simulink model "RB_KAIROS_ArmOnly"  (R2020b)
(part 6 of 17)

t15918 = ((t9.*(t16.*(t30.*(t2425-t2468)+t68.*(t2425-t2468))+t8.*(t7.*(t4650+t34.*(t2425-t2468))+t47.*(t2425-t2468))).*7.35522e-1+t17.*(t4654+t15.*(t4650+t34.*(t2425-t2468))).*7.35522e-1).*(t1987-t2621+t3452+t11654+t9.*(t71-t391).*6.1597e-2+t17.*(t426-t581)+t9.*(t9166-t11658)))./4.0;
t15980 = ((t9.*(t16.*(t30.*(t2425-t2468)+t68.*(t2425-t2468))+t8.*(t7.*(t4650+t34.*(t2425-t2468))+t47.*(t2425-t2468)))+t17.*(t4654+t15.*(t4650+t34.*(t2425-t2468)))).*(t3418-t3879+t4324+t11855+t9.*(t71-t391).*4.5305948634e-2+t17.*(t426-t581).*7.35522e-1+t9.*(t9166-t11658).*7.35522e-1))./4.0;
t16008 = t5405+t5427+t5511+t6027+t6161+t8970+t8992+t9123+t9124+t9143+t9812;
t16084 = ((t2148+t2513+t2649+t2661+t3582+t11950+t17.*(t258+t2289+t5392+t7559)).*(t3418-t3879+t4324+t11855+t9.*(t71-t391).*4.5305948634e-2+t17.*(t426-t581).*7.35522e-1+t9.*(t9166-t11658).*7.35522e-1))./2.0;
t16096 = t14770.*(t3418-t3879+t4324+t11855+t9.*(t71-t391).*4.5305948634e-2+t17.*(t426-t581).*7.35522e-1+t9.*(t9166-t11658).*7.35522e-1).*(-1.0./2.0);
t16098 = t14821.*(t3418-t3879+t4324+t11855+t9.*(t71-t391).*4.5305948634e-2+t17.*(t426-t581).*7.35522e-1+t9.*(t9166-t11658).*7.35522e-1).*(-1.0./2.0);
t16101 = (t14821.*(t3418-t3879+t4324+t11855+t9.*(t71-t391).*4.5305948634e-2+t17.*(t426-t581).*7.35522e-1+t9.*(t9166-t11658).*7.35522e-1))./2.0;
t16102 = t15155.*(t1987-t2621+t3452+t11654+t9.*(t71-t391).*6.1597e-2+t17.*(t426-t581)+t9.*(t9166-t11658)).*(-1.0./2.0);
t16103 = (t15155.*(t1987-t2621+t3452+t11654+t9.*(t71-t391).*6.1597e-2+t17.*(t426-t581)+t9.*(t9166-t11658)))./2.0;
t16113 = t3191+t3236+t3713+t3776+t3783+t3799+t3859+t3869+t3956+t4124+t4167+t4189+t5302+t5350+t5730+t5737+t5835+t5903+t6355+t6376+t7335+t7337+t7624+t7699+t8153+t8325+t8326+t9141;
t16114 = q4d.*t16112;
t16116 = q4d.*t16115;
t16117 = t2870+t2974+t3039+t3190+t3194+t3235+t3795+t3999+t4020+t4097+t4102+t4129+t4150+t4188+t4835+t4914+t5310+t5373+t5382+t5862+t5987+t6897+t6956+t7263+t7271+t7272+t7672+t8100+t8116+t8118+t8495+t8498+t9163;
t16119 = t2976+t3040+t3143+t3150+t3229+t3252+t3795+t3999+t4020+t4073+t4079+t4117+t4162+t4221+t4835+t4914+t5310+t5373+t5382+t5862+t5987+t6897+t6956+t7263+t7271+t7272+t7672+t8100+t8116+t8118+t8495+t8498+t9163;
t16126 = q4d.*t16125;
t16150 = t3018+t3019+t3656+t3665+t3675+t3695+t3698+t3717+t3730+t3731+t3800+t3981+t4084+t4092+t4145+t4644+t4690+t4718+t4739+t4745+t4760+t4775+t4780+t4781+t4782+t4851+t4864+t4887+t5324+t5327+t5565+t5601+t5850+t5874+t5910+t5920+t5986+t6084+t6085+t6180+t6191+t6243+t6506+t6558+t6561+t6580+t7154+t7178+t7233+t7543+t7562+t7668+t7867+t7869+t7983+t8096+t8111+t8854+t8872+t8948+t9161;
t16151 = t2953+t3140+t3656+t3675+t3692+t3695+t3698+t3717+t3730+t3731+t3830+t3957+t4105+t4110+t4120+t4644+t4690+t4718+t4739+t4745+t4760+t4775+t4780+t4781+t4782+t4851+t4864+t4887+t5324+t5327+t5565+t5601+t5836+t5874+t5910+t5944+t5986+t6084+t6085+t6174+t6195+t6243+t6506+t6558+t6561+t6580+t7154+t7178+t7233+t7543+t7562+t7668+t7867+t7869+t7970+t8095+t8112+t8854+t8872+t8942+t9161;
t5197 = -t5186;
t5267 = -t5253;
t5765 = -t5749;
t5803 = -t5791;
t5811 = -t5798;
t5815 = -t5802;
t5846 = -t5830;
t6345 = -t6326;
t6404 = -t6390;
t6420 = -t6411;
t6620 = -t6610;
t6944 = -t6919;
t7029 = -t7008;
t7082 = -t7069;
t7123 = -t7114;
t7204 = -t7195;
t7229 = -t7213;
t7270 = -t7258;
t7407 = -t7394;
t7425 = -t7413;
t7508 = -t7495;
t7583 = -t7568;
t7588 = -t7572;
t7594 = t7.*t7568;
t7597 = t7.*t7572;
t7610 = -t7595;
t7619 = -t7599;
t7650 = -t7631;
t7662 = -t7647;
t7723 = -t7706;
t7754 = -t7742;
t7765 = -t7756;
t7775 = -t7762;
t7783 = -t7768;
t7784 = -t7769;
t7802 = t321.*t7568;
t7812 = t321.*t7572;
t7824 = -t7809;
t7825 = -t7810;
t7850 = -t7836;
t7899 = -t7880;
t7921 = -t7911;
t7946 = -t7931;
t7986 = -t7972;
t8094 = -t8074;
t8167 = -t8154;
t8365 = -t8354;
t8408 = -t8395;
t8493 = -t8481;
t8618 = -t8614;
t8624 = t8.*t8614;
t8632 = -t8626;
t8645 = -t8637;
t8671 = -t8666;
t8676 = t8.*t8666;
t8682 = -t8677;
t8685 = -t8679;
t8686 = -t8680;
t8691 = -t8687;
t8694 = t323.*t8614;
t8714 = -t8707;
t8735 = -t8729;
t8736 = -t8730;
t8739 = -t8733;
t8743 = t1992+t2480+t2616+t3584+t5408;
t8753 = t323.*t8666;
t8758 = t439.*t8614;
t8761 = -t8752;
t8789 = -t8774;
t8795 = -t8781;
t8827 = -t8807;
t8834 = -t8815;
t8866 = -t8847;
t8885 = t439.*t8666;
t8904 = -t8881;
t8912 = -t8887;
t8916 = -t8895;
t8932 = -t8924;
t8935 = -t8926;
t8944 = -t8936;
t8955 = -t8943;
t8965 = -t8953;
t9004 = -t9000;
t9007 = -t9003;
t9021 = -t9017;
t9030 = -t9025;
t9040 = -t9037;
t9057 = -t9051;
t9073 = -t9066;
t9074 = -t9067;
t9080 = -t9070;
t9094 = -t9089;
t9109 = -t9097;
t9153 = -t9148;
t9186 = -t9180;
t9199 = -t9193;
t9208 = -t9203;
t9210 = -t9204;
t9227 = -t9220;
t9235 = -t9222;
t9237 = -t9223;
t9257 = (t3421.*t8654)./4.0;
t9259 = (t3489.*t8654)./4.0;
t9292 = t2497+t2680+t3516+t4728+t5360;
t9293 = t2500+t2647+t3521+t4730+t5385;
t9334 = -t9324;
t9355 = -t9344;
t9357 = -t9345;
t9358 = -t9346;
t9487 = -t9479;
t9506 = -t9497;
t9530 = t17.*t9194.*1.539925e-2;
t9544 = -t9532;
t9563 = t9256.*1.666555;
t9565 = t9256.*7.35522e-1;
t9567 = t9254.*1.666555;
t9642 = -t9634;
t9652 = (t2044.*t9194)./4.0;
t9703 = -t9695;
t9706 = -t9697;
t9707 = -t9699;
t9719 = -t9709;
t9721 = -t9711;
t9729 = -t9718;
t9784 = t9256.*5.01208083475e-2;
t9796 = -t9783;
t9802 = -t9789;
t9809 = t9254.*1.17633784675e-2;
t9814 = -t9800;
t9819 = -t9808;
t9843 = -t9834;
t9850 = -t9841;
t9866 = -t9856;
t9922 = t3378+t3817+t3882+t4359+t5832;
t9928 = -t9923;
t9930 = (t3763.*t9194)./4.0;
t9948 = -t9942;
t9961 = -t9956;
t9963 = -t9958;
t9998 = -t9990;
t10007 = t8.*t9743.*2.62925e-3;
t10009 = t8.*t9744.*2.62925e-3;
t10026 = -t10018;
t10031 = -t10022;
t10032 = -t10023;
t10043 = -t10029;
t10118 = (t5433.*t8725)./4.0;
t10127 = -t10122;
t10131 = -t10125;
t10133 = (t5696.*t8654)./4.0;
t10134 = -t10128;
t10135 = (t4474.*t9194)./4.0;
t10140 = -t10136;
t10158 = t8.*t10147;
t10159 = t9.*t10147;
t10160 = t16.*t10147;
t10161 = t17.*t10147;
t10167 = -t10163;
t10173 = t9.*t10153;
t10174 = t17.*t10153;
t10179 = (t2501.*t9744)./4.0;
t10190 = (t4798.*t9194)./4.0;
t10207 = -t10188;
t10221 = -t10213;
t10227 = -t10222;
t10243 = -t10239;
t10256 = -t10247;
t10296 = -t10290;
t10297 = -t10291;
t10351 = -t10342;
t10370 = (t3732.*t9744)./4.0;
t10374 = -t10365;
t10387 = (t5213.*t9194)./4.0;
t10388 = (t6302.*t8654)./4.0;
t10389 = -t10371;
t10390 = -t10372;
t10412 = t10188.*7.35522e-1;
t10413 = t10189.*7.35522e-1;
t10414 = t10191.*7.35522e-1;
t10415 = t10192.*7.35522e-1;
t10418 = t10188.*1.666555;
t10419 = t10191.*1.666555;
t10428 = -t10420;
t10431 = -t10421;
t10438 = t10203.*7.35522e-1;
t10439 = t10204.*7.35522e-1;
t10445 = t8.*t10436;
t10446 = t3845+t3925+t4339+t5224+t5804;
t10463 = (t4024.*t9743)./4.0;
t10464 = -t10456;
t10486 = -t10481;
t10491 = t2711+t3823+t3943+t3991+t5204+t5257;
t10499 = -t10497;
t10525 = -t10517;
t10546 = t6863+t8519;
t10549 = (t4489.*t9744)./4.0;
t10550 = t6855+t8515;
t10552 = (t4498.*t9744)./4.0;
t10554 = t6889+t8505;
t10561 = t6885+t8517;
t10593 = t7.*t10147.*1.059103943995e-1;
t10602 = t16.*t10153.*5.01208083475e-2;
t10604 = (t5679.*t9194)./2.0;
t10607 = t6838+t8605;
t10608 = t8.*t10153.*1.17633784675e-2;
t10611 = t15.*t10153.*1.059103943995e-1;
t10612 = t6831+t8599;
t10620 = t10189.*3.867742437e-3;
t10622 = t10191.*5.01208083475e-2;
t10624 = -t10616;
t10627 = t10188.*1.17633784675e-2;
t10628 = t9.*t10170.*1.13264871585e-2;
t10630 = t10192.*1.563719772e-3;
t10643 = -t10632;
t10644 = t10204.*3.867742437e-3;
t10645 = t17.*t10180.*1.13264871585e-2;
t10661 = t10203.*1.563719772e-3;
t10679 = -t10656;
t10681 = -t10660;
t10688 = t16.*t10199.*4.38178973375e-3;
t10702 = (t5782.*t9194)./2.0;
t10708 = t17.*(t4324-t5228+t5802+t9.*(t71-t391).*4.5305948634e-2+t17.*(t426-t581).*7.35522e-1).*(-1.539925e-2);
t10718 = t17.*(t4324-t5228+t5802+t9.*(t71-t391).*4.5305948634e-2+t17.*(t426-t581).*7.35522e-1).*1.539925e-2;
t10723 = -t10713;
t10733 = -t10728;
t10734 = -t10730;
t10736 = -t10731;
t10745 = t9.*t10480.*1.539925e-2;
t10748 = t17.*t10485.*1.539925e-2;
t10772 = (t5007.*t9744)./4.0;
t10773 = -t10771;
t10776 = (t6016.*t9194)./2.0;
t10780 = -t10777;
t10786 = -t10784;
t10791 = -t10788;
t10796 = -t10789;
t10809 = -t10803;
t10811 = -t10806;
t10815 = -t10814;
t10819 = (t5235.*t9743)./4.0;
t10828 = t8.*t10597.*2.62925e-3;
t10830 = -t10827;
t10834 = t7.*t10577.*8.639075e-2;
t10877 = t16.*t3489.*t10153.*1.838805e-1;
t10889 = -t10885;
t10895 = t1728+t2213+t3231+t3940+t3941+t4346+t4371+t5207;
t10915 = -t10907;
t10933 = -t10923;
t10935 = -t10929;
t10938 = t9.*t10920;
t10939 = t17.*t10920;
t10942 = t6474+t9254;
t10945 = (t6540.*t9194)./2.0;
t10956 = t6502+t9256;
t10967 = t3743.*(t4324-t5228+t5802+t9.*(t71-t391).*4.5305948634e-2+t17.*(t426-t581).*7.35522e-1).*(-1.0./4.0);
t10971 = -t10961;
t10979 = (t3743.*(t4324-t5228+t5802+t9.*(t71-t391).*4.5305948634e-2+t17.*(t426-t581).*7.35522e-1))./4.0;
t10981 = -t10969;
t10982 = -t10970;
t10997 = t16.*t4021.*t10153.*4.1663875e-1;
t10998 = t8.*t4024.*t10153.*4.1663875e-1;
t10999 = -t10991;
t11002 = -t10994;
t11003 = -t10995;
t11005 = -t10988;
t11016 = -t11010;
t11018 = -t11013;
t11021 = (t3738.*t10480)./4.0;
t11026 = (t3743.*t10485)./4.0;
t11030 = (t2966.*t10577)./4.0;
t11032 = (t4884.*t10153)./4.0;
t11037 = -t11031;
t11038 = (t4900.*t10153)./4.0;
t11052 = (t4939.*t10153)./4.0;
t11083 = (t10199.*(t2904-t2927))./4.0;
t11104 = (t5929.*t9744)./4.0;
t11109 = (t5947.*t9744)./4.0;
t11113 = (t5951.*t9744)./4.0;
t11122 = (t3752.*t10586)./4.0;
t11123 = (t7797.*t8725)./4.0;
t11131 = (t5216.*t10147)./4.0;
t11137 = -t11126;
t11145 = (t5218.*t10153)./4.0;
t11148 = -t11141;
t11172 = -t11163;
t11173 = t10988.*7.35522e-1;
t11174 = t10990.*7.35522e-1;
t11187 = t11006.*7.35522e-1;
t11188 = t11008.*7.35522e-1;
t11198 = (t4035.*t10577)./4.0;
t11200 = -t11196;
t11201 = (t4024.*t10597)./4.0;
t11218 = (t8191.*t8654)./4.0;
t11223 = -t11219;
t11242 = -t11236;
t11243 = (t16.*t5365.*t10153)./4.0;
t11246 = (t4255.*t10577)./4.0;
t11248 = (t4286.*t10577)./4.0;
t11252 = -t11245;
t11270 = (t5443.*t10147)./4.0;
t11271 = -t11261;
t11281 = (t5365.*t10199)./4.0;
t11284 = (t5442.*t10153)./4.0;
t11286 = (t5443.*t10153)./4.0;
t11292 = -t11283;
t11302 = (t5434.*t10170)./4.0;
t11304 = -t11297;
t11308 = -t11303;
t11310 = (t5433.*t10180)./4.0;
t11323 = -t11313;
t11329 = -t11319;
t11337 = -t11332;
t11338 = t8518+t8558;
t11340 = t8512+t8568;
t11341 = t8516+t8571;
t11342 = -t11339;
t11351 = (t5635.*t10147)./4.0;
t11352 = t9194.*(t1468-t1988-t2498+t4565+t17.*(t208-t427)).*(-1.0./4.0);
t11357 = (t9194.*(t1468-t1988-t2498+t4565+t17.*(t208-t427)))./4.0;
t11360 = t8.*t10920.*4.38178973375e-3;
t11367 = (t5646.*t10153)./4.0;
t11368 = t16.*t5234.*t10153.*4.1663875e-1;
t11369 = t8.*t5235.*t10153.*4.1663875e-1;
t11372 = t6910+t9566;
t11376 = t16.*t10936.*4.38178973375e-3;
t11377 = t6927+t9564;
t11380 = t6934+t9562;
t11382 = -t11373;
t11386 = -t11378;
t11387 = -t11379;
t11396 = t8586+t8603;
t11400 = t8592+t8608;
t11407 = t10990.*3.867742437e-3;
t11415 = t10988.*1.563719772e-3;
t11416 = t16.*(t6472-t9256).*(-4.38178973375e-3);
t11420 = -t11410;
t11421 = -t11411;
t11424 = t11008.*3.867742437e-3;
t11428 = t16.*t10973.*4.38178973375e-3;
t11429 = t11006.*1.563719772e-3;
t11430 = -t11423;
t11432 = -t11427;
t11440 = -t11434;
t11441 = -t11435;
t11443 = (t4849.*t10577)./4.0;
t11444 = -t11438;
t11451 = -t11448;
t11453 = -t11449;
t11468 = t5345.*(t4324-t5228+t5802+t9.*(t71-t391).*4.5305948634e-2+t17.*(t426-t581).*7.35522e-1).*(-1.0./4.0);
t11472 = (t5345.*(t4324-t5228+t5802+t9.*(t71-t391).*4.5305948634e-2+t17.*(t426-t581).*7.35522e-1))./4.0;
t11477 = (t6729.*t9744)./2.0;
t11484 = t3471+t3796+t3914+t3942+t4358+t5220+t5842;
t11488 = (t5064.*t10577)./4.0;
t11490 = (t5329.*t10480)./4.0;
t11495 = (t5345.*t10485)./4.0;
t11499 = -t11492;
t11508 = (t7799.*t9194)./4.0;
t11511 = (t8.*t6046.*t10153)./4.0;
t11517 = (t16.*t6069.*t10153)./4.0;
t11525 = t9744.*(-t1540+t2091+t2579+t8.*(t260+t468+t570+t2298)).*(-1.0./2.0);
t11531 = (t6175.*t10147)./4.0;
t11532 = (t9744.*(-t1540+t2091+t2579+t8.*(t260+t468+t570+t2298)))./2.0;
t11541 = (t6196.*t10147)./4.0;
t11543 = (t6069.*t10199)./4.0;
t11545 = (t6175.*t10153)./4.0;
t11550 = t16.*t5696.*t10153.*1.838805e-1;
t11552 = (t6995.*t9744)./2.0;
t11553 = (t5235.*t10597)./4.0;
t11557 = (t6196.*t10153)./4.0;
t11567 = -t11555;
t11578 = -t11566;
t11583 = -t11574;
t11585 = (t7949.*t9194)./4.0;
t11588 = -t11580;
t11589 = -t11582;
t11597 = -t11590;
t11598 = t8.*t11390.*2.62925e-3;
t11600 = (t7066.*t9744)./4.0;
t11608 = (t7987.*t9194)./4.0;
t11612 = -t11607;
t11632 = -t11625;
t11636 = -t11631;
t11641 = (t6385.*t10153)./4.0;
t11644 = -t11637;
t11646 = -t11638;
t11682 = -t11680;
t11686 = -t11684;
t11694 = t17.*(t3418-t3879+t4324-t5228+t5802+t9.*(t71-t391).*4.5305948634e-2+t17.*(t426-t581).*7.35522e-1).*(-1.539925e-2);
t11696 = -t11689;
t11702 = t17.*(t3418-t3879+t4324-t5228+t5802+t9.*(t71-t391).*4.5305948634e-2+t17.*(t426-t581).*7.35522e-1).*1.539925e-2;
t11717 = t9.*t11483.*1.539925e-2;
t11740 = (t6552.*t10147)./4.0;
t11743 = (t5613.*t10577)./4.0;
t11748 = (t5634.*t10577)./4.0;
t11749 = (t6546.*t10153)./4.0;
t11754 = (t5628.*t10577)./4.0;
t11770 = (t7402.*t9744)./2.0;
t11783 = -t11771;
t11789 = (t5699.*t10586)./4.0;
t11807 = -t11795;
t11827 = t2044.*(t3418-t3879+t4324-t5228+t5802+t9.*(t71-t391).*4.5305948634e-2+t17.*(t426-t581).*7.35522e-1).*(-1.0./4.0);
t11831 = t16.*t6302.*t10153.*1.838805e-1;
t11832 = (t2044.*(t3418-t3879+t4324-t5228+t5802+t9.*(t71-t391).*4.5305948634e-2+t17.*(t426-t581).*7.35522e-1))./4.0;
t11836 = (t10936.*(t2904-t2927))./4.0;
t11838 = (t5806.*t10577)./4.0;
t11843 = t10577.*(t495+t572+t1838+t2069+t2107).*(-1.0./4.0);
t11850 = (t2904-t2927).*(t6472-t9256).*(-1.0./4.0);
t11869 = (t10973.*(t2904-t2927))./4.0;
t11888 = (t5928.*t10577)./4.0;
t11900 = (t16.*t6884.*t10153)./4.0;
t11901 = (t8.*t6872.*t10153)./4.0;
t11904 = (t6969.*t10153)./4.0;
t11908 = -t11906;
t11913 = (t6884.*t10199)./4.0;
t11926 = -t11919;
t11927 = -t11920;
t11939 = (t7113.*t10147)./4.0;
t11954 = (t7124.*t10153)./4.0;
t11963 = -t11955;
t11967 = t8654.*(t249-t391.*(1.1e+1./1.25e+2)-t1912.*4.252e-3+t3505+t5357+t693.*(t71-t391)+t784.*(t71-t391)).*(-1.0./2.0);
t11968 = t8654.*(t249-t391.*(1.1e+1./1.25e+2)-t1912.*4.252e-3+t3505+t5357+t693.*(t71-t391)+t784.*(t71-t391)).*(-1.0./4.0);
t11971 = -t11958;
t11974 = (t5365.*t10936)./4.0;
t11975 = (t8654.*(t249-t391.*(1.1e+1./1.25e+2)-t1912.*4.252e-3+t3505+t5357+t693.*(t71-t391)+t784.*(t71-t391)))./2.0;
t11976 = (t8654.*(t249-t391.*(1.1e+1./1.25e+2)-t1912.*4.252e-3+t3505+t5357+t693.*(t71-t391)+t784.*(t71-t391)))./4.0;
t11977 = -t11972;
t11978 = (t8725.*t9185)./4.0;
t11987 = t5365.*(t6472-t9256).*(-1.0./4.0);
t11990 = (t5365.*(t6472-t9256))./4.0;
t11995 = (t5365.*t10973)./4.0;
t11996 = t3763.*(t3418-t3879+t4324-t5228+t5802+t9.*(t71-t391).*4.5305948634e-2+t17.*(t426-t581).*7.35522e-1).*(-1.0./4.0);
t12000 = (t3763.*(t3418-t3879+t4324-t5228+t5802+t9.*(t71-t391).*4.5305948634e-2+t17.*(t426-t581).*7.35522e-1))./4.0;
t12001 = (t3738.*t11483)./4.0;
t12005 = (t7217.*t10153)./4.0;
t12032 = (t8178.*t9744)./2.0;
t12035 = t6761.*(t4324-t5228+t5802+t9.*(t71-t391).*4.5305948634e-2+t17.*(t426-t581).*7.35522e-1).*(-1.0./4.0);
t12040 = (t6761.*(t4324-t5228+t5802+t9.*(t71-t391).*4.5305948634e-2+t17.*(t426-t581).*7.35522e-1))./4.0;
t12041 = t9743.*(-t1476-t1540+t2091+t2165+t2579+t8.*(t260+t468+t570+t2298)).*(-1.0./2.0);
t12045 = (t9743.*(-t1476-t1540+t2091+t2165+t2579+t8.*(t260+t468+t570+t2298)))./2.0;
t12061 = t16.*t7079.*t10153.*4.1663875e-1;
t12064 = (t6589.*t10586)./4.0;
t12070 = t8.*t7116.*t10153.*4.1663875e-1;
t12089 = t4474.*(t3418-t3879+t4324-t5228+t5802+t9.*(t71-t391).*4.5305948634e-2+t17.*(t426-t581).*7.35522e-1).*(-1.0./4.0);
t12092 = (t4474.*(t3418-t3879+t4324-t5228+t5802+t9.*(t71-t391).*4.5305948634e-2+t17.*(t426-t581).*7.35522e-1))./4.0;
t12093 = -t12090;
t12105 = (t7676.*t10153)./4.0;
t12120 = t4798.*(t3418-t3879+t4324-t5228+t5802+t9.*(t71-t391).*4.5305948634e-2+t17.*(t426-t581).*7.35522e-1).*(-1.0./4.0);
t12123 = (t4798.*(t3418-t3879+t4324-t5228+t5802+t9.*(t71-t391).*4.5305948634e-2+t17.*(t426-t581).*7.35522e-1))./4.0;
t12128 = -t12124;
t12139 = -t12133;
t12142 = (t7815.*t10153)./4.0;
t12144 = -t12138;
t12145 = (t7796.*t10170)./4.0;
t12147 = t6069.*(t6472-t9256).*(-1.0./4.0);
t12148 = -t12140;
t12152 = (t7797.*t10180)./4.0;
t12154 = (t6069.*(t6472-t9256))./4.0;
t12155 = (t6967.*t10577)./4.0;
t12160 = (t6069.*t10973)./4.0;
t12161 = (t10577.*(t921+t1317-t5853))./4.0;
t12176 = (t7039.*t10577)./4.0;
t12179 = t10147.*(t2437+t2648+t3129+t3384+t3574).*(-1.0./4.0);
t12180 = (t5235.*t11390)./4.0;
t12186 = -t12178;
t12192 = (t7937.*t10153)./4.0;
t12206 = t9194.*(t824+t2543+t2699+t2707-t4767+t17.*(t260+t468+t570+t2298)).*(-1.0./4.0);
t12213 = (t9194.*(t824+t2543+t2699+t2707-t4767+t17.*(t260+t468+t570+t2298)))./4.0;
t12229 = (t9187.*t9194)./4.0;
t12231 = (t8044.*t10147)./4.0;
t12232 = -t12227;
t12234 = (t8047.*t10147)./4.0;
t12235 = (t8050.*t10147)./4.0;
t12238 = (t8054.*t10147)./4.0;
t12239 = -t12233;
t12241 = -t12237;
t12244 = (t8050.*t10153)./4.0;
t12245 = (t8053.*t10153)./4.0;
t12247 = (t8054.*t10153)./4.0;
t12254 = -t12248;
t12255 = (t8065.*t10153)./4.0;
t12259 = (t10153.*(t917-t1669+t2469+t2475+t3495+t3591))./4.0;
t12265 = -t12261;
t12268 = -t12263;
t12284 = t5213.*(t3418-t3879+t4324-t5228+t5802+t9.*(t71-t391).*4.5305948634e-2+t17.*(t426-t581).*7.35522e-1).*(-1.0./4.0);
t12290 = (t5213.*(t3418-t3879+t4324-t5228+t5802+t9.*(t71-t391).*4.5305948634e-2+t17.*(t426-t581).*7.35522e-1))./4.0;
t12293 = (t8256.*t10147)./4.0;
t12296 = t8189+t10191;
t12303 = (t8285.*t10147)./4.0;
t12306 = (t8256.*t10153)./4.0;
t12322 = -t12314;
t12324 = -t12315;
t12328 = -t12318;
t12331 = -t12326;
t12338 = (t8310.*t10153)./4.0;
t12339 = t8270+t10203;
t12347 = t8292+t10204;
t12352 = (t5329.*t11483)./4.0;
t12393 = (t16.*t8477.*t10153)./4.0;
t12395 = -t12391;
t12402 = -t12399;
t12403 = -t12400;
t12408 = (t6872.*t10920)./4.0;
t12411 = (t8477.*t10199)./4.0;
t12412 = t16.*t8191.*t10153.*1.838805e-1;
t12416 = (t6884.*t10936)./4.0;
t12417 = t5679.*(t3418-t3879+t4324-t5228+t5802+t9.*(t71-t391).*4.5305948634e-2+t17.*(t426-t581).*7.35522e-1).*(-1.0./4.0);
t12420 = t16.*t8227.*t10153.*4.1663875e-1;
t12421 = (t5679.*(t3418-t3879+t4324-t5228+t5802+t9.*(t71-t391).*4.5305948634e-2+t17.*(t426-t581).*7.35522e-1))./4.0;
t12422 = (t10153.*(t2433+t2449-t3048-t3102+t3223+t3232))./4.0;
t12423 = t8.*t10153.*(-t1476-t1540+t2091+t2165+t2579+t8.*(t260+t468+t570+t2298)).*(-4.1663875e-1);
t12441 = (t7822.*t10586)./4.0;
t12448 = t5782.*(t3418-t3879+t4324-t5228+t5802+t9.*(t71-t391).*4.5305948634e-2+t17.*(t426-t581).*7.35522e-1).*(-1.0./4.0);
t12449 = (t16.*t8640.*t10153)./4.0;
t12452 = (t5782.*(t3418-t3879+t4324-t5228+t5802+t9.*(t71-t391).*4.5305948634e-2+t17.*(t426-t581).*7.35522e-1))./4.0;
t12463 = (t8640.*t10199)./4.0;
t12475 = t6016.*(t3418-t3879+t4324-t5228+t5802+t9.*(t71-t391).*4.5305948634e-2+t17.*(t426-t581).*7.35522e-1).*(-1.0./4.0);
t12477 = (t6016.*(t3418-t3879+t4324-t5228+t5802+t9.*(t71-t391).*4.5305948634e-2+t17.*(t426-t581).*7.35522e-1))./4.0;
t12492 = (t8791.*t10153)./4.0;
t12512 = t10597.*(-t1476-t1540+t2091+t2165+t2579+t8.*(t260+t468+t570+t2298)).*(-1.0./4.0);
t12517 = (t10597.*(-t1476-t1540+t2091+t2165+t2579+t8.*(t260+t468+t570+t2298)))./4.0;
t12537 = t17.*(t8266-t10204).*(-1.13264871585e-2);
t12546 = -t12545;
t12575 = t6540.*(t3418-t3879+t4324-t5228+t5802+t9.*(t71-t391).*4.5305948634e-2+t17.*(t426-t581).*7.35522e-1).*(-1.0./4.0);
t12584 = (t6540.*(t3418-t3879+t4324-t5228+t5802+t9.*(t71-t391).*4.5305948634e-2+t17.*(t426-t581).*7.35522e-1))./4.0;
t12586 = -t12576;
t12587 = -t12577;
t12594 = (t8725.*t10469)./4.0;
t12605 = (t9104.*t10153)./4.0;
t12612 = (t16.*t9110.*t10153)./4.0;
t12613 = (t8.*t9112.*t10153)./4.0;
t12643 = t8981.*(t4324-t5228+t5802+t9.*(t71-t391).*4.5305948634e-2+t17.*(t426-t581).*7.35522e-1).*(-1.0./4.0);
t12645 = (t8981.*(t4324-t5228+t5802+t9.*(t71-t391).*4.5305948634e-2+t17.*(t426-t581).*7.35522e-1))./4.0;
t12647 = (t7116.*t11390)./4.0;
t12651 = (t9209.*t10147)./4.0;
t12657 = (t10147.*(t2810+t2988-t7937))./4.0;
t12658 = (t9185.*t10180)./4.0;
t12659 = (t8979.*t10480)./2.0;
t12660 = (t6811.*t11483)./4.0;
t12661 = (t9194.*t10170)./4.0;
t12665 = -t12655;
t12674 = -t12662;
t12675 = (t9216.*t10153)./4.0;
t12676 = (t9236.*t10147)./4.0;
t12677 = (t10153.*(t2810+t2988-t7937))./4.0;
t12678 = -t12671;
t12680 = (t8981.*t10485)./2.0;
t12685 = (t9236.*t10153)./4.0;
t12694 = -t12686;
t12713 = (t9278.*t10147)./4.0;
t12721 = (t9278.*t10153)./4.0;
t12733 = -t12728;
t12738 = t8224+t11006;
t12741 = (t9333.*t10153)./4.0;
t12744 = t8255+t11008;
t12811 = (t9525.*t10153)./4.0;
t12819 = t8477.*(t6472-t9256).*(-1.0./4.0);
t12821 = ((t1468-t1988-t2498+t4565+t17.*(t208-t427)).*(t3418-t3879+t4324-t5228+t5802+t9.*(t71-t391).*4.5305948634e-2+t17.*(t426-t581).*7.35522e-1))./4.0;
t12822 = (t8477.*(t6472-t9256))./4.0;
t12827 = (t8477.*t10973)./4.0;
t12835 = t16.*t10153.*(t249-t391.*(1.1e+1./1.25e+2)-t1912.*4.252e-3+t3505+t5357+t693.*(t71-t391)+t784.*(t71-t391)).*(-1.838805e-1);
t12838 = -t12833;
t12839 = -t12834;
t12857 = -t12848;
t12858 = -t12849;
t12867 = t1999+t2168+t2188+t12349;
t12870 = (t8640.*t10936)./4.0;
t12937 = -t12934;
t12940 = t7799.*(t3418-t3879+t4324-t5228+t5802+t9.*(t71-t391).*4.5305948634e-2+t17.*(t426-t581).*7.35522e-1).*(-1.0./4.0);
t12946 = (t7799.*(t3418-t3879+t4324-t5228+t5802+t9.*(t71-t391).*4.5305948634e-2+t17.*(t426-t581).*7.35522e-1))./4.0;
t12947 = (t16.*t9744.*t10153)./4.0;
t12951 = t8.*t10153.*(-t3045-t3218+t3458+t3539+t3878+t8.*(t260+t468+t570+t2298).*1.666555).*(-1.0./4.0);
t12962 = t5433.*(t8266-t10204).*(-1.0./4.0);
t12967 = (t5433.*(t8266-t10204))./4.0;
t12970 = t16.*t9744.*(t6452-t8229).*(-1.0./4.0);
t12973 = (t9744.*t10199)./4.0;
t12980 = -t12976;
t12988 = t7949.*(t3418-t3879+t4324-t5228+t5802+t9.*(t71-t391).*4.5305948634e-2+t17.*(t426-t581).*7.35522e-1).*(-1.0./4.0);
t12993 = t11390.*(-t1476-t1540+t2091+t2165+t2579+t8.*(t260+t468+t570+t2298)).*(-1.0./4.0);
t12998 = (t11390.*(-t1476-t1540+t2091+t2165+t2579+t8.*(t260+t468+t570+t2298)))./4.0;
t13001 = t7987.*(t3418-t3879+t4324-t5228+t5802+t9.*(t71-t391).*4.5305948634e-2+t17.*(t426-t581).*7.35522e-1).*(-1.0./4.0);
t13008 = (t7987.*(t3418-t3879+t4324-t5228+t5802+t9.*(t71-t391).*4.5305948634e-2+t17.*(t426-t581).*7.35522e-1))./4.0;
t13010 = t9744.*(t8315+t8.*(t30.*(t2425-t2468)+t68.*(t2425-t2468))).*(-1.0./4.0);
t13012 = (t9744.*(t8315+t8.*(t30.*(t2425-t2468)+t68.*(t2425-t2468))))./4.0;
t13014 = t17.*(t8221-t11008).*(-1.13264871585e-2);
t13026 = t9.*t13013;
t13027 = t17.*t13013;
t13055 = (t9967.*t10147)./4.0;
t13065 = (t9967.*t10153)./4.0;
t13077 = -t13074;
t13079 = (t9992.*t10153)./4.0;
t13107 = (t9112.*t10920)./4.0;
t13114 = -t13108;
t13115 = (t9110.*t10936)./4.0;
t13123 = -t13118;
t13126 = -t13121;
t13127 = t9110.*(t6472-t9256).*(-1.0./4.0);
t13133 = (t9110.*t10973)./4.0;
t13139 = -t13136;
t13153 = (t16.*t10141.*t10153)./4.0;
t13159 = -t13157;
t13177 = t9244+t10990;
t13182 = t10189+t10217;
t13189 = t10192+t10232;
t13196 = t9140+t11149;
t13197 = t9144+t11144;
t13198 = t9147+t11147;
t13205 = -t13202;
t13207 = t16.*t13005.*4.38178973375e-3;
t13213 = t8.*t13013.*4.38178973375e-3;
t13223 = -t13221;
t13296 = t10480.*(t1987-t2621+t3452-t4730+t5359+t9.*(t71-t391).*6.1597e-2+t17.*(t426-t581)).*(-1.0./4.0);
t13297 = t8999.*(t3418-t3879+t4324-t5228+t5802+t9.*(t71-t391).*4.5305948634e-2+t17.*(t426-t581).*7.35522e-1).*(-1.0./4.0);
t13342 = t10920.*(-t3045-t3218+t3458+t3539+t3878+t8.*(t260+t468+t570+t2298).*1.666555).*(-1.0./4.0);
t13348 = (t10920.*(-t3045-t3218+t3458+t3539+t3878+t8.*(t260+t468+t570+t2298).*1.666555))./4.0;
t13359 = (t9744.*t10936)./4.0;
t13372 = t9744.*(t6472-t9256).*(-1.0./4.0);
t13374 = t5433.*(t8221-t11008).*(-1.0./4.0);
t13378 = (t5433.*(t8221-t11008))./4.0;
t13380 = t3414+t3525+t3532+t9320+t9761;
t13383 = (t9744.*t10973)./4.0;
t13390 = t9744.*(t8219-t8226).*(-1.0./4.0);
t13407 = ((t824+t2543+t2699+t2707-t4767+t17.*(t260+t468+t570+t2298)).*(t3418-t3879+t4324-t5228+t5802+t9.*(t71-t391).*4.5305948634e-2+t17.*(t426-t581).*7.35522e-1))./2.0;
t13411 = t9187.*(t3418-t3879+t4324-t5228+t5802+t9.*(t71-t391).*4.5305948634e-2+t17.*(t426-t581).*7.35522e-1).*(-1.0./2.0);
t13412 = -t13410;
t13413 = (t9187.*(t3418-t3879+t4324-t5228+t5802+t9.*(t71-t391).*4.5305948634e-2+t17.*(t426-t581).*7.35522e-1))./2.0;
t13423 = -t13420;
t13441 = t9252.*(t3418-t3879+t4324-t5228+t5802+t9.*(t71-t391).*4.5305948634e-2+t17.*(t426-t581).*7.35522e-1).*(-1.0./2.0);
t13445 = (t9252.*(t3418-t3879+t4324-t5228+t5802+t9.*(t71-t391).*4.5305948634e-2+t17.*(t426-t581).*7.35522e-1))./2.0;
t13458 = t8.*t13333.*2.62925e-3;
t13459 = (t13005.*(t2904-t2927))./4.0;
t13470 = (t10408.*t10577)./4.0;
t13471 = -t13463;
t13507 = t16.*t13376.*2.62925e-3;
t13531 = -t13518;
t13539 = t7797.*(t8266-t10204).*(-1.0./4.0);
t13543 = (t7797.*(t8266-t10204))./4.0;
t13567 = (t10141.*t10936)./4.0;
t13574 = t16.*t10153.*(t1589-t2213+t3195-t4346+t4355+t4748.*7.35522e-1+t2772.*(t71-t391)+t2775.*(t71-t391)).*(-1.0./4.0);
t13577 = t10141.*(t6472-t9256).*(-1.0./4.0);
t13586 = t10199.*(t1589-t2213+t3195-t4346+t4355+t4748.*7.35522e-1+t2772.*(t71-t391)+t2775.*(t71-t391)).*(-1.0./4.0);
t13587 = (t10141.*t10973)./4.0;
t13597 = (t5365.*t13005)./4.0;
t13608 = -t13603;
t13615 = t13518.*7.35522e-1;
t13616 = t13519.*7.35522e-1;
t13638 = -t13634;
t13657 = -t13654;
t13675 = -t13670;
t13679 = (t4024.*t13333)./4.0;
t13680 = -t13674;
t13692 = -t13688;
t13703 = -t13700;
t13711 = t13519.*3.867742437e-3;
t13715 = t13518.*1.563719772e-3;
t13716 = (t10577.*t10850)./4.0;
t13719 = (t6069.*t13005)./4.0;
t13723 = (t6046.*t13013)./4.0;
t13726 = -t13722;
t13746 = -t13743;
t13750 = -t13747;
t13754 = (t10147.*t11336)./4.0;
t13760 = (t10147.*t11344)./4.0;
t13765 = (t10153.*t11343)./4.0;
t13771 = t10153.*(t9125+t7.*(t5026+t5.*(t2959-t2967)).*1.666555).*(-1.0./4.0);
t13773 = t10153.*(t9128+t7.*(t5026+t5.*(t2959-t2967)).*1.225946).*(-1.0./4.0);
t13779 = (t10153.*(t9125+t7.*(t5026+t5.*(t2959-t2967)).*1.666555))./4.0;
t13782 = (t10153.*(t9128+t7.*(t5026+t5.*(t2959-t2967)).*1.225946))./4.0;
t13783 = (t10577.*t10931)./4.0;
t13793 = -t13784;
t13808 = -t13800;
t13811 = -t13805;
t13841 = -t13835;
t13847 = -t13846;
t13852 = -t13851;
t13857 = -t13855;
t13862 = t11483.*(t1987-t2621+t3452-t4730+t5359+t9.*(t71-t391).*6.1597e-2+t17.*(t426-t581)).*(-1.0./2.0);
t13863 = t10170.*(t3418-t3879+t4324-t5228+t5802+t9.*(t71-t391).*4.5305948634e-2+t17.*(t426-t581).*7.35522e-1).*(-1.0./2.0);
t13866 = (t11483.*(t1987-t2621+t3452-t4730+t5359+t9.*(t71-t391).*6.1597e-2+t17.*(t426-t581)))./2.0;
t13867 = (t10170.*(t3418-t3879+t4324-t5228+t5802+t9.*(t71-t391).*4.5305948634e-2+t17.*(t426-t581).*7.35522e-1))./2.0;
t13878 = -t13874;
t13881 = (t5235.*t13333)./4.0;
t13905 = (t5234.*t13376)./4.0;
t13924 = (t6884.*t13005)./4.0;
t13936 = (t10577.*t11228)./4.0;
t13939 = (t6872.*t13013)./4.0;
t13969 = t10936.*(t1589-t2213+t3195-t4346+t4355+t4748.*7.35522e-1+t2772.*(t71-t391)+t2775.*(t71-t391)).*(-1.0./4.0);
t13971 = -t13967;
t13973 = ((t6472-t9256).*(t1589-t2213+t3195-t4346+t4355+t4748.*7.35522e-1+t2772.*(t71-t391)+t2775.*(t71-t391)))./4.0;
t13979 = t10973.*(t1589-t2213+t3195-t4346+t4355+t4748.*7.35522e-1+t2772.*(t71-t391)+t2775.*(t71-t391)).*(-1.0./4.0);
t13981 = -t13978;
t13986 = t9185.*(t8266-t10204).*(-1.0./4.0);
t13990 = (t9185.*(t8266-t10204))./4.0;
t14004 = t9194.*(t9.*(t16.*(t30.*(t2425-t2468)+t68.*(t2425-t2468))+t8.*(t7.*(t4650+t34.*(t2425-t2468))+t47.*(t2425-t2468)))+t17.*(t4654+t15.*(t4650+t34.*(t2425-t2468)))).*(-1.0./4.0);
t14007 = (t9194.*(t9.*(t16.*(t30.*(t2425-t2468)+t68.*(t2425-t2468))+t8.*(t7.*(t4650+t34.*(t2425-t2468))+t47.*(t2425-t2468)))+t17.*(t4654+t15.*(t4650+t34.*(t2425-t2468)))))./4.0;
t14010 = -t14006;
t14012 = -t14009;
t14013 = -t14011;
t14030 = -t14029;
t14031 = t16.*t13876.*4.38178973375e-3;
t14032 = t8.*t13879.*4.38178973375e-3;
t14036 = (t10153.*t11969)./4.0;
t14044 = -t14042;
t14057 = t1439+t2078+t13879;
t14058 = t1670+t2165+t13876;
t14063 = (t10147.*t12042)./4.0;
t14082 = -t14077;
t14083 = -t14078;
t14084 = (t10153.*t12050)./4.0;
t14088 = -t14085;
t14098 = (t3421.*t13974)./4.0;
t14099 = (t3489.*t13974)./4.0;
t14104 = t9744.*(t1292+t2073+t2694+t11671).*(-1.0./4.0);
t14112 = t3363+t3872+t9470+t11867;
t14118 = (t10147.*t12163)./4.0;
t14124 = -t14122;
t14126 = -t14125;
t14132 = (t8477.*t13005)./4.0;
t14133 = (t10153.*t12185)./4.0;
t14156 = t2031+t2474+t2569+t3581+t13519;
t14159 = (t7079.*t13376)./4.0;
t14172 = (t8640.*t13005)./4.0;
t14190 = -t14188;
t14193 = t16.*t14113.*2.62925e-3;
t14195 = t9185.*(t8221-t11008).*(-1.0./4.0);
t14205 = t16.*(-t1476+t2165+t13876).*4.38178973375e-3;
t14210 = (t10577.*t12049)./4.0;
t14236 = -t14230;
t14237 = -t14231;
t14253 = (t10153.*t12464)./4.0;
t14264 = -t14262;
t14266 = (t9110.*t13005)./4.0;
t14270 = (t9112.*t13013)./4.0;
t14271 = (t9744.*t12667)./4.0;
t14278 = t13333.*(-t1476-t1540+t2091+t2165+t2579+t8.*(t260+t468+t570+t2298)).*(-1.0./4.0);
t14281 = (t13333.*(-t1476-t1540+t2091+t2165+t2579+t8.*(t260+t468+t570+t2298)))./4.0;
t14287 = (t6046.*t13879)./4.0;
t14288 = (t6069.*t13876)./4.0;
t14290 = (t4021.*t14113)./4.0;
t14296 = (t8227.*t13376)./4.0;
t14303 = -t14302;
t14309 = -t14308;
t14314 = -t14311;
t14315 = -t14312;
t14320 = (t10577.*t12385)./4.0;
t14330 = (t5083.*(-t1476+t2165+t13876))./4.0;
t14331 = t10147.*(t3129+t3384+t3574+t7846+t9332).*(-1.0./4.0);
t14332 = (t10577.*t12396)./4.0;
t14333 = (t10147.*(t3129+t3384+t3574+t7846+t9332))./4.0;
t14336 = (t10153.*t12589)./4.0;
t14340 = -t14337;
t14347 = (t9744.*t12860)./4.0;
t14355 = (t6302.*t13974)./4.0;
t14378 = (t10153.*t12669)./4.0;
t14379 = (t5441.*(-t1476+t2165+t13876))./4.0;
t14381 = t3152+t3539+t14113;
t14399 = (t6884.*t13876)./4.0;
t14402 = (t5234.*t14113)./4.0;
t14405 = (t6872.*t13879)./4.0;
t14417 = (t9744.*t13019)./4.0;
t14437 = (t10586.*t12564)./4.0;
t14439 = (t5912.*(-t1476+t2165+t13876))./4.0;
t14441 = (t5915.*(-t1476+t2165+t13876))./4.0;
t14461 = t16.*(-t3045+t3539+t14113).*2.62925e-3;
t14484 = (t10153.*t12898)./4.0;
t14489 = t10469.*(t8221-t11008).*(-1.0./4.0);
t14491 = (t10469.*(t8221-t11008))./4.0;
t14507 = (t2520.*(-t3045+t3539+t14113))./4.0;
t14529 = (t10141.*t13005)./4.0;
t14551 = -t14547;
t14552 = -t14548;
t14561 = (t6677.*(-t1476+t2165+t13876))./4.0;
t14572 = (t3780.*(-t3045+t3539+t14113))./4.0;
t14587 = (t10147.*(t2810+t2988-t12589))./4.0;
t14593 = (t10147.*t13140)./4.0;
t14594 = (t10153.*(t2810+t2988-t12589))./4.0;
t14601 = (t10153.*t13140)./4.0;
t14604 = ((t9.*(t16.*(t30.*(t2425-t2468)+t68.*(t2425-t2468))+t8.*(t7.*(t4650+t34.*(t2425-t2468))+t47.*(t2425-t2468)))+t17.*(t4654+t15.*(t4650+t34.*(t2425-t2468)))).*(t3418-t3879+t4324-t5228+t5802+t9.*(t71-t391).*4.5305948634e-2+t17.*(t426-t581).*7.35522e-1))./4.0;
t14614 = -t14611;
t14624 = (t4509.*(-t3045+t3539+t14113))./4.0;
t14626 = (t4514.*(-t3045+t3539+t14113))./4.0;
t14635 = (t8191.*t13974)./4.0;
t14650 = (t7079.*t14113)./4.0;
t14654 = t9.*t14541.*1.13264871585e-2;
t14662 = t17.*t14542.*1.13264871585e-2;
t14668 = (t5050.*(-t3045+t3539+t14113))./4.0;
t14675 = (t7613.*(-t1476+t2165+t13876))./4.0;
t14678 = (t7646.*(-t1476+t2165+t13876))./4.0;
t14725 = t1728+t2213+t3940+t3941+t4346+t4371+t9468+t11874;
t14727 = (t8062.*(-t1476+t2165+t13876))./4.0;
t14742 = (t9110.*t13876)./4.0;
t14743 = (t9112.*t13879)./4.0;
t14744 = (t10147.*t13416)./4.0;
t14748 = (t10153.*t13416)./4.0;
t14753 = -t14751;
t14759 = (t5923.*(-t3045+t3539+t14113))./4.0;
t14764 = (t5952.*(-t3045+t3539+t14113))./4.0;
t14773 = (t6014.*(-t3045+t3539+t14113))./4.0;
t14790 = (t8227.*t14113)./4.0;
t14796 = (t8562.*(-t1476+t2165+t13876))./4.0;
t14815 = (-t1476+t2165+t13876).*(t3063+t3528+t3966-t5230).*(-1.0./4.0);
t14849 = (t8713.*(-t1476+t2165+t13876))./4.0;
t14857 = t13974.*(t249-t391.*(1.1e+1./1.25e+2)-t1912.*4.252e-3+t3505+t5357+t693.*(t71-t391)+t784.*(t71-t391)).*(-1.0./4.0);
t14860 = (t5434.*t14541)./4.0;
t14864 = (t5433.*t14542)./4.0;
t14866 = -t14862;
t14880 = (t6744.*(-t3045+t3539+t14113))./4.0;
t14892 = t3596+t3793+t3876+t3921+t4381+t10079+t12073;
t14898 = (t9744.*t13876)./4.0;
t14899 = (t6957.*(-t3045+t3539+t14113))./4.0;
t14902 = t13879.*(-t3045-t3218+t3458+t3539+t3878+t8.*(t260+t468+t570+t2298).*1.666555).*(-1.0./4.0);
t14909 = (-t3045+t3539+t14113).*(t1492+t2158+t2696-t4727).*(-1.0./4.0);
t14918 = t3432+t3474+t3527+t3542+t4169+t9768+t12465;
t14919 = t3466+t3470+t3498+t3537+t4168+t9767+t12469;
t14922 = (t9106.*(-t1476+t2165+t13876))./4.0;
t14923 = (t7105.*(-t3045+t3539+t14113))./4.0;
t14925 = -t14924;
t14950 = -t14947;
t14962 = t9.*(t3543+t3820+t3911+t3949+t4360+t12067+t17.*(t258+t2289+t5392+t7559).*7.35522e-1).*(-1.539925e-2);
t14964 = t9.*(t3543+t3820+t3911+t3949+t4360+t12067+t17.*(t258+t2289+t5392+t7559).*7.35522e-1).*1.539925e-2;
t14966 = (t9269.*(-t1476+t2165+t13876))./4.0;
t14967 = (t7434.*(-t3045+t3539+t14113))./4.0;
t15012 = t8654.*(t249-t391.*(1.1e+1./1.25e+2)-t1912.*4.252e-3+t3505+t13496+t693.*(t71-t391)+t784.*(t71-t391)).*(-1.0./2.0);
t15013 = t8654.*(t249-t391.*(1.1e+1./1.25e+2)-t1912.*4.252e-3+t3505+t13496+t693.*(t71-t391)+t784.*(t71-t391)).*(-1.0./4.0);
t15016 = (t8654.*(t249-t391.*(1.1e+1./1.25e+2)-t1912.*4.252e-3+t3505+t13496+t693.*(t71-t391)+t784.*(t71-t391)))./2.0;
t15017 = (t8654.*(t249-t391.*(1.1e+1./1.25e+2)-t1912.*4.252e-3+t3505+t13496+t693.*(t71-t391)+t784.*(t71-t391)))./4.0;
t15041 = t3738.*(t3543+t3820+t3911+t3949+t4360+t12067+t17.*(t258+t2289+t5392+t7559).*7.35522e-1).*(-1.0./4.0);
t15044 = (t3738.*(t3543+t3820+t3911+t3949+t4360+t12067+t17.*(t258+t2289+t5392+t7559).*7.35522e-1))./4.0;
t15049 = (t8253.*(-t3045+t3539+t14113))./4.0;
t15050 = (t9743.*(-t1476+t2165+t13876))./4.0;
t15089 = t2711+t3823+t3943+t3991+t11871+t11872;
t15123 = -t15122;
t15132 = -t15131;
t15140 = t9.*t15088.*1.539925e-2;
t15174 = t5329.*(t3543+t3820+t3911+t3949+t4360+t12067+t17.*(t258+t2289+t5392+t7559).*7.35522e-1).*(-1.0./4.0);
t15176 = (t5329.*(t3543+t3820+t3911+t3949+t4360+t12067+t17.*(t258+t2289+t5392+t7559).*7.35522e-1))./4.0;
t15201 = t8.*t10153.*(-t1476+t2165+t13876).*4.1663875e-1;
t15208 = t8.*(t6452-t8229).*(-t1476+t2165+t13876).*(-4.1663875e-1);
t15210 = t8.*(t6452-t8229).*(-t1476+t2165+t13876).*4.1663875e-1;
t15223 = -t15220;
t15225 = -t15221;
t15231 = (t10597.*(-t1476+t2165+t13876))./4.0;
t15237 = (t16.*(t30.*(t2425-t2468)+t68.*(t2425-t2468)).*1.666555+t8.*(t7.*(t4650+t34.*(t2425-t2468))+t47.*(t2425-t2468)).*1.666555).*(-t1476+t2165+t13876).*(-1.0./4.0);
t15242 = ((t16.*(t30.*(t2425-t2468)+t68.*(t2425-t2468)).*1.666555+t8.*(t7.*(t4650+t34.*(t2425-t2468))+t47.*(t2425-t2468)).*1.666555).*(-t1476+t2165+t13876))./4.0;
t15243 = -t15238;
t15332 = t6811.*(t3543+t3820+t3911+t3949+t4360+t12067+t17.*(t258+t2289+t5392+t7559).*7.35522e-1).*(-1.0./4.0);
t15333 = t9194.*(t2148+t2513+t2649+t2661+t3582+t11950+t17.*(t258+t2289+t5392+t7559)).*(-1.0./4.0);
t15336 = (t6811.*(t3543+t3820+t3911+t3949+t4360+t12067+t17.*(t258+t2289+t5392+t7559).*7.35522e-1))./4.0;
t15337 = (t9194.*(t2148+t2513+t2649+t2661+t3582+t11950+t17.*(t258+t2289+t5392+t7559)))./4.0;
t15340 = -t15335;
t15347 = (t5329.*t15088)./4.0;
t15351 = (t9194.*t14541)./4.0;
t15361 = (t9185.*t14542)./4.0;
t15374 = -t15373;
t15382 = t16.*t10153.*(t249-t391.*(1.1e+1./1.25e+2)-t1912.*4.252e-3+t3505+t13496+t693.*(t71-t391)+t784.*(t71-t391)).*(-1.838805e-1);
t15386 = t16.*t10153.*(t249-t391.*(1.1e+1./1.25e+2)-t1912.*4.252e-3+t3505+t13496+t693.*(t71-t391)+t784.*(t71-t391)).*1.838805e-1;
t15392 = -t15391;
t15406 = (t8.*t10153.*(-t3045+t3539+t14113))./4.0;
t15409 = (t10182.*(-t3045+t3539+t14113))./4.0;
t15413 = t8.*(t6452-t8229).*(-t3045+t3539+t14113).*(-1.0./4.0);
t15417 = (t8.*(t6452-t8229).*(-t3045+t3539+t14113))./4.0;
t15427 = (t11390.*(-t1476+t2165+t13876))./4.0;
t15428 = (t16.*(t30.*(t2425-t2468)+t68.*(t2425-t2468))+t8.*(t7.*(t4650+t34.*(t2425-t2468))+t47.*(t2425-t2468))).*(-t3045+t3539+t14113).*(-1.0./4.0);
t15429 = ((t16.*(t30.*(t2425-t2468)+t68.*(t2425-t2468))+t8.*(t7.*(t4650+t34.*(t2425-t2468))+t47.*(t2425-t2468))).*(-t3045+t3539+t14113))./4.0;
t15448 = (t6811.*t15088)./4.0;
t15451 = t2500+t2647+t3521+t11672+t13530;
t15462 = (t9194.*t14770)./4.0;
t15488 = (t10468.*t14541)./4.0;
t15492 = (t10920.*(-t3045+t3539+t14113))./4.0;
t15495 = (t10469.*t14542)./4.0;
t15496 = t9.*(t2497+t2680+t3516+t9.*(t210+t2107+t7423+t9121)+t17.*(t9166-t11658)).*(-1.13264871585e-2);
t15500 = t9.*(t2497+t2680+t3516+t9.*(t210+t2107+t7423+t9121)+t17.*(t9166-t11658)).*1.13264871585e-2;
t15506 = ((t9253-t44.*(t4540+t5.*(t2425-t2468))).*(-t3045+t3539+t14113))./4.0;
t15511 = (t10974.*(-t3045+t3539+t14113))./4.0;
t15525 = t2017+t2639+t15449;
t15528 = t16.*t10153.*(t1589-t2213-t4346+t4355+t9454+t11863+t2772.*(t71-t391)+t2775.*(t71-t391)).*(-1.0./4.0);
t15529 = (t16.*t10153.*(t1589-t2213-t4346+t4355+t9454+t11863+t2772.*(t71-t391)+t2775.*(t71-t391)))./4.0;
t15530 = t10199.*(t1589-t2213-t4346+t4355+t9454+t11863+t2772.*(t71-t391)+t2775.*(t71-t391)).*(-1.0./4.0);
t15532 = -t15531;
t15534 = -t15533;
t15536 = t3846+t3924+t4341+t11864+t13624;
t15549 = (t8979.*t15088)./4.0;
t15553 = t5434.*(t2497+t2680+t3516+t9.*(t210+t2107+t7423+t9121)+t17.*(t9166-t11658)).*(-1.0./4.0);
t15554 = (t5434.*(t2497+t2680+t3516+t9.*(t210+t2107+t7423+t9121)+t17.*(t9166-t11658)))./4.0;
t15556 = t9.*(t2091+t2497+t2579+t2680+t3516+t9.*(t210+t2107+t7423+t9121)+t17.*(t9166-t11658)).*(-1.13264871585e-2);
t15559 = t9.*(t2091+t2497+t2579+t2680+t3516+t9.*(t210+t2107+t7423+t9121)+t17.*(t9166-t11658)).*1.13264871585e-2;
t15561 = t9.*(t3845+t3925+t4339+t9.*(t210+t2107+t7423+t9121).*7.35522e-1+t17.*(t9166-t11658).*7.35522e-1).*(-1.539925e-2);
t15563 = t9.*(t3845+t3925+t4339+t9.*(t210+t2107+t7423+t9121).*7.35522e-1+t17.*(t9166-t11658).*7.35522e-1).*1.539925e-2;
t15584 = -t15580;
t15597 = t4300.*(t2091+t2497+t2579+t2680+t3516+t9.*(t210+t2107+t7423+t9121)+t17.*(t9166-t11658)).*(-1.0./4.0);
t15598 = ((t3543+t3820+t3911+t3949+t4360+t12067+t17.*(t258+t2289+t5392+t7559).*7.35522e-1).*(t1987-t2621+t3452-t4730+t5359+t9.*(t71-t391).*6.1597e-2+t17.*(t426-t581)))./4.0;
t15599 = ((t2148+t2513+t2649+t2661+t3582+t11950+t17.*(t258+t2289+t5392+t7559)).*(t3418-t3879+t4324-t5228+t5802+t9.*(t71-t391).*4.5305948634e-2+t17.*(t426-t581).*7.35522e-1))./4.0;
t15600 = (t4300.*(t2091+t2497+t2579+t2680+t3516+t9.*(t210+t2107+t7423+t9121)+t17.*(t9166-t11658)))./4.0;
t15603 = t14541.*(t3418-t3879+t4324-t5228+t5802+t9.*(t71-t391).*4.5305948634e-2+t17.*(t426-t581).*7.35522e-1).*(-1.0./4.0);
t15607 = t3738.*(t3845+t3925+t4339+t9.*(t210+t2107+t7423+t9121).*7.35522e-1+t17.*(t9166-t11658).*7.35522e-1).*(-1.0./4.0);
t15608 = (t3738.*(t3845+t3925+t4339+t9.*(t210+t2107+t7423+t9121).*7.35522e-1+t17.*(t9166-t11658).*7.35522e-1))./4.0;
t15611 = t10936.*(t1589-t2213-t4346+t4355+t9454+t11863+t2772.*(t71-t391)+t2775.*(t71-t391)).*(-1.0./4.0);
t15612 = ((t6472-t9256).*(t1589-t2213-t4346+t4355+t9454+t11863+t2772.*(t71-t391)+t2775.*(t71-t391)))./4.0;
t15613 = t10973.*(t1589-t2213-t4346+t4355+t9454+t11863+t2772.*(t71-t391)+t2775.*(t71-t391)).*(-1.0./4.0);
t15616 = (t12792.*(-t1476+t2165+t13876))./2.0;
t15618 = t5448.*(t2091+t2497+t2579+t2680+t3516+t9.*(t210+t2107+t7423+t9121)+t17.*(t9166-t11658)).*(-1.0./4.0);
t15619 = (t5448.*(t2091+t2497+t2579+t2680+t3516+t9.*(t210+t2107+t7423+t9121)+t17.*(t9166-t11658)))./4.0;
t15641 = t5329.*(t3845+t3925+t4339+t9.*(t210+t2107+t7423+t9121).*7.35522e-1+t17.*(t9166-t11658).*7.35522e-1).*(-1.0./4.0);
t15643 = (t5329.*(t3845+t3925+t4339+t9.*(t210+t2107+t7423+t9121).*7.35522e-1+t17.*(t9166-t11658).*7.35522e-1))./4.0;
t15645 = t3372+t3917+t15535;
t15650 = t15088.*(t1987-t2621+t3452-t4730+t5359+t9.*(t71-t391).*6.1597e-2+t17.*(t426-t581)).*(-1.0./4.0);
t15651 = (t15088.*(t1987-t2621+t3452-t4730+t5359+t9.*(t71-t391).*6.1597e-2+t17.*(t426-t581)))./4.0;
t15654 = (t12392.*(-t3045+t3539+t14113))./2.0;
t15655 = t7796.*(t2497+t2680+t3516+t9.*(t210+t2107+t7423+t9121)+t17.*(t9166-t11658)).*(-1.0./4.0);
t15656 = (t7796.*(t2497+t2680+t3516+t9.*(t210+t2107+t7423+t9121)+t17.*(t9166-t11658)))./4.0;
t15659 = t6408.*(t2091+t2497+t2579+t2680+t3516+t9.*(t210+t2107+t7423+t9121)+t17.*(t9166-t11658)).*(-1.0./4.0);
t15661 = (t6408.*(t2091+t2497+t2579+t2680+t3516+t9.*(t210+t2107+t7423+t9121)+t17.*(t9166-t11658)))./4.0;
t15662 = t9.*(t3423+t3845+t3888+t3925+t4339+t9.*(t210+t2107+t7423+t9121).*7.35522e-1+t17.*(t9166-t11658).*7.35522e-1).*(-1.539925e-2);
t15664 = t9.*(t3423+t3845+t3888+t3925+t4339+t9.*(t210+t2107+t7423+t9121).*7.35522e-1+t17.*(t9166-t11658).*7.35522e-1).*1.539925e-2;
t15666 = t14770.*(t3418-t3879+t4324-t5228+t5802+t9.*(t71-t391).*4.5305948634e-2+t17.*(t426-t581).*7.35522e-1).*(-1.0./4.0);
t15667 = (t14770.*(t3418-t3879+t4324-t5228+t5802+t9.*(t71-t391).*4.5305948634e-2+t17.*(t426-t581).*7.35522e-1))./4.0;
t15669 = t2054.*(t3423+t3845+t3888+t3925+t4339+t9.*(t210+t2107+t7423+t9121).*7.35522e-1+t17.*(t9166-t11658).*7.35522e-1).*(-1.0./4.0);
t15671 = (t2054.*(t3423+t3845+t3888+t3925+t4339+t9.*(t210+t2107+t7423+t9121).*7.35522e-1+t17.*(t9166-t11658).*7.35522e-1))./4.0;
t15674 = t14821.*(t3418-t3879+t4324-t5228+t5802+t9.*(t71-t391).*4.5305948634e-2+t17.*(t426-t581).*7.35522e-1).*(-1.0./4.0);
t15677 = (t14821.*(t3418-t3879+t4324-t5228+t5802+t9.*(t71-t391).*4.5305948634e-2+t17.*(t426-t581).*7.35522e-1))./4.0;
t15681 = t6781.*(t2091+t2497+t2579+t2680+t3516+t9.*(t210+t2107+t7423+t9121)+t17.*(t9166-t11658)).*(-1.0./4.0);
t15682 = (t6781.*(t2091+t2497+t2579+t2680+t3516+t9.*(t210+t2107+t7423+t9121)+t17.*(t9166-t11658)))./4.0;
t15688 = t3767.*(t3423+t3845+t3888+t3925+t4339+t9.*(t210+t2107+t7423+t9121).*7.35522e-1+t17.*(t9166-t11658).*7.35522e-1).*(-1.0./4.0);
t15690 = (t3767.*(t3423+t3845+t3888+t3925+t4339+t9.*(t210+t2107+t7423+t9121).*7.35522e-1+t17.*(t9166-t11658).*7.35522e-1))./4.0;
t15694 = t6811.*(t3845+t3925+t4339+t9.*(t210+t2107+t7423+t9121).*7.35522e-1+t17.*(t9166-t11658).*7.35522e-1).*(-1.0./4.0);
t15695 = (t6811.*(t3845+t3925+t4339+t9.*(t210+t2107+t7423+t9121).*7.35522e-1+t17.*(t9166-t11658).*7.35522e-1))./4.0;
t15698 = (t12696.*(-t3045+t3539+t14113))./2.0;
t15699 = (t13333.*(-t1476+t2165+t13876))./2.0;
t15700 = t7540.*(t2091+t2497+t2579+t2680+t3516+t9.*(t210+t2107+t7423+t9121)+t17.*(t9166-t11658)).*(-1.0./4.0);
t15702 = (t7540.*(t2091+t2497+t2579+t2680+t3516+t9.*(t210+t2107+t7423+t9121)+t17.*(t9166-t11658)))./4.0;
t15705 = t4517.*(t3423+t3845+t3888+t3925+t4339+t9.*(t210+t2107+t7423+t9121).*7.35522e-1+t17.*(t9166-t11658).*7.35522e-1).*(-1.0./4.0);
t15706 = (t4517.*(t3423+t3845+t3888+t3925+t4339+t9.*(t210+t2107+t7423+t9121).*7.35522e-1+t17.*(t9166-t11658).*7.35522e-1))./4.0;
t15711 = t4772.*(t3423+t3845+t3888+t3925+t4339+t9.*(t210+t2107+t7423+t9121).*7.35522e-1+t17.*(t9166-t11658).*7.35522e-1).*(-1.0./4.0);
t15712 = (t4772.*(t3423+t3845+t3888+t3925+t4339+t9.*(t210+t2107+t7423+t9121).*7.35522e-1+t17.*(t9166-t11658).*7.35522e-1))./4.0;
t15716 = t7856.*(t2091+t2497+t2579+t2680+t3516+t9.*(t210+t2107+t7423+t9121)+t17.*(t9166-t11658)).*(-1.0./4.0);
t15718 = (t7856.*(t2091+t2497+t2579+t2680+t3516+t9.*(t210+t2107+t7423+t9121)+t17.*(t9166-t11658)))./4.0;
t15719 = t7901.*(t2091+t2497+t2579+t2680+t3516+t9.*(t210+t2107+t7423+t9121)+t17.*(t9166-t11658)).*(-1.0./4.0);
t15726 = t5217.*(t3423+t3845+t3888+t3925+t4339+t9.*(t210+t2107+t7423+t9121).*7.35522e-1+t17.*(t9166-t11658).*7.35522e-1).*(-1.0./4.0);
t15728 = (t5217.*(t3423+t3845+t3888+t3925+t4339+t9.*(t210+t2107+t7423+t9121).*7.35522e-1+t17.*(t9166-t11658).*7.35522e-1))./4.0;
t15731 = t9194.*(t2497+t2680+t3516+t9.*(t210+t2107+t7423+t9121)+t17.*(t9166-t11658)).*(-1.0./4.0);
t15733 = (t9194.*(t2497+t2680+t3516+t9.*(t210+t2107+t7423+t9121)+t17.*(t9166-t11658)))./4.0;
t15741 = t8464.*(t2091+t2497+t2579+t2680+t3516+t9.*(t210+t2107+t7423+t9121)+t17.*(t9166-t11658)).*(-1.0./4.0);
t15743 = (t8464.*(t2091+t2497+t2579+t2680+t3516+t9.*(t210+t2107+t7423+t9121)+t17.*(t9166-t11658)))./4.0;
t15746 = (t13013.*(-t3045+t3539+t14113))./2.0;
t15753 = t5719.*(t3423+t3845+t3888+t3925+t4339+t9.*(t210+t2107+t7423+t9121).*7.35522e-1+t17.*(t9166-t11658).*7.35522e-1).*(-1.0./4.0);
t15754 = (t13627.*(-t1476+t2165+t13876))./2.0;
t15755 = (t13038.*(-t3045+t3539+t14113))./2.0;
t15756 = (t5719.*(t3423+t3845+t3888+t3925+t4339+t9.*(t210+t2107+t7423+t9121).*7.35522e-1+t17.*(t9166-t11658).*7.35522e-1))./4.0;
t15759 = t5760.*(t3423+t3845+t3888+t3925+t4339+t9.*(t210+t2107+t7423+t9121).*7.35522e-1+t17.*(t9166-t11658).*7.35522e-1).*(-1.0./4.0);
t15763 = t6038.*(t3423+t3845+t3888+t3925+t4339+t9.*(t210+t2107+t7423+t9121).*7.35522e-1+t17.*(t9166-t11658).*7.35522e-1).*(-1.0./4.0);
t15765 = (t6038.*(t3423+t3845+t3888+t3925+t4339+t9.*(t210+t2107+t7423+t9121).*7.35522e-1+t17.*(t9166-t11658).*7.35522e-1))./4.0;
t15766 = t6526.*(t3423+t3845+t3888+t3925+t4339+t9.*(t210+t2107+t7423+t9121).*7.35522e-1+t17.*(t9166-t11658).*7.35522e-1).*(-1.0./4.0);
t15767 = (t6526.*(t3423+t3845+t3888+t3925+t4339+t9.*(t210+t2107+t7423+t9121).*7.35522e-1+t17.*(t9166-t11658).*7.35522e-1))./4.0;
t15768 = t9049.*(t2091+t2497+t2579+t2680+t3516+t9.*(t210+t2107+t7423+t9121)+t17.*(t9166-t11658)).*(-1.0./4.0);
t15769 = t9050.*(t2091+t2497+t2579+t2680+t3516+t9.*(t210+t2107+t7423+t9121)+t17.*(t9166-t11658)).*(-1.0./4.0);
t15770 = (t9049.*(t2091+t2497+t2579+t2680+t3516+t9.*(t210+t2107+t7423+t9121)+t17.*(t9166-t11658)))./4.0;
t15771 = (t9050.*(t2091+t2497+t2579+t2680+t3516+t9.*(t210+t2107+t7423+t9121)+t17.*(t9166-t11658)))./4.0;
t15777 = t8979.*(t3845+t3925+t4339+t9.*(t210+t2107+t7423+t9121).*7.35522e-1+t17.*(t9166-t11658).*7.35522e-1).*(-1.0./4.0);
t15778 = (t8979.*(t3845+t3925+t4339+t9.*(t210+t2107+t7423+t9121).*7.35522e-1+t17.*(t9166-t11658).*7.35522e-1))./4.0;
t15783 = t9362.*(t2091+t2497+t2579+t2680+t3516+t9.*(t210+t2107+t7423+t9121)+t17.*(t9166-t11658)).*(-1.0./4.0);
t15786 = t9538.*(t2091+t2497+t2579+t2680+t3516+t9.*(t210+t2107+t7423+t9121)+t17.*(t9166-t11658)).*(-1.0./4.0);
t15787 = t7348.*(t3423+t3845+t3888+t3925+t4339+t9.*(t210+t2107+t7423+t9121).*7.35522e-1+t17.*(t9166-t11658).*7.35522e-1).*(-1.0./4.0);
t15788 = (t9538.*(t2091+t2497+t2579+t2680+t3516+t9.*(t210+t2107+t7423+t9121)+t17.*(t9166-t11658)))./4.0;
t15790 = (t7348.*(t3423+t3845+t3888+t3925+t4339+t9.*(t210+t2107+t7423+t9121).*7.35522e-1+t17.*(t9166-t11658).*7.35522e-1))./4.0;
t15794 = t10468.*(t2497+t2680+t3516+t9.*(t210+t2107+t7423+t9121)+t17.*(t9166-t11658)).*(-1.0./4.0);
t15795 = (t10468.*(t2497+t2680+t3516+t9.*(t210+t2107+t7423+t9121)+t17.*(t9166-t11658)))./4.0;
t15798 = (t2056+t2203+t2351+t3433+t3503+t16.*t389.*(1.1e+1./1.25e+2)).*(t3423+t3845+t3888+t3925+t4339+t9.*(t210+t2107+t7423+t9121).*7.35522e-1+t17.*(t9166-t11658).*7.35522e-1).*(-1.0./4.0);
t15799 = ((t2056+t2203+t2351+t3433+t3503+t16.*t389.*(1.1e+1./1.25e+2)).*(t3423+t3845+t3888+t3925+t4339+t9.*(t210+t2107+t7423+t9121).*7.35522e-1+t17.*(t9166-t11658).*7.35522e-1))./4.0;
t15802 = t7940.*(t3423+t3845+t3888+t3925+t4339+t9.*(t210+t2107+t7423+t9121).*7.35522e-1+t17.*(t9166-t11658).*7.35522e-1).*(-1.0./4.0);
t15804 = t9887.*(t2091+t2497+t2579+t2680+t3516+t9.*(t210+t2107+t7423+t9121)+t17.*(t9166-t11658)).*(-1.0./4.0);
t15805 = t7982.*(t3423+t3845+t3888+t3925+t4339+t9.*(t210+t2107+t7423+t9121).*7.35522e-1+t17.*(t9166-t11658).*7.35522e-1).*(-1.0./4.0);
t15810 = t13005.*(t1589-t2213-t4346+t4355+t9454+t11863+t2772.*(t71-t391)+t2775.*(t71-t391)).*(-1.0./2.0);
t15817 = t13974.*(t249-t391.*(1.1e+1./1.25e+2)-t1912.*4.252e-3+t3505+t13496+t693.*(t71-t391)+t784.*(t71-t391)).*(-1.0./2.0);
t15818 = (t13974.*(t249-t391.*(1.1e+1./1.25e+2)-t1912.*4.252e-3+t3505+t13496+t693.*(t71-t391)+t784.*(t71-t391)))./2.0;
t15819 = t8725.*(t3423+t3845+t3888+t3925+t4339+t9.*(t210+t2107+t7423+t9121).*7.35522e-1+t17.*(t9166-t11658).*7.35522e-1).*(-1.0./4.0);
t15823 = ((t4324-t5228+t5802+t9.*(t71-t391).*4.5305948634e-2+t17.*(t426-t581).*7.35522e-1).*(t2091+t2497+t2579+t2680+t3516+t9.*(t210+t2107+t7423+t9121)+t17.*(t9166-t11658)))./4.0;
t15824 = ((t3845+t3925+t4339+t9.*(t210+t2107+t7423+t9121).*7.35522e-1+t17.*(t9166-t11658).*7.35522e-1).*(t1987-t2621+t3452-t4730+t5359+t9.*(t71-t391).*6.1597e-2+t17.*(t426-t581)))./4.0;
t15830 = t9001.*(t3423+t3845+t3888+t3925+t4339+t9.*(t210+t2107+t7423+t9121).*7.35522e-1+t17.*(t9166-t11658).*7.35522e-1).*(-1.0./4.0);
t15831 = t10485.*(t2091+t2497+t2579+t2680+t3516+t9.*(t210+t2107+t7423+t9121)+t17.*(t9166-t11658)).*(-1.0./4.0);
t15833 = t10480.*(t1987-t2621+t3452+t11654+t9.*(t71-t391).*6.1597e-2+t17.*(t426-t581)+t9.*(t9166-t11658)).*(-1.0./4.0);
t15836 = ((-t3823+t3970+t5243+t9.*(t260+t468+t570+t2298).*7.35522e-1+t972.*(t71-t391)+t2777.*(t71-t391)).*(t2091+t2497+t2579+t2680+t3516+t9.*(t210+t2107+t7423+t9121)+t17.*(t9166-t11658)))./4.0;
t15840 = (t13879.*(-t3045+t3539+t14113))./2.0;
t15845 = ((-t2550+t2696+t2698+t4771+t9.*(t260+t468+t570+t2298)+t147.*(t71-t391)).*(t3423+t3845+t3888+t3925+t4339+t9.*(t210+t2107+t7423+t9121).*7.35522e-1+t17.*(t9166-t11658).*7.35522e-1))./4.0;
t15849 = t9197.*(t3423+t3845+t3888+t3925+t4339+t9.*(t210+t2107+t7423+t9121).*7.35522e-1+t17.*(t9166-t11658).*7.35522e-1).*(-1.0./4.0);
t15850 = t10763.*(t2091+t2497+t2579+t2680+t3516+t9.*(t210+t2107+t7423+t9121)+t17.*(t9166-t11658)).*(-1.0./4.0);
t15851 = (t9197.*(t3423+t3845+t3888+t3925+t4339+t9.*(t210+t2107+t7423+t9121).*7.35522e-1+t17.*(t9166-t11658).*7.35522e-1))./4.0;
t15852 = (t10763.*(t2091+t2497+t2579+t2680+t3516+t9.*(t210+t2107+t7423+t9121)+t17.*(t9166-t11658)))./4.0;
t15853 = t9233.*(t3423+t3845+t3888+t3925+t4339+t9.*(t210+t2107+t7423+t9121).*7.35522e-1+t17.*(t9166-t11658).*7.35522e-1).*(-1.0./4.0);
t15854 = t10783.*(t2091+t2497+t2579+t2680+t3516+t9.*(t210+t2107+t7423+t9121)+t17.*(t9166-t11658)).*(-1.0./4.0);
t15860 = ((t2497+t2680+t3516+t9.*(t210+t2107+t7423+t9121)+t17.*(t9166-t11658)).*(t3418-t3879+t4324-t5228+t5802+t9.*(t71-t391).*4.5305948634e-2+t17.*(t426-t581).*7.35522e-1))./4.0;
t15861 = ((t3452-t4730+t5359+t9.*(t71-t391).*6.1597e-2+t17.*(t426-t581)).*(t3423+t3845+t3888+t3925+t4339+t9.*(t210+t2107+t7423+t9121).*7.35522e-1+t17.*(t9166-t11658).*7.35522e-1))./4.0;
t15877 = t10180.*(t3423+t3845+t3888+t3925+t4339+t9.*(t210+t2107+t7423+t9121).*7.35522e-1+t17.*(t9166-t11658).*7.35522e-1).*(-1.0./4.0);
t15878 = t11483.*(t1987-t2621+t3452+t11654+t9.*(t71-t391).*6.1597e-2+t17.*(t426-t581)+t9.*(t9166-t11658)).*(-1.0./4.0);
t15879 = t10170.*(t3418-t3879+t4324+t11855+t9.*(t71-t391).*4.5305948634e-2+t17.*(t426-t581).*7.35522e-1+t9.*(t9166-t11658).*7.35522e-1).*(-1.0./4.0);
t15880 = (t11483.*(t1987-t2621+t3452+t11654+t9.*(t71-t391).*6.1597e-2+t17.*(t426-t581)+t9.*(t9166-t11658)))./4.0;
t15881 = (t10170.*(t3418-t3879+t4324+t11855+t9.*(t71-t391).*4.5305948634e-2+t17.*(t426-t581).*7.35522e-1+t9.*(t9166-t11658).*7.35522e-1))./4.0;
t15917 = t12563.*(t2091+t2497+t2579+t2680+t3516+t9.*(t210+t2107+t7423+t9121)+t17.*(t9166-t11658)).*(-1.0./4.0);
t15919 = (t12563.*(t2091+t2497+t2579+t2680+t3516+t9.*(t210+t2107+t7423+t9121)+t17.*(t9166-t11658)))./4.0;
t15920 = -t15918;
t15975 = ((t8266-t10204).*(t3423+t3845+t3888+t3925+t4339+t9.*(t210+t2107+t7423+t9121).*7.35522e-1+t17.*(t9166-t11658).*7.35522e-1))./4.0;
t15982 = -t15980;
t15983 = ((t8329+t17.*(t16.*(t30.*(t2425-t2468)+t68.*(t2425-t2468))+t8.*(t7.*(t4650+t34.*(t2425-t2468))+t47.*(t2425-t2468)))).*(t3423+t3845+t3888+t3925+t4339+t9.*(t210+t2107+t7423+t9121).*7.35522e-1+t17.*(t9166-t11658).*7.35522e-1))./4.0;
t16009 = q4d.*t16008;
t16013 = ((t8221-t11008).*(t3423+t3845+t3888+t3925+t4339+t9.*(t210+t2107+t7423+t9121).*7.35522e-1+t17.*(t9166-t11658).*7.35522e-1))./4.0;
t16079 = ((t2189+t2495+t2635+t2646+t3580+t9.*(t258+t2289+t5392+t7559)+t17.*(t7693+t9904)).*(t3423+t3845+t3888+t3925+t4339+t9.*(t210+t2107+t7423+t9121).*7.35522e-1+t17.*(t9166-t11658).*7.35522e-1))./2.0;
t16081 = ((t2091+t2497+t2579+t2680+t3516+t9.*(t210+t2107+t7423+t9121)+t17.*(t9166-t11658)).*(t3471+t3796+t3914+t3942+t4358+t9.*(t258+t2289+t5392+t7559).*7.35522e-1+t17.*(t7693+t9904).*7.35522e-1))./2.0;
t16083 = ((t1987-t2621+t3452+t11654+t9.*(t71-t391).*6.1597e-2+t17.*(t426-t581)+t9.*(t9166-t11658)).*(t3543+t3820+t3911+t3949+t4360+t12067+t17.*(t258+t2289+t5392+t7559).*7.35522e-1))./2.0;
t16085 = t14541.*(t3418-t3879+t4324+t11855+t9.*(t71-t391).*4.5305948634e-2+t17.*(t426-t581).*7.35522e-1+t9.*(t9166-t11658).*7.35522e-1).*(-1.0./2.0);
t16086 = (t14541.*(t3418-t3879+t4324+t11855+t9.*(t71-t391).*4.5305948634e-2+t17.*(t426-t581).*7.35522e-1+t9.*(t9166-t11658).*7.35522e-1))./2.0;
t16089 = t14542.*(t3423+t3845+t3888+t3925+t4339+t9.*(t210+t2107+t7423+t9121).*7.35522e-1+t17.*(t9166-t11658).*7.35522e-1).*(-1.0./2.0);
t16091 = ((-t3823+t3970+t11861+t8.*t11864+t972.*(t71-t391)+t2777.*(t71-t391)).*(t2091+t2497+t2579+t2680+t3516+t9.*(t210+t2107+t7423+t9121)+t17.*(t9166-t11658)))./2.0;
t16092 = t15088.*(t1987-t2621+t3452+t11654+t9.*(t71-t391).*6.1597e-2+t17.*(t426-t581)+t9.*(t9166-t11658)).*(-1.0./2.0);
t16097 = ((-t2550+t2696+t2698+t11659+t8.*t11672+t147.*(t71-t391)).*(t3423+t3845+t3888+t3925+t4339+t9.*(t210+t2107+t7423+t9121).*7.35522e-1+t17.*(t9166-t11658).*7.35522e-1))./2.0;
t16099 = t14823.*(t3423+t3845+t3888+t3925+t4339+t9.*(t210+t2107+t7423+t9121).*7.35522e-1+t17.*(t9166-t11658).*7.35522e-1).*(-1.0./2.0);
t16100 = t15156.*(t2091+t2497+t2579+t2680+t3516+t9.*(t210+t2107+t7423+t9121)+t17.*(t9166-t11658)).*(-1.0./2.0);
t16106 = ((t3845+t3925+t4339+t9.*(t210+t2107+t7423+t9121).*7.35522e-1+t17.*(t9166-t11658).*7.35522e-1).*(t1987-t2621+t3452+t11654+t9.*(t71-t391).*6.1597e-2+t17.*(t426-t581)+t9.*(t9166-t11658)))./2.0;
t16107 = ((t4324+t11855+t9.*(t71-t391).*4.5305948634e-2+t17.*(t426-t581).*7.35522e-1+t9.*(t9166-t11658).*7.35522e-1).*(t2091+t2497+t2579+t2680+t3516+t9.*(t210+t2107+t7423+t9121)+t17.*(t9166-t11658)))./2.0;
t16109 = ((t3452+t11654+t9.*(t71-t391).*6.1597e-2+t17.*(t426-t581)+t9.*(t9166-t11658)).*(t3423+t3845+t3888+t3925+t4339+t9.*(t210+t2107+t7423+t9121).*7.35522e-1+t17.*(t9166-t11658).*7.35522e-1))./2.0;
t16110 = ((t2497+t2680+t3516+t9.*(t210+t2107+t7423+t9121)+t17.*(t9166-t11658)).*(t3418-t3879+t4324+t11855+t9.*(t71-t391).*4.5305948634e-2+t17.*(t426-t581).*7.35522e-1+t9.*(t9166-t11658).*7.35522e-1))./2.0;
t16118 = q4d.*t16117;
t16124 = -q2d.*(t6828+t6939+t8127-t12109+t12110+t12391-t12394+(t7475.*(t395+t9.*(t48-t349)))./2.0+(t439.*(-t2182+t2241+t696.*(t48-t349)+t891.*(t48-t349)))./2.0+(t10141.*(-t2149+t2205+t693.*(t48-t349)+t784.*(t48-t349)))./2.0+(t8191.*(t3479-t3544+t2772.*(t48-t349)+t2775.*(t48-t349)))./2.0);
t16132 = t4142+t4173+t4201+t4274+t4443+t4577+t4620+t4675+t4706+t4741+t4788+t5568+t5608+t6270+t6382+t7494+t7575+t8573+t8704+t8708+t8825+t9404+t9434+t9443+t9680+t9681+t10696+t10728+t10730;
t16148 = t5858+t5996+t6080+t6417+t6650+t6682+t7156+t7172+t7853+t7858+t7933+t9831+t10233+t10260+t10626+t10677+t10684+t10910+t11645+t11959+t11965+t12198+t12208;
t16153 = q4d.*t16151;
t16154 = -q2d.*(-t3995-t4013-t4190-t4197+t4291+t4306+t4448+t4462+t4520+t4539+t5127+t5140-t5688+t5906+t6001-t6439+t6487+t6491+t7633+t7758-t10457-t10565+t10573+t10755-t10760-t10844+t10845-t11160+t11236-t11240+(t5837.*(t395+t9.*(t48-t349)))./4.0+(t8477.*(-t2149+t2205+t693.*(t48-t349)+t784.*(t48-t349)))./4.0+(t5696.*(t3479-t3544+t2772.*(t48-t349)+t2775.*(t48-t349)))./4.0+(t15.*t16.*(-t2182+t2241+t696.*(t48-t349)+t891.*(t48-t349)))./4.0);
t16175 = t5401+t5404+t5429+t5864+t5939+t6062+t6066+t6077+t6991+t7081+t7084+t7099+t7282+t7341+t7741+t7977+t8099+t9152+t9177+t9181+t9463+t9481+t9764+t10219+t10235+t10255+t10633+t10674+t10699+t11886+t12026+t12193+t12199+t12373+t12375;
t16216 = t3835+t3856+t4042+t4054+t4170+t4181+t4228+t4239+t4267+t4282+t4285+t4340+t4367+t4579+t4599+t5061+t5082+t5091+t5402+t5428+t5706+t5714+t5744+t6100+t6238+t6255+t6290+t6311+t6323+t6843+t6869+t6961+t7085+t7530+t7539+t7636+t8058+t8459+t8524+t8717+t8719+t8770+t8772+t8831+t8835+t8933+t8973+t9068+t9614+t9624+t9773+t9935+t9970+t10013+t10122+t10125+t10299+t10301+t10328+t10466+t10473+t10629+t10665+t10821+t11175+t11190;
t9266 = -t9257;
t9268 = -t9259;
t9663 = -t9652;
t9797 = -t9784;
t9820 = -t9809;
t9882 = t9.*t9292.*1.13264871585e-2;
t9926 = t3367+t3819+t3875+t4361+t5846;
t9932 = -t9930;
t10015 = -t10007;
t10017 = -t10009;
t10121 = -t10118;
t10124 = (t5434.*t8743)./4.0;
t10137 = -t10133;
t10139 = -t10135;
t10149 = t2091+t2579+t9292;
t10152 = t2076+t2621+t9293;
t10172 = -t10158;
t10185 = t8.*t10173;
t10186 = -t10179;
t10187 = t8.*t10174;
t10193 = -t10174;
t10198 = -t10190;
t10378 = t10158.*7.35522e-1;
t10379 = t10159.*7.35522e-1;
t10381 = -t10370;
t10382 = t10160.*7.35522e-1;
t10383 = t10161.*7.35522e-1;
t10384 = t10158.*1.666555;
t10386 = t10160.*1.666555;
t10396 = -t10387;
t10399 = -t10388;
t10402 = t10173.*7.35522e-1;
t10403 = t10174.*7.35522e-1;
t10424 = -t10412;
t10427 = -t10418;
t10447 = t3846+t3924+t4341+t5228+t5815;
t10465 = -t10463;
t10511 = (t3743.*t9922)./4.0;
t10560 = -t10549;
t10578 = (t5434.*t9292)./4.0;
t10579 = t10159.*3.867742437e-3;
t10580 = t10160.*5.01208083475e-2;
t10587 = t10158.*1.17633784675e-2;
t10590 = t10161.*1.563719772e-3;
t10600 = t10173.*3.867742437e-3;
t10603 = -t10593;
t10609 = t10174.*1.563719772e-3;
t10613 = -t10604;
t10617 = -t10608;
t10623 = -t10611;
t10637 = -t10627;
t10638 = -t10628;
t10664 = -t10644;
t10666 = -t10645;
t10693 = -t10688;
t10707 = t9.*t10446.*1.539925e-2;
t10775 = -t10772;
t10817 = t7.*t10546.*8.639075e-2;
t10823 = t15.*t10554.*8.639075e-2;
t10824 = -t10819;
t10832 = -t10828;
t10833 = t16.*t10607.*2.62925e-3;
t10838 = -t10834;
t10962 = t9.*t10942;
t10963 = t17.*t10942;
t10965 = (t3738.*t10446)./4.0;
t11007 = (t5345.*t9922)./4.0;
t11012 = (t2966.*t10546)./4.0;
t11019 = (t2980.*t10554)./4.0;
t11027 = -t11021;
t11028 = -t11026;
t11036 = -t11030;
t11039 = -t11032;
t11043 = (t3249.*t10561)./4.0;
t11044 = -t11038;
t11048 = (t3265.*t10561)./4.0;
t11055 = -t11052;
t11062 = (t3360.*t10561)./4.0;
t11089 = -t11083;
t11094 = (t3421.*t10612)./4.0;
t11097 = (t3752.*t10550)./4.0;
t11098 = (t3489.*t10612)./4.0;
t11101 = (t3771.*t10561)./4.0;
t11103 = (t3752.*t10561)./4.0;
t11112 = -t11104;
t11115 = -t11109;
t11118 = -t11113;
t11127 = -t11122;
t11129 = t10938.*7.35522e-1;
t11130 = t10939.*7.35522e-1;
t11132 = -t11123;
t11136 = (t7796.*t8743)./4.0;
t11139 = -t11131;
t11152 = -t11145;
t11177 = (t4035.*t10546)./4.0;
t11179 = -t11173;
t11186 = (t4064.*t10554)./4.0;
t11205 = -t11198;
t11216 = (t4021.*t10607)./4.0;
t11220 = (t4255.*t10546)./4.0;
t11222 = (t4286.*t10546)./4.0;
t11225 = (t4255.*t10554)./4.0;
t11229 = (t4286.*t10554)./4.0;
t11254 = -t11246;
t11259 = -t11248;
t11278 = -t11270;
t11291 = (t4453.*t10561)./4.0;
t11293 = -t11284;
t11295 = -t11286;
t11307 = -t11302;
t11320 = -t11310;
t11354 = t10939.*3.867742437e-3;
t11355 = -t11351;
t11356 = t6848+t9567;
t11361 = t10938.*1.563719772e-3;
t11362 = t6876+t9565;
t11364 = t6883+t9563;
t11370 = -t11360;
t11374 = -t11368;
t11375 = -t11369;
t11384 = -t11376;
t11394 = t8.*t10942.*4.38178973375e-3;
t11417 = (t4837.*t10554)./4.0;
t11419 = (t4849.*t10546)./4.0;
t11422 = -t11415;
t11431 = -t11424;
t11433 = -t11429;
t11447 = -t11443;
t11464 = (t5329.*t10446)./4.0;
t11470 = t3423+t3888+t10446;
t11471 = (t5064.*t10546)./4.0;
t11481 = -t11477;
t11485 = (t5095.*t10554)./4.0;
t11493 = -t11490;
t11512 = -t11508;
t11528 = t8.*t11338.*2.62925e-3;
t11535 = t16.*t11341.*2.62925e-3;
t11537 = -t11531;
t11548 = -t11541;
t11549 = (t5275.*t10561)./4.0;
t11551 = -t11543;
t11554 = -t11545;
t11561 = -t11552;
t11563 = (t5234.*t10607)./4.0;
t11565 = -t11553;
t11569 = -t11557;
t11572 = t16.*(t6847-t9563).*(-2.62925e-3);
t11581 = t8.*t11372.*2.62925e-3;
t11591 = t16.*t11380.*2.62925e-3;
t11594 = -t11585;
t11599 = (t7796.*t9292)./4.0;
t11603 = -t11598;
t11613 = -t11608;
t11630 = (t6761.*t9922)./4.0;
t11649 = -t11641;
t11688 = (t5518.*t10561)./4.0;
t11690 = (t5523.*t10561)./4.0;
t11698 = (t5543.*t10561)./4.0;
t11711 = (t5613.*t10546)./4.0;
t11718 = t17.*t11484.*1.539925e-2;
t11724 = (t5634.*t10546)./4.0;
t11725 = -t11717;
t11728 = (t5628.*t10546)./4.0;
t11733 = (t5634.*t10554)./4.0;
t11736 = (t5628.*t10554)./4.0;
t11741 = (t5648.*t10554)./4.0;
t11744 = -t11740;
t11756 = (t5699.*t10550)./4.0;
t11758 = -t11748;
t11760 = -t11749;
t11766 = -t11754;
t11769 = (t5699.*t10561)./4.0;
t11799 = -t11789;
t11817 = (t5696.*t10612)./4.0;
t11825 = (t5806.*t10546)./4.0;
t11833 = t10546.*(t495+t572+t1838+t2069+t2107).*(-1.0./4.0);
t11835 = -t11831;
t11839 = (t5853.*t10554)./4.0;
t11840 = -t11836;
t11841 = (t5860.*t10554)./4.0;
t11844 = (t3421.*t11340)./4.0;
t11847 = (t3489.*t11340)./4.0;
t11873 = (t5928.*t10546)./4.0;
t11875 = t3421.*(t6834-t9565).*(-1.0./4.0);
t11878 = t3489.*(t6834-t9565).*(-1.0./4.0);
t11883 = (t3421.*t11377)./4.0;
t11884 = (t3489.*(t6834-t9565))./4.0;
t11885 = (t5999.*t10554)./4.0;
t11889 = (t3489.*t11377)./4.0;
t11902 = -t11900;
t11903 = -t11901;
t11910 = (t10561.*(-t1272-t1479+t1647+t1848+t2236))./4.0;
t11922 = -t11913;
t11928 = (t6193.*t10561)./4.0;
t11935 = t4021.*(t6847-t9563).*(-1.0./4.0);
t11940 = (t4021.*(t6847-t9563))./4.0;
t11942 = (t4024.*t11372)./4.0;
t11944 = (t4021.*t11380)./4.0;
t11962 = -t11954;
t11989 = (t6302.*t10612)./4.0;
t11991 = (t8743.*t9194)./4.0;
t11999 = -t11995;
t12003 = (t3743.*t11484)./4.0;
t12009 = -t12001;
t12012 = -t12005;
t12036 = (t6535.*t10561)./4.0;
t12044 = (t6811.*t10446)./4.0;
t12055 = (t6589.*t10550)./4.0;
t12057 = (t6589.*t10561)./4.0;
t12065 = -t12064;
t12078 = (t6654.*t10561)./4.0;
t12107 = -t12105;
t12126 = (t6046.*t10942)./4.0;
t12127 = (t6967.*t10546)./4.0;
t12129 = (t5235.*t11338)./4.0;
t12132 = (t6970.*t10561)./4.0;
t12134 = (t10546.*(t921+t1317-t5853))./4.0;
t12135 = (t5234.*t11341)./4.0;
t12136 = (t6988.*t10554)./4.0;
t12141 = (t10554.*(t921+t1317-t5853))./4.0;
t12151 = -t12142;
t12153 = (t7039.*t10546)./4.0;
t12158 = (t7039.*t10554)./4.0;
t12165 = -t12160;
t12169 = -t12161;
t12184 = (t7080.*t10561)./4.0;
t12236 = -t12229;
t12240 = -t12235;
t12242 = -t12238;
t12253 = -t12247;
t12264 = -t12259;
t12279 = t8158+t10160;
t12291 = -t9.*(t10158+t16.*(t4542-t6448));
t12292 = -t17.*(t10158+t16.*(t4542-t6448));
t12298 = (t9194.*t9292)./4.0;
t12300 = -t12293;
t12307 = t8192+t10207;
t12310 = -t12306;
t12357 = (t5345.*t11484)./4.0;
t12358 = t5696.*(t6834-t9565).*(-1.0./4.0);
t12363 = (t5696.*(t6834-t9565))./4.0;
t12365 = (t5696.*t11377)./4.0;
t12413 = -t12411;
t12414 = t9.*(t10158+t16.*(t4542-t6448)).*(-7.35522e-1);
t12415 = t17.*(t10158+t16.*(t4542-t6448)).*(-7.35522e-1);
t12426 = -t12422;
t12427 = (t7822.*t10550)./4.0;
t12430 = (t7822.*t10561)./4.0;
t12432 = (t8981.*t9922)./4.0;
t12442 = (t7875.*t10561)./4.0;
t12446 = -t12441;
t12453 = -t12449;
t12468 = -t12463;
t12471 = (t6302.*t11340)./4.0;
t12500 = t8557+t10414;
t12501 = t17.*(t10158+t16.*(t4542-t6448)).*(-3.867742437e-3);
t12503 = t8564+t10419;
t12504 = t8.*(t10158+t16.*(t4542-t6448)).*(-4.38178973375e-3);
t12505 = t9.*(t10158+t16.*(t4542-t6448)).*(-1.563719772e-3);
t12507 = t17.*(t10158+t16.*(t4542-t6448)).*3.867742437e-3;
t12509 = t8.*(t10158+t16.*(t4542-t6448)).*4.38178973375e-3;
t12510 = t9.*(t10158+t16.*(t4542-t6448)).*1.563719772e-3;
t12511 = t17.*t12296.*3.867742437e-3;
t12513 = t9.*t12296.*1.563719772e-3;
t12514 = t16.*t12296.*4.38178973375e-3;
t12516 = (t8227.*t10607)./4.0;
t12520 = t8612+t10438;
t12524 = t8616+t10439;
t12529 = t9.*t12339.*1.13264871585e-2;
t12599 = (t8743.*t10468)./4.0;
t12608 = -t12605;
t12617 = (t7079.*t11341)./4.0;
t12622 = t17.*(t8610-t10439).*(-1.539925e-2);
t12623 = (t7116.*t11338)./4.0;
t12628 = t7079.*(t6847-t9563).*(-1.0./4.0);
t12632 = (t7079.*t11380)./4.0;
t12640 = (t8979.*t10446)./4.0;
t12641 = (t7116.*t11372)./4.0;
t12649 = -t12647;
t12650 = (t6761.*t11484)./4.0;
t12668 = -t12658;
t12670 = -t12659;
t12672 = -t12660;
t12673 = -t12661;
t12689 = t8188+t10938;
t12693 = -t12685;
t12698 = t9.*t3738.*t12296.*1.838805e-1;
t12702 = t17.*t3743.*t12296.*1.838805e-1;
t12705 = t8222+t10939;
t12716 = -t12713;
t12724 = -t12721;
t12745 = -t12741;
t12773 = (t10158+t16.*(t4542-t6448)).*(t2904-t2927).*(-1.0./4.0);
t12774 = (t4896.*t12296)./4.0;
t12776 = ((t10158+t16.*(t4542-t6448)).*(t2904-t2927))./4.0;
t12781 = (t4938.*t12296)./4.0;
t12786 = (t12296.*(t2889-t2921))./4.0;
t12787 = (t12296.*(t2904-t2927))./4.0;
t12807 = t5083.*(t10158+t16.*(t4542-t6448)).*(-1.0./4.0);
t12810 = (t5083.*(t10158+t16.*(t4542-t6448)))./4.0;
t12816 = (t5069.*t12296)./4.0;
t12830 = -t12827;
t12862 = t3743.*(t8610-t10439).*(-1.0./4.0);
t12868 = (t3743.*(t8610-t10439))./4.0;
t12895 = (t9292.*t10468)./4.0;
t12904 = (t5365.*t12296)./4.0;
t12909 = t5441.*(t10158+t16.*(t4542-t6448)).*(-1.0./4.0);
t12922 = (t5430.*t12296)./4.0;
t12928 = (t9.*t5434.*t12296)./4.0;
t12929 = (t17.*t5433.*t12296)./4.0;
t12950 = (t5434.*t12339)./4.0;
t12952 = (t8191.*t11340)./4.0;
t12966 = (t8227.*t11341)./4.0;
t12968 = t11338.*(-t1476-t1540+t2091+t2165+t2579+t8.*(t260+t468+t570+t2298)).*(-1.0./4.0);
t12971 = (t11338.*(-t1476-t1540+t2091+t2165+t2579+t8.*(t260+t468+t570+t2298)))./4.0;
t12974 = t8191.*(t6834-t9565).*(-1.0./4.0);
t12977 = (t8191.*t11377)./4.0;
t12978 = t8227.*(t6847-t9563).*(-1.0./4.0);
t12981 = t10612.*(t249-t391.*(1.1e+1./1.25e+2)-t1912.*4.252e-3+t3505+t5357+t693.*(t71-t391)+t784.*(t71-t391)).*(-1.0./4.0);
t12983 = (t8227.*t11380)./4.0;
t12985 = t11372.*(-t1476-t1540+t2091+t2165+t2579+t8.*(t260+t468+t570+t2298)).*(-1.0./4.0);
t12987 = t8585+t11187;
t12991 = t8604+t11188;
t13006 = t9.*t12738.*1.13264871585e-2;
t13021 = t9.*t5329.*t12296.*1.838805e-1;
t13030 = t17.*t5345.*t12296.*1.838805e-1;
t13036 = -t13026;
t13047 = t5912.*(t10158+t16.*(t4542-t6448)).*(-1.0./4.0);
t13048 = t5915.*(t10158+t16.*(t4542-t6448)).*(-1.0./4.0);
t13050 = (t5912.*(t10158+t16.*(t4542-t6448)))./4.0;
t13051 = (t5915.*(t10158+t16.*(t4542-t6448)))./4.0;
t13054 = (t5914.*t12296)./4.0;
t13056 = (t5919.*t12296)./4.0;
t13058 = -t13055;
t13068 = t6046.*(t10158+t16.*(t4542-t6448)).*(-1.0./4.0);
t13072 = (t6046.*(t10158+t16.*(t4542-t6448)))./4.0;
t13073 = t6069.*(t10158+t16.*(t4542-t6448)).*(-1.0./4.0);
t13076 = (t6069.*(t10158+t16.*(t4542-t6448)))./4.0;
t13084 = (t6046.*t12296)./4.0;
t13092 = (t6069.*t12296)./4.0;
t13101 = (t6104.*t12296)./4.0;
t13113 = -t13107;
t13117 = -t13115;
t13122 = (t9112.*t10942)./4.0;
t13129 = t8.*t12867.*4.38178973375e-3;
t13135 = t17.*(t8583-t11188).*(-1.539925e-2);
t13145 = t13026.*7.35522e-1;
t13146 = t13027.*7.35522e-1;
t13147 = (t6304.*t12296)./4.0;
t13156 = t5345.*(t8610-t10439).*(-1.0./4.0);
t13158 = (t5345.*(t8610-t10439))./4.0;
t13181 = t9247+t11005;
t13208 = t6677.*(t10158+t16.*(t4542-t6448)).*(-1.0./4.0);
t13209 = t8743.*(t3418-t3879+t4324-t5228+t5802+t9.*(t71-t391).*4.5305948634e-2+t17.*(t426-t581).*7.35522e-1).*(-1.0./2.0);
t13210 = -t13207;
t13211 = t13027.*3.867742437e-3;
t13212 = (t8743.*(t3418-t3879+t4324-t5228+t5802+t9.*(t71-t391).*4.5305948634e-2+t17.*(t426-t581).*7.35522e-1))./2.0;
t13214 = t13026.*1.563719772e-3;
t13216 = -t13213;
t13220 = (t6681.*t12296)./4.0;
t13252 = t6884.*(t10158+t16.*(t4542-t6448)).*(-1.0./4.0);
t13255 = t6872.*(t10158+t16.*(t4542-t6448)).*(-1.0./4.0);
t13261 = (t6872.*(t10158+t16.*(t4542-t6448)))./4.0;
t13270 = (t6884.*t12296)./4.0;
t13274 = (t6872.*t12296)./4.0;
t13278 = t10446.*(t1987-t2621+t3452-t4730+t5359+t9.*(t71-t391).*6.1597e-2+t17.*(t426-t581)).*(-1.0./2.0);
t13291 = (t6966.*t12296)./4.0;
t13293 = t3743.*(t8583-t11188).*(-1.0./4.0);
t13295 = (t3743.*(t8583-t11188))./4.0;
t13317 = t16.*t13196.*2.62925e-3;
t13320 = t8.*t13198.*2.62925e-3;
t13345 = (t7215.*t12296)./4.0;
t13352 = t17.*t6761.*t12296.*1.838805e-1;
t13364 = t10942.*(-t3045-t3218+t3458+t3539+t3878+t8.*(t260+t468+t570+t2298).*1.666555).*(-1.0./4.0);
t13366 = (t5434.*t12738)./4.0;
t13367 = t9.*t6811.*t12296.*1.838805e-1;
t13373 = t11340.*(t249-t391.*(1.1e+1./1.25e+2)-t1912.*4.252e-3+t3505+t5357+t693.*(t71-t391)+t784.*(t71-t391)).*(-1.0./4.0);
t13382 = t9553+t11174;
t13387 = t10413+t10445;
t13388 = ((t6834-t9565).*(t249-t391.*(1.1e+1./1.25e+2)-t1912.*4.252e-3+t3505+t5357+t693.*(t71-t391)+t784.*(t71-t391)))./4.0;
t13391 = t10415+t10460;
t13394 = t11377.*(t249-t391.*(1.1e+1./1.25e+2)-t1912.*4.252e-3+t3505+t5357+t693.*(t71-t391)+t784.*(t71-t391)).*(-1.0./4.0);
t13395 = t17.*t13177.*1.13264871585e-2;
t13402 = t17.*t13182.*1.13264871585e-2;
t13405 = t9.*t13189.*1.13264871585e-2;
t13427 = t7613.*(t10158+t16.*(t4542-t6448)).*(-1.0./4.0);
t13428 = (t7613.*(t10158+t16.*(t4542-t6448)))./4.0;
t13431 = t7646.*(t10158+t16.*(t4542-t6448)).*(-1.0./4.0);
t13438 = (t7612.*t12296)./4.0;
t13439 = (t7622.*t12296)./4.0;
t13453 = (t10408.*t10546)./4.0;
t13456 = t9292.*(t3418-t3879+t4324-t5228+t5802+t9.*(t71-t391).*4.5305948634e-2+t17.*(t426-t581).*7.35522e-1).*(-1.0./2.0);
t13462 = -t13458;
t13464 = -t13459;
t13465 = (t10441.*t10554)./4.0;
t13479 = (t3421.*t13197)./4.0;
t13480 = t6761.*(t8610-t10439).*(-1.0./4.0);
t13484 = (t3489.*t13197)./4.0;
t13487 = (t6761.*(t8610-t10439))./4.0;
t13495 = (t9.*t7796.*t12296)./4.0;
t13497 = (t17.*t7797.*t12296)./4.0;
t13512 = t8.*t13380.*2.62925e-3;
t13515 = -t13507;
t13522 = t12296.*(t3479-t3544+t2772.*(t48-t349)+t2775.*(t48-t349)).*(-1.0./4.0);
t13523 = (t7796.*t12339)./4.0;
t13529 = (t12296.*(t3479-t3544+t2772.*(t48-t349)+t2775.*(t48-t349)))./4.0;
t13555 = (t7980.*t12296)./4.0;
t13564 = (t4021.*t13196)./4.0;
t13565 = t8062.*(t10158+t16.*(t4542-t6448)).*(-1.0./4.0);
t13569 = (t8062.*(t10158+t16.*(t4542-t6448)))./4.0;
t13570 = (t4024.*t13198)./4.0;
t13572 = -t13567;
t13575 = (t8070.*t12296)./4.0;
t13576 = t12296.*(t2752+t3814-t4385-t9.*t439.*3.127439544e-3).*(-1.0./4.0);
t13581 = (t12296.*(t2752+t3814-t4385-t9.*t439.*3.127439544e-3))./4.0;
t13600 = -t13597;
t13621 = -t13615;
t13645 = t8477.*(t10158+t16.*(t4542-t6448)).*(-1.0./4.0);
t13648 = (t8477.*(t10158+t16.*(t4542-t6448)))./4.0;
t13652 = (t8477.*t12296)./4.0;
t13658 = (t8497.*t12296)./4.0;
t13665 = t8562.*(t10158+t16.*(t4542-t6448)).*(-1.0./4.0);
t13669 = (t8562.*(t10158+t16.*(t4542-t6448)))./4.0;
t13678 = (t8547.*t12296)./4.0;
t13683 = ((t10158+t16.*(t4542-t6448)).*(t3063+t3528+t3966-t5230))./4.0;
t13684 = -t13679;
t13685 = t12296.*(-t3218+t3458+t3878+t8.*(t260+t468+t570+t2298).*1.666555).*(-1.0./4.0);
t13687 = (t12296.*(-t3218+t3458+t3878+t8.*(t260+t468+t570+t2298).*1.666555))./4.0;
t13693 = (t8600.*t12296)./4.0;
t13701 = t8640.*(t10158+t16.*(t4542-t6448)).*(-1.0./4.0);
t13705 = (t10546.*t10850)./4.0;
t13708 = (t8640.*t12296)./4.0;
t13712 = (t8654.*t12296)./4.0;
t13714 = (t10554.*t10858)./4.0;
t13717 = -t13715;
t13718 = -t13716;
t13720 = -t13719;
t13721 = (t10561.*t10871)./4.0;
t13728 = -t13723;
t13731 = (t5234.*t13196)./4.0;
t13733 = t8713.*(t10158+t16.*(t4542-t6448)).*(-1.0./4.0);
t13737 = (t5235.*t13198)./4.0;
t13751 = (t8709.*t12296)./4.0;
t13759 = (t10546.*t10931)./4.0;
t13763 = (t5433.*t13177)./4.0;
t13770 = t10561.*(t8963+t7.*(t5026+t5.*(t2959-t2967))).*(-1.0./4.0);
t13772 = t10554.*(t8963+t7.*(t5026+t5.*(t2959-t2967))).*(-1.0./4.0);
t13778 = (t10561.*(t8963+t7.*(t5026+t5.*(t2959-t2967))))./4.0;
t13781 = (t10554.*(t8963+t7.*(t5026+t5.*(t2959-t2967))))./4.0;
t13792 = -t13783;
t13843 = (t6872.*t12867)./4.0;
t13859 = (t5696.*t13197)./4.0;
t13870 = (t9028.*t12296)./4.0;
t13883 = -t13881;
t13894 = t6761.*(t8583-t11188).*(-1.0./4.0);
t13898 = t9106.*(t10158+t16.*(t4542-t6448)).*(-1.0./4.0);
t13899 = t9110.*(t10158+t16.*(t4542-t6448)).*(-1.0./4.0);
t13901 = t9112.*(t10158+t16.*(t4542-t6448)).*(-1.0./4.0);
t13902 = (t5235.*t13380)./4.0;
t13903 = (t9110.*(t10158+t16.*(t4542-t6448)))./4.0;
t13906 = (t9112.*(t10158+t16.*(t4542-t6448)))./4.0;
t13909 = -t13905;
t13912 = (t9098.*t12296)./4.0;
t13916 = (t9110.*t12296)./4.0;
t13917 = (t9112.*t12296)./4.0;
t13918 = (t10546.*t11228)./4.0;
t13929 = t9.*t8979.*t12296.*1.838805e-1;
t13930 = -t13924;
t13932 = t17.*t8981.*t12296.*1.838805e-1;
t13933 = (t10554.*t11247)./4.0;
t13942 = (t10561.*t11266)./4.0;
t13943 = -t13939;
t13972 = (t17.*t9185.*t12296)./4.0;
t13977 = (t9.*t9194.*t12296)./4.0;
t13985 = (t9194.*t12339)./4.0;
t13987 = (t6302.*t13197)./4.0;
t13988 = t9269.*(t10158+t16.*(t4542-t6448)).*(-1.0./4.0);
t13992 = (t9269.*(t10158+t16.*(t4542-t6448)))./4.0;
t13999 = (t12296.*(t3098+t3199+t3211-t3221+t3678+t4612))./4.0;
t14002 = (t9310.*t12296)./4.0;
t14026 = (t9505.*t12296)./4.0;
t14033 = -t14031;
t14034 = -t14032;
t14037 = -t14036;
t14046 = (t7079.*t13196)./4.0;
t14050 = t9743.*(t10158+t16.*(t4542-t6448)).*(-1.0./4.0);
t14051 = t9744.*(t10158+t16.*(t4542-t6448)).*(-1.0./4.0);
t14054 = ((t10158+t16.*(t4542-t6448)).*(-t3045-t3218+t3458+t3539+t3878+t8.*(t260+t468+t570+t2298).*1.666555))./4.0;
t14055 = (t9744.*(t10158+t16.*(t4542-t6448)))./4.0;
t14059 = (t10561.*t11720)./4.0;
t14060 = (t9717.*t12296)./4.0;
t14061 = (t7116.*t13198)./4.0;
t14066 = (t9744.*t12296)./4.0;
t14067 = -t14063;
t14068 = t12296.*(-t3045-t3218+t3458+t3539+t3878+t8.*(t260+t468+t570+t2298).*1.666555).*(-1.0./4.0);
t14072 = (t12296.*(-t3045-t3218+t3458+t3539+t3878+t8.*(t260+t468+t570+t2298).*1.666555))./4.0;
t14100 = -t14098;
t14101 = -t14099;
t14135 = (t7797.*t13177)./4.0;
t14136 = -t14132;
t14139 = (t7797.*t13182)./4.0;
t14145 = (t7796.*t13189)./4.0;
t14152 = (t10096.*t12296)./4.0;
t14158 = (t10111.*t12296)./4.0;
t14161 = t1992+t2480+t2616+t3584+t13531;
t14166 = (t7116.*t13380)./4.0;
t14167 = t10141.*(t10158+t16.*(t4542-t6448)).*(-1.0./4.0);
t14170 = (t10141.*(t10158+t16.*(t4542-t6448)))./4.0;
t14175 = -t14172;
t14179 = (t10141.*t12296)./4.0;
t14192 = t8.*t14112.*2.62925e-3;
t14194 = (t9194.*t12738)./4.0;
t14197 = -t14193;
t14199 = (t10546.*t12049)./4.0;
t14200 = t8.*t14057.*4.38178973375e-3;
t14202 = (t10554.*t12053)./4.0;
t14208 = -t14205;
t14211 = -t14210;
t14215 = (t10240.*t12296)./4.0;
t14222 = (t8191.*t13197)./4.0;
t14226 = (t9112.*t12867)./4.0;
t14234 = t8981.*(t8583-t11188).*(-1.0./4.0);
t14239 = (t8981.*(t8583-t11188))./4.0;
t14243 = t9.*t12296.*(t1987-t2621+t3452-t4730+t5359+t9.*(t71-t391).*6.1597e-2+t17.*(t426-t581)).*(-1.838805e-1);
t14246 = t9.*t12296.*(t1987-t2621+t3452-t4730+t5359+t9.*(t71-t391).*6.1597e-2+t17.*(t426-t581)).*1.838805e-1;
t14248 = (t10398.*t12296)./4.0;
t14256 = (t9.*t10468.*t12296)./4.0;
t14257 = (t17.*t10469.*t12296)./4.0;
t14263 = (t10561.*t12266)./4.0;
t14267 = -t14266;
t14272 = -t14270;
t14291 = (t4024.*t14112)./4.0;
t14292 = t9.*(t10174+t9.*(t10158+t16.*(t4542-t6448))).*(-1.13264871585e-2);
t14298 = t13380.*(-t1476-t1540+t2091+t2165+t2579+t8.*(t260+t468+t570+t2298)).*(-1.0./4.0);
t14300 = (t13380.*(-t1476-t1540+t2091+t2165+t2579+t8.*(t260+t468+t570+t2298)))./4.0;
t14313 = (t10546.*t12385)./4.0;
t14316 = (t10554.*t12385)./4.0;
t14319 = (t10546.*t12396)./4.0;
t14321 = (t10554.*t12396)./4.0;
t14323 = (t5069.*t14057)./4.0;
t14335 = -t14332;
t14339 = -t14336;
t14348 = t12867.*(-t3045-t3218+t3458+t3539+t3878+t8.*(t260+t468+t570+t2298).*1.666555).*(-1.0./4.0);
t14349 = (t12867.*(-t3045-t3218+t3458+t3539+t3878+t8.*(t260+t468+t570+t2298).*1.666555))./4.0;
t14360 = -t14355;
t14363 = t4298.*(t10174+t9.*(t10158+t16.*(t4542-t6448))).*(-1.0./4.0);
t14365 = (t10863.*t12296)./4.0;
t14366 = (t4298.*(t10174+t9.*(t10158+t16.*(t4542-t6448))))./4.0;
t14371 = ((t10158+t16.*(t4542-t6448)).*(t1589-t2213+t3195-t4346+t4355+t4748.*7.35522e-1+t2772.*(t71-t391)+t2775.*(t71-t391)))./4.0;
t14374 = (t5430.*t14057)./4.0;
t14380 = t3176+t3494+t14112;
t14382 = -t14379;
t14384 = t12296.*(t1589-t2213+t3195-t4346+t4355+t4748.*7.35522e-1+t2772.*(t71-t391)+t2775.*(t71-t391)).*(-1.0./4.0);
t14387 = (t12296.*(t1589-t2213+t3195-t4346+t4355+t4748.*7.35522e-1+t2772.*(t71-t391)+t2775.*(t71-t391)))./4.0;
t14392 = (t9185.*t13182)./4.0;
t14403 = (t5235.*t14112)./4.0;
t14406 = (t9194.*t13189)./4.0;
t14408 = -t14405;
t14411 = t3378+t3817+t3882+t4359+t13616;
t14429 = (t10550.*t12564)./4.0;
t14433 = (t10561.*t12564)./4.0;
t14436 = (t5919.*t14057)./4.0;
t14438 = (t5914.*t14057)./4.0;
t14442 = -t14437;
t14444 = -t14439;
t14445 = -t14441;
t14463 = -t14461;
t14476 = (t5433.*t14156)./4.0;
t14485 = -t14484;
t14486 = (t10468.*t12738)./4.0;
t14497 = t5433.*(t10174+t9.*(t10158+t16.*(t4542-t6448))).*(-1.0./4.0);
t14498 = t5434.*(t10174+t9.*(t10158+t16.*(t4542-t6448))).*(-1.0./4.0);
t14500 = (t5433.*(t10174+t9.*(t10158+t16.*(t4542-t6448))))./4.0;
t14501 = (t5434.*(t10174+t9.*(t10158+t16.*(t4542-t6448))))./4.0;
t14502 = t5449.*(t10174+t9.*(t10158+t16.*(t4542-t6448))).*(-1.0./4.0);
t14503 = (t5449.*(t10174+t9.*(t10158+t16.*(t4542-t6448))))./4.0;
t14534 = -t14529;
t14559 = (t6681.*t14057)./4.0;
t14565 = -t14561;
t14573 = -t14572;
t14575 = t9.*t12296.*(t3418-t3879+t4324-t5228+t5802+t9.*(t71-t391).*4.5305948634e-2+t17.*(t426-t581).*7.35522e-1).*(-1.0./4.0);
t14578 = (t9.*t12296.*(t3418-t3879+t4324-t5228+t5802+t9.*(t71-t391).*4.5305948634e-2+t17.*(t426-t581).*7.35522e-1))./4.0;
t14581 = t12339.*(t3418-t3879+t4324-t5228+t5802+t9.*(t71-t391).*4.5305948634e-2+t17.*(t426-t581).*7.35522e-1).*(-1.0./4.0);
t14590 = -t14587;
t14597 = -t14593;
t14598 = -t14594;
t14606 = -t14601;
t14608 = -t14604;
t14620 = t6397.*(t10174+t9.*(t10158+t16.*(t4542-t6448))).*(-1.0./4.0);
t14625 = (t6397.*(t10174+t9.*(t10158+t16.*(t4542-t6448))))./4.0;
t14628 = -t14624;
t14629 = -t14626;
t14652 = (t7116.*t14112)./4.0;
t14656 = -t14654;
t14665 = -t14662;
t14669 = -t14668;
t14672 = (t7612.*t14057)./4.0;
t14673 = (t7622.*t14057)./4.0;
t14679 = -t14675;
t14683 = -t14678;
t14687 = t6780.*(t10174+t9.*(t10158+t16.*(t4542-t6448))).*(-1.0./4.0);
t14688 = (t6780.*(t10174+t9.*(t10158+t16.*(t4542-t6448))))./4.0;
t14714 = (t10469.*t13177)./4.0;
t14717 = (t10469.*t13182)./4.0;
t14721 = (t10468.*t13189)./4.0;
t14726 = (t8070.*t14057)./4.0;
t14746 = -t14744;
t14750 = -t14748;
t14752 = t10959+t13027;
t14758 = t7538.*(t10174+t9.*(t10158+t16.*(t4542-t6448))).*(-1.0./4.0);
t14760 = (t7797.*t14156)./4.0;
t14763 = -t14759;
t14776 = -t14773;
t14792 = t14057.*(-t3218+t3458+t3878+t8.*(t260+t468+t570+t2298).*1.666555).*(-1.0./4.0);
t14793 = t14112.*(-t1476-t1540+t2091+t2165+t2579+t8.*(t260+t468+t570+t2298)).*(-1.0./4.0);
t14794 = t12738.*(t3418-t3879+t4324-t5228+t5802+t9.*(t71-t391).*4.5305948634e-2+t17.*(t426-t581).*7.35522e-1).*(-1.0./4.0);
t14795 = (t14057.*(-t3218+t3458+t3878+t8.*(t260+t468+t570+t2298).*1.666555))./4.0;
t14799 = -t14796;
t14806 = (t8600.*t14057)./4.0;
t14809 = t7796.*(t10174+t9.*(t10158+t16.*(t4542-t6448))).*(-1.0./4.0);
t14810 = t7797.*(t10174+t9.*(t10158+t16.*(t4542-t6448))).*(-1.0./4.0);
t14814 = (t7796.*(t10174+t9.*(t10158+t16.*(t4542-t6448))))./4.0;
t14818 = t7828.*(t10174+t9.*(t10158+t16.*(t4542-t6448))).*(-1.0./4.0);
t14822 = (t7828.*(t10174+t9.*(t10158+t16.*(t4542-t6448))))./4.0;
t14830 = t7913.*(t10174+t9.*(t10158+t16.*(t4542-t6448))).*(-1.0./4.0);
t14833 = (t7913.*(t10174+t9.*(t10158+t16.*(t4542-t6448))))./4.0;
t14847 = (t8709.*t14057)./4.0;
t14887 = t9.*(t13026+t17.*(t8963+t7.*(t5026+t5.*(t2959-t2967)))).*(-1.13264871585e-2);
t14888 = t8460.*(t10174+t9.*(t10158+t16.*(t4542-t6448))).*(-1.0./4.0);
t14889 = t9.*(t13026+t17.*(t8963+t7.*(t5026+t5.*(t2959-t2967)))).*1.13264871585e-2;
t14890 = (t8460.*(t10174+t9.*(t10158+t16.*(t4542-t6448))))./4.0;
t14901 = -t14899;
t14920 = (t9098.*t14057)./4.0;
t14961 = (t14057.*(t3098+t3199+t3211-t3221+t3678+t4612))./4.0;
t14968 = -t14966;
t14969 = -t14967;
t14972 = t9.*t14918.*1.539925e-2;
t14974 = t17.*t14919.*1.539925e-2;
t15000 = t13189.*(t3418-t3879+t4324-t5228+t5802+t9.*(t71-t391).*4.5305948634e-2+t17.*(t426-t581).*7.35522e-1).*(-1.0./4.0);
t15004 = t9048.*(t10174+t9.*(t10158+t16.*(t4542-t6448))).*(-1.0./4.0);
t15005 = ((t10174+t9.*(t10158+t16.*(t4542-t6448))).*(t3085-t3419-t3773+t5128+t17.*(t208-t427).*7.35522e-1))./4.0;
t15009 = (t9185.*t14156)./4.0;
t15031 = t9185.*(t10174+t9.*(t10158+t16.*(t4542-t6448))).*(-1.0./4.0);
t15033 = (t9185.*(t10174+t9.*(t10158+t16.*(t4542-t6448))))./4.0;
t15035 = t9194.*(t10174+t9.*(t10158+t16.*(t4542-t6448))).*(-1.0./4.0);
t15038 = (t9194.*(t10174+t9.*(t10158+t16.*(t4542-t6448))))./4.0;
t15047 = (t9717.*t14057)./4.0;
t15061 = (t3738.*t14918)./4.0;
t15064 = (t3743.*t14919)./4.0;
t15071 = t5434.*(t13026+t17.*(t8963+t7.*(t5026+t5.*(t2959-t2967)))).*(-1.0./4.0);
t15076 = (t5434.*(t13026+t17.*(t8963+t7.*(t5026+t5.*(t2959-t2967)))))./4.0;
t15079 = t9361.*(t10174+t9.*(t10158+t16.*(t4542-t6448))).*(-1.0./4.0);
t15083 = (t9361.*(t10174+t9.*(t10158+t16.*(t4542-t6448))))./4.0;
t15087 = t12792.*(t10158+t16.*(t4542-t6448)).*(-1.0./4.0);
t15091 = (t12792.*(t10158+t16.*(t4542-t6448)))./4.0;
t15103 = t12296.*(t3116+t3486+t3963+t11671.*1.666555).*(-1.0./4.0);
t15110 = (t12296.*(t3116+t3486+t3963+t11671.*1.666555))./4.0;
t15119 = t9537.*(t10174+t9.*(t10158+t16.*(t4542-t6448))).*(-1.0./4.0);
t15177 = t9896.*(t10174+t9.*(t10158+t16.*(t4542-t6448))).*(-1.0./4.0);
t15179 = (t9896.*(t10174+t9.*(t10158+t16.*(t4542-t6448))))./4.0;
t15198 = t16.*t10153.*t14057.*4.1663875e-1;
t15203 = -t15201;
t15205 = t16.*t14057.*(t6452-t8229).*(-4.1663875e-1);
t15207 = t16.*t14057.*(t6452-t8229).*4.1663875e-1;
t15230 = (t10607.*t14057)./4.0;
t15236 = (t14057.*(t8646-t8.*(t30.*(t2425-t2468)+t68.*(t2425-t2468)).*1.666555))./4.0;
t15240 = t13198.*(t10158+t16.*(t4542-t6448)).*(-1.0./4.0);
t15245 = (t13198.*(t10158+t16.*(t4542-t6448)))./4.0;
t15248 = (t12296.*t13196)./4.0;
t15250 = (t12296.*t13197)./4.0;
t15267 = (t10469.*t14156)./4.0;
t15273 = t10446.*(t10174+t9.*(t10158+t16.*(t4542-t6448))).*(-1.0./4.0);
t15276 = (t10446.*(t10174+t9.*(t10158+t16.*(t4542-t6448))))./4.0;
t15279 = t10468.*(t10174+t9.*(t10158+t16.*(t4542-t6448))).*(-1.0./4.0);
t15280 = t10469.*(t10174+t9.*(t10158+t16.*(t4542-t6448))).*(-1.0./4.0);
t15281 = (t10468.*(t10174+t9.*(t10158+t16.*(t4542-t6448))))./4.0;
t15282 = (t10469.*(t10174+t9.*(t10158+t16.*(t4542-t6448))))./4.0;
t15284 = t10480.*(t10174+t9.*(t10158+t16.*(t4542-t6448))).*(-1.0./4.0);
t15290 = ((t10174+t9.*(t10158+t16.*(t4542-t6448))).*(t2740+t3849+t3968+t3972-t5255+t17.*(t260+t468+t570+t2298).*7.35522e-1))./4.0;
t15311 = t13333.*(t10158+t16.*(t4542-t6448)).*(-1.0./4.0);
t15317 = (t12296.*t13326)./4.0;
t15323 = t7796.*(t13026+t17.*(t8963+t7.*(t5026+t5.*(t2959-t2967)))).*(-1.0./4.0);
t15326 = (t7796.*(t13026+t17.*(t8963+t7.*(t5026+t5.*(t2959-t2967)))))./4.0;
t15346 = t13380.*(t10158+t16.*(t4542-t6448)).*(-1.0./4.0);
t15348 = -t15347;
t15350 = (t12296.*t13376)./4.0;
t15354 = (t6761.*t14919)./4.0;
t15356 = -t15351;
t15357 = (t6811.*t14918)./4.0;
t15364 = -t15361;
t15377 = t10753.*(t10174+t9.*(t10158+t16.*(t4542-t6448))).*(-1.0./4.0);
t15385 = t10787.*(t10174+t9.*(t10158+t16.*(t4542-t6448))).*(-1.0./4.0);
t15388 = (t10787.*(t10174+t9.*(t10158+t16.*(t4542-t6448))))./4.0;
t15408 = -t15406;
t15410 = (t11341.*t14057)./4.0;
t15412 = (t11338.*(-t1476+t2165+t13876))./4.0;
t15415 = (t12296.*t13578)./4.0;
t15419 = t14057.*(t6847-t9563).*(-1.0./4.0);
t15422 = t10612.*(t249-t391.*(1.1e+1./1.25e+2)-t1912.*4.252e-3+t3505+t13496+t693.*(t71-t391)+t784.*(t71-t391)).*(-1.0./4.0);
t15423 = (t11380.*t14057)./4.0;
t15424 = (t11372.*(-t1476+t2165+t13876))./4.0;
t15426 = t14057.*(t8589-t8592).*(-1.0./4.0);
t15435 = t13627.*(t10158+t16.*(t4542-t6448)).*(-1.0./4.0);
t15438 = (t13627.*(t10158+t16.*(t4542-t6448)))./4.0;
t15441 = (t12296.*(t3098+t3211-t3221+t3678+t8102+t10798))./4.0;
t15450 = -t15448;
t15458 = t9194.*(t13026+t17.*(t8963+t7.*(t5026+t5.*(t2959-t2967)))).*(-1.0./4.0);
t15459 = (t9194.*(t13026+t17.*(t8963+t7.*(t5026+t5.*(t2959-t2967)))))./4.0;
t15463 = -t15462;
t15467 = ((t10174+t9.*(t10158+t16.*(t4542-t6448))).*(t3418-t3879+t4324-t5228+t5802+t9.*(t71-t391).*4.5305948634e-2+t17.*(t426-t581).*7.35522e-1))./4.0;
t15470 = t11483.*(t10174+t9.*(t10158+t16.*(t4542-t6448))).*(-1.0./4.0);
t15471 = (t11483.*(t10174+t9.*(t10158+t16.*(t4542-t6448))))./4.0;
t15486 = (t12296.*t13915)./4.0;
t15489 = (t8979.*t14918)./4.0;
t15490 = -t15488;
t15494 = (t8981.*t14919)./4.0;
t15499 = -t15495;
t15503 = (t10942.*(-t3045+t3539+t14113))./4.0;
t15507 = (t12296.*t13974)./4.0;
t15508 = t11340.*(t249-t391.*(1.1e+1./1.25e+2)-t1912.*4.252e-3+t3505+t13496+t693.*(t71-t391)+t784.*(t71-t391)).*(-1.0./4.0);
t15509 = -t15506;
t15513 = ((t6834-t9565).*(t249-t391.*(1.1e+1./1.25e+2)-t1912.*4.252e-3+t3505+t13496+t693.*(t71-t391)+t784.*(t71-t391)))./4.0;
t15514 = t11377.*(t249-t391.*(1.1e+1./1.25e+2)-t1912.*4.252e-3+t3505+t13496+t693.*(t71-t391)+t784.*(t71-t391)).*(-1.0./4.0);
t15526 = t2076+t2621+t15451;
t15527 = (t12296.*t14035)./4.0;
t15541 = t14112.*(t10158+t16.*(t4542-t6448)).*(-1.0./4.0);
t15543 = (t14112.*(t10158+t16.*(t4542-t6448)))./4.0;
t15545 = (t12296.*t14113)./4.0;
t15551 = -t15549;
t15575 = t10468.*(t13026+t17.*(t8963+t7.*(t5026+t5.*(t2959-t2967)))).*(-1.0./4.0);
t15576 = (t10468.*(t13026+t17.*(t8963+t7.*(t5026+t5.*(t2959-t2967)))))./4.0;
t15593 = t12296.*(t4401+t4424+t9457-t11860).*(-1.0./4.0);
t15594 = (t12296.*(t4401+t4424+t9457-t11860))./4.0;
t15604 = t14918.*(t1987-t2621+t3452-t4730+t5359+t9.*(t71-t391).*6.1597e-2+t17.*(t426-t581)).*(-1.0./4.0);
t15615 = t14057.*(t3116+t3486+t3963+t11671.*1.666555).*(-1.0./2.0);
t15617 = (t14057.*(t3116+t3486+t3963+t11671.*1.666555))./2.0;
t15627 = (t10158+t16.*(t4542-t6448)).*(-t3045+t3539+t14113).*(-1.0./4.0);
t15629 = ((t10158+t16.*(t4542-t6448)).*(-t3045+t3539+t14113))./4.0;
t15632 = (t12296.*(-t3045+t3539+t14113))./4.0;
t15647 = t3460+t3879+t15536;
t15685 = (t13196.*t14057)./2.0;
t15686 = (t13198.*(-t1476+t2165+t13876))./2.0;
t15697 = (t13326.*t14057)./2.0;
t15707 = (t13376.*t14057)./2.0;
t15708 = (t13380.*(-t1476+t2165+t13876))./2.0;
t15724 = (t12867.*(-t3045+t3539+t14113))./2.0;
t15736 = ((t10158+t16.*(t4542-t6448)).*(t1589-t2213-t4346+t4355+t9454+t11863+t2772.*(t71-t391)+t2775.*(t71-t391)))./4.0;
t15738 = t12296.*(t1589-t2213-t4346+t4355+t9454+t11863+t2772.*(t71-t391)+t2775.*(t71-t391)).*(-1.0./4.0);
t15747 = -t15746;
t15750 = (t14057.*(t3098+t3211-t3221+t3678+t8102+t10798))./2.0;
t15752 = t13197.*(t249-t391.*(1.1e+1./1.25e+2)-t1912.*4.252e-3+t3505+t13496+t693.*(t71-t391)+t784.*(t71-t391)).*(-1.0./2.0);
t15757 = -t15754;
t15758 = -t15755;
t15808 = t9922.*(t2091+t2497+t2579+t2680+t3516+t9.*(t210+t2107+t7423+t9121)+t17.*(t9166-t11658)).*(-1.0./4.0);
t15812 = (t14057.*t14113)./2.0;
t15813 = (t14112.*(-t1476+t2165+t13876))./2.0;
t15820 = t8743.*(t3418-t3879+t4324+t11855+t9.*(t71-t391).*4.5305948634e-2+t17.*(t426-t581).*7.35522e-1+t9.*(t9166-t11658).*7.35522e-1).*(-1.0./4.0);
t15821 = (t8743.*(t3418-t3879+t4324+t11855+t9.*(t71-t391).*4.5305948634e-2+t17.*(t426-t581).*7.35522e-1+t9.*(t9166-t11658).*7.35522e-1))./4.0;
t15826 = -t15823;
t15827 = t10446.*(t1987-t2621+t3452+t11654+t9.*(t71-t391).*6.1597e-2+t17.*(t426-t581)+t9.*(t9166-t11658)).*(-1.0./4.0);
t15828 = -t15824;
t15829 = (t10446.*(t1987-t2621+t3452+t11654+t9.*(t71-t391).*6.1597e-2+t17.*(t426-t581)+t9.*(t9166-t11658)))./4.0;
t15837 = -t15836;
t15841 = -t15840;
t15846 = -t15845;
t15859 = t9292.*(t3418-t3879+t4324+t11855+t9.*(t71-t391).*4.5305948634e-2+t17.*(t426-t581).*7.35522e-1+t9.*(t9166-t11658).*7.35522e-1).*(-1.0./4.0);
t15862 = (t9292.*(t3418-t3879+t4324+t11855+t9.*(t71-t391).*4.5305948634e-2+t17.*(t426-t581).*7.35522e-1+t9.*(t9166-t11658).*7.35522e-1))./4.0;
t15863 = -t15860;
t15864 = -t15861;
t15876 = t11484.*(t2091+t2497+t2579+t2680+t3516+t9.*(t210+t2107+t7423+t9121)+t17.*(t9166-t11658)).*(-1.0./4.0);
t15911 = t17.*t12296.*(t2091+t2497+t2579+t2680+t3516+t9.*(t210+t2107+t7423+t9121)+t17.*(t9166-t11658)).*(-1.838805e-1);
t15912 = t9.*t12296.*(t1987-t2621+t3452+t11654+t9.*(t71-t391).*6.1597e-2+t17.*(t426-t581)+t9.*(t9166-t11658)).*(-1.838805e-1);
t15913 = t17.*t12296.*(t2091+t2497+t2579+t2680+t3516+t9.*(t210+t2107+t7423+t9121)+t17.*(t9166-t11658)).*1.838805e-1;
t15914 = t9.*t12296.*(t1987-t2621+t3452+t11654+t9.*(t71-t391).*6.1597e-2+t17.*(t426-t581)+t9.*(t9166-t11658)).*1.838805e-1;
t15915 = ((t8610-t10439).*(t2091+t2497+t2579+t2680+t3516+t9.*(t210+t2107+t7423+t9121)+t17.*(t9166-t11658)))./4.0;
t15937 = ((t10174+t9.*(t10158+t16.*(t4542-t6448))).*(t3543+t3820+t3911+t3949+t4360+t12067+t17.*(t258+t2289+t5392+t7559).*7.35522e-1))./4.0;
t15948 = t14918.*(t10174+t9.*(t10158+t16.*(t4542-t6448))).*(-1.0./4.0);
t15964 = ((t8583-t11188).*(t2091+t2497+t2579+t2680+t3516+t9.*(t210+t2107+t7423+t9121)+t17.*(t9166-t11658)))./4.0;
t15970 = t17.*t12296.*(t3423+t3845+t3888+t3925+t4339+t9.*(t210+t2107+t7423+t9121).*7.35522e-1+t17.*(t9166-t11658).*7.35522e-1).*(-1.0./4.0);
t15971 = (t17.*t12296.*(t3423+t3845+t3888+t3925+t4339+t9.*(t210+t2107+t7423+t9121).*7.35522e-1+t17.*(t9166-t11658).*7.35522e-1))./4.0;
t15972 = t9.*t12296.*(t3418-t3879+t4324+t11855+t9.*(t71-t391).*4.5305948634e-2+t17.*(t426-t581).*7.35522e-1+t9.*(t9166-t11658).*7.35522e-1).*(-1.0./4.0);
t15973 = (t9.*t12296.*(t3418-t3879+t4324+t11855+t9.*(t71-t391).*4.5305948634e-2+t17.*(t426-t581).*7.35522e-1+t9.*(t9166-t11658).*7.35522e-1))./4.0;
t15974 = t12339.*(t3418-t3879+t4324+t11855+t9.*(t71-t391).*4.5305948634e-2+t17.*(t426-t581).*7.35522e-1+t9.*(t9166-t11658).*7.35522e-1).*(-1.0./4.0);
t15978 = t15088.*(t10174+t9.*(t10158+t16.*(t4542-t6448))).*(-1.0./4.0);
t15979 = (t15088.*(t10174+t9.*(t10158+t16.*(t4542-t6448))))./4.0;
t15985 = -t15983;
t15989 = t15155.*(t10174+t9.*(t10158+t16.*(t4542-t6448))).*(-1.0./4.0);
t15990 = (t15155.*(t10174+t9.*(t10158+t16.*(t4542-t6448))))./4.0;
t16012 = t12738.*(t3418-t3879+t4324+t11855+t9.*(t71-t391).*4.5305948634e-2+t17.*(t426-t581).*7.35522e-1+t9.*(t9166-t11658).*7.35522e-1).*(-1.0./4.0);
t16020 = t13177.*(t3423+t3845+t3888+t3925+t4339+t9.*(t210+t2107+t7423+t9121).*7.35522e-1+t17.*(t9166-t11658).*7.35522e-1).*(-1.0./4.0);
t16022 = (t13177.*(t3423+t3845+t3888+t3925+t4339+t9.*(t210+t2107+t7423+t9121).*7.35522e-1+t17.*(t9166-t11658).*7.35522e-1))./4.0;
t16023 = t13182.*(t3423+t3845+t3888+t3925+t4339+t9.*(t210+t2107+t7423+t9121).*7.35522e-1+t17.*(t9166-t11658).*7.35522e-1).*(-1.0./4.0);
t16025 = (t13182.*(t3423+t3845+t3888+t3925+t4339+t9.*(t210+t2107+t7423+t9121).*7.35522e-1+t17.*(t9166-t11658).*7.35522e-1))./4.0;
t16026 = t13189.*(t3418-t3879+t4324+t11855+t9.*(t71-t391).*4.5305948634e-2+t17.*(t426-t581).*7.35522e-1+t9.*(t9166-t11658).*7.35522e-1).*(-1.0./4.0);
t16027 = (t13189.*(t3418-t3879+t4324+t11855+t9.*(t71-t391).*4.5305948634e-2+t17.*(t426-t581).*7.35522e-1+t9.*(t9166-t11658).*7.35522e-1))./4.0;
t16035 = ((t10174+t9.*(t10158+t16.*(t4542-t6448))).*(t3845+t3925+t4339+t9.*(t210+t2107+t7423+t9121).*7.35522e-1+t17.*(t9166-t11658).*7.35522e-1))./4.0;
t16055 = t14156.*(t3423+t3845+t3888+t3925+t4339+t9.*(t210+t2107+t7423+t9121).*7.35522e-1+t17.*(t9166-t11658).*7.35522e-1).*(-1.0./2.0);
t16061 = ((t10174+t9.*(t10158+t16.*(t4542-t6448))).*(t3423+t3845+t3888+t3925+t4339+t9.*(t210+t2107+t7423+t9121).*7.35522e-1+t17.*(t9166-t11658).*7.35522e-1))./4.0;
t16062 = ((t10174+t9.*(t10158+t16.*(t4542-t6448))).*(t3418-t3879+t4324+t11855+t9.*(t71-t391).*4.5305948634e-2+t17.*(t426-t581).*7.35522e-1+t9.*(t9166-t11658).*7.35522e-1))./4.0;
t16080 = -t16079;
t16082 = -t16081;
t16087 = t14918.*(t1987-t2621+t3452+t11654+t9.*(t71-t391).*6.1597e-2+t17.*(t426-t581)+t9.*(t9166-t11658)).*(-1.0./2.0);
t16088 = t14919.*(t2091+t2497+t2579+t2680+t3516+t9.*(t210+t2107+t7423+t9121)+t17.*(t9166-t11658)).*(-1.0./2.0);
t16090 = (t14918.*(t1987-t2621+t3452+t11654+t9.*(t71-t391).*6.1597e-2+t17.*(t426-t581)+t9.*(t9166-t11658)))./2.0;
t16095 = ((t13026+t17.*(t8963+t7.*(t5026+t5.*(t2959-t2967)))).*(t3418-t3879+t4324+t11855+t9.*(t71-t391).*4.5305948634e-2+t17.*(t426-t581).*7.35522e-1+t9.*(t9166-t11658).*7.35522e-1))./2.0;
t16108 = -t16106;
t16111 = -t16110;
t16120 = t3825+t3853+t3990+t4067+t4099+t4144+t4160+t4186+t4191+t4192+t4273+t4372+t4423+t5547+t5682+t6603+t6632+t6671+t6773+t7738+t7781+t7999+t8214+t8343+t8365+t8418+t9206+t9519+t9530;
t16121 = t3855+t3902+t3990+t4067+t4125+t4133+t4144+t4191+t4192+t4220+t4292+t4393+t4403+t5547+t5682+t6603+t6632+t6671+t6773+t7738+t7781+t7999+t8214+t8343+t8365+t8418+t9206+t9519+t9530;
t16122 = -q3d.*(t3825+t3853-t3990-t4067+t4099+t4153+t4160+t4186+t4273+t4372+t4423-t5547+t5671+t6595+t6623-t6671-t6773-t7738-t7781+t7992-t8214+t8334+t8354+t8404-t9519-t9530+(t3239.*(t79-t358))./4.0+(t3280.*(t79-t358))./4.0+(t8640.*(t701-t775))./4.0);
t16123 = t6607+t6866+t6958+t8144+t8271+t10847+t11562+t12109+t12111+t12394+t12395;
t16128 = t3246+t3276+t4061+t4076+t4093+t4101+t4123+t4128+t4149+t4198+t4204+t4216+t4249+t4314+t4987+t5020+t5602+t5695+t5703+t6706+t6797+t7553+t8183+t8252+t8277+t8371+t8395+t8411+t8870+t8916+t9242+t9642+t9652;
t16130 = t5400+t5539+t5540+t5796+t5949+t6070+t6141+t6224+t6931+t6949+t7075+t8179+t8201+t8525+t8546+t9075+t9150+t9637+t9726+t10231+t10261+t10662+t10702;
t16133 = t4142+t4173+t4230+t4274+t4443+t4577+t4620+t4639+t4676+t4717+t4806+t5568+t5608+t6288+t6364+t7479+t7557+t8596+t8696+t8702+t8843+t9424+t9447+t9460+t9673+t9675+t10705+t10733+t10734;
t16134 = -q2d.*(t4230+t4248-t4443-t4577+t4593+t4639+t4676+t4717+t4806-t5568+t5585+t6288+t6364+t7479+t7557+t8596+t8696+t8702+t8843+t9424+t9447+t9460+t9673+t9675+t10705+t10733+t10734+t9.*(t208-t427).*3.867742437e-3+t17.*(t208-t427).*1.563719772e-3);
t16137 = t3755+t3777+t3804+t3826+t3854+t3858+t4158+t4161+t4187+t4272+t4394+t4404+t5537+t5564+t5693+t5724+t5748+t5797+t6226+t6283+t6816+t7024+t9276+t9483+t9492+t9506+t9625+t9654+t9691+t9711+t9918+t9950+t10167+t10190;
t16140 = t3674+t3725+t4299+t4368+t4370+t4449+t4465+t4487+t4832+t4838+t5008+t5031+t5042+t5053+t5303+t5394+t6299+t6400+t6407+t7506+t7601+t8249+t8803+t9467+t9588+t9589+t9754+t9766+t10062+t10073+t10727+t10806+t10809;
t16141 = t3674+t3725+t4277+t4368+t4370+t4449+t4465+t4487+t4817+t4823+t5008+t5031+t5042+t5053+t5313+t5380+t6316+t6414+t6419+t7516+t7587+t8265+t8818+t9453+t9582+t9596+t9758+t9762+t10065+t10069+t10721+t10803+t10811;
t16142 = -q2d.*(-t3674-t3725+t4277+t4347+t4353+t4442-t4449+t4817+t4823-t5008+t5022-t5031-t5053+t5313+t5380+t6316+t6414+t6419+t7516+t7587+t8265+t8818+t9453+t9582+t9596+t9758+t9762+t10065+t10069+t10721+t10803+t10811-t16.*t321.*2.454825983680473e-3);
t16143 = t3673+t3746+t3749+t4622+t4642+t4844+t4966+t5013+t5977+t6055+t6056+t6130+t6131+t6286+t6334+t6436+t6679+t6718+t6783+t6994+t7060+t7170+t7181+t8168+t8199+t8511+t8527+t8809+t9232+t10282+t10283+t10530+t10540+t10773+t10776;
t16144 = -q3d.*(t3633+t3726-t3746+t4595-t4642+t4830-t4966+t4993-t5977+t6037-t6056-t6130-t6131+t6269-t6334-t6679+t6697+t6774+t6978-t7060-t7170+t7175-t8168+t8180-t8511+t8521-t8809-t9232+t10278+t10279+t10520-t10540+t10771-t10776+(t5990.*(t79-t358))./2.0);
t16149 = q2d.*t16148;
t16152 = t3995+t4013+t4190+t4197+t4271+t4313+t4437+t4467+t4543+t4560+t5106+t5166+t5688+t5927+t6018+t6425+t6439+t6494+t6507+t6566+t7652+t7772+t9677+t10258+t10457+t10565+t10581+t10760+t10761+t10844+t10851+t11160+t11240+t11242;
t16155 = t4014+t4034+t4223+t4227+t4291+t4306+t4448+t4462+t4520+t4539+t5127+t5140+t5688+t5927+t6018+t6425+t6439+t6494+t6507+t6566+t7652+t7772+t9677+t10258+t10457+t10565+t10581+t10760+t10761+t10844+t10851+t11160+t11240+t11242;
t16159 = t2443+t2487+t3485+t3570+t4596+t4601+t4621+t4671+t4683+t4705+t4746+t5231+t5976+t5978+t6142+t6164+t6168+t6169+t6194+t6210+t6932+t7049+t7087+t7098+t7157+t7174+t7188+t7205+t7518+t7544+t8739+t8746+t8749+t8755+t9576+t9805+t10305+t10309+t10927+t10928+t10944+t10945;
t16161 = t4205+t4237+t4290+t4348+t4354+t4488+t4659+t4688+t5055+t5068+t5558+t5588+t6012+t6285+t6346+t6525+t6537+t6601+t7295+t7457+t7844+t7912+t9953+t10352+t10563+t11210+t11219+t11264+t11304+t11317+t11567+t11585+t11625+t11646;
t16167 = t3683+t3711+t3905+t3992+t4002+t4004+t4012+t4015+t4070+t4083+t4138+t4151+t4177+t4852+t4878+t4885+t4951+t4976+t5059+t5370+t5399+t5595+t5618+t5654+t5697+t5735+t5948+t6006+t6007+t6089+t6217+t6218+t6488+t6489+t6703+t6730+t6819+t6959+t6979+t7019+t7191+t7419+t7420+t7425+t7630+t8036+t8288+t8290+t8308+t8439+t8783+t8787+t8930+t8943+t9010+t9017+t9019+t9164+t9251+t9923+t9930;
t16176 = q2d.*t16175;
t16182 = -q3d.*(t3775+t3786+t3787+t3920+t4029+t4037+t4091+t4106+t4132+t4182+t4207+t4240+t4247-t4891-t4926+t4961+t5036+t5146-t5372-t5398+t5421-t5678-t5816-t5817+t6004+t6023-t6086+t6705+t6722+t6754+t6842+t6882+t7285-t7298-t7325-t7333+t7431+t7447+t7678-t7716-t7729+t7762-t7766-t7770-t8247+t8489-t8744+t9018+t9027+t9191+t9282+t9287+t9461+t9479+t9493-t9516-t9517-t9646-t9671-t9683+t10135+t10136-(t9.*t323.*t5763)./4.0-(t17.*t323.*t5837)./4.0);
t16189 = t2651+t3719+t3727+t4078+t4686+t4845+t4894+t4923+t4929+t5319+t5818+t5901+t5984+t6284+t6298+t6303+t6445+t6473+t6626+t6627+t6830+t7097+t7117+t7264+t7522+t7608+t7774+t7893+t7990+t8674+t8978+t8988+t9262+t9272+t9303+t10462+t10470+t10496+t10683+t10687+t10849+t11810+t11938+t12401+t12402+t12403+t12405;
t16190 = q2d.*(-t2608+t3719+t3727+t4078+t4686+t4845+t4894+t4923+t4929+t5319+t5818+t5901+t5984+t6284+t6298+t6303+t6445+t6473+t6626+t6627+t6830+t7097+t7117+t7264+t7522+t7608+t7774+t7893+t7990+t8674+t8978+t8988+t9262+t9272+t9303+t10462+t10470+t10496+t10683+t10687+t10849+t11810+t11938+t12401+t12402+t12403+t12405);
t16197 = t3979+t4031+t4174+t4202+t4213+t4235+t4244+t4302+t4406+t4411+t4445+t4502+t4973+t4975+t5003+t5005+t5025+t5058+t5346+t5354+t5692+t5715+t6081+t6097+t6173+t6630+t6707+t6798+t6815+t6914+t6916+t7460+t7509+t7515+t7600+t7993+t8041+t8173+t8190+t8339+t8378+t8496+t8642+t8644+t8996+t9173+t9207+t9219+t9407+t9433+t9466+t9737+t9745+t9789+t9804+t9924+t10115+t10229+t10238+t10726+t11016+t11018;
t16198 = t3979+t4010+t4202+t4206+t4213+t4244+t4261+t4302+t4375+t4382+t4418+t4519+t4975+t4983+t4989+t5003+t5025+t5058+t5346+t5354+t5692+t5715+t6081+t6097+t6173+t6640+t6691+t6798+t6815+t6914+t6916+t7460+t7509+t7515+t7600+t7993+t8041+t8173+t8190+t8339+t8378+t8496+t8636+t8650+t8996+t9179+t9207+t9219+t9407+t9433+t9466+t9737+t9745+t9790+t9802+t9924+t10119+t10229+t10238+t10726+t11016+t11018;
t16217 = t3863+t3903+t4054+t4060+t4137+t4199+t4211+t4243+t4258+t4262+t4285+t4340+t4345+t4564+t4615+t5061+t5082+t5091+t5402+t5428+t5706+t5714+t5744+t6100+t6238+t6255+t6290+t6311+t6323+t6843+t6869+t6975+t7070+t7530+t7539+t7636+t8058+t8459+t8524+t8723+t8724+t8770+t8772+t8831+t8835+t8933+t8973+t9076+t9614+t9624+t9773+t9935+t9973+t10013+t10127+t10131+t10299+t10301+t10328+t10466+t10473+t10629+t10665+t10821+t11175+t11190;
t16237 = t3402+t3406+t3511+t3547+t3554+t3608+t3690+t3722+t3729+t3737+t3906+t3994+t4041+t4051+t4096+t4562+t4603+t4677+t4708+t4799+t4800+t4809+t4853+t4855+t4861+t4899+t4932+t4933+t4934+t5000+t5060+t5426+t5447+t5756+t5769+t5942+t5968+t5970+t5972+t6003+t6010+t6028+t6039+t6105+t6106+t6113+t6115+t6160+t6167+t6172+t6214+t6221+t6262+t6312+t6520+t6665+t6667+t6736+t6753+t6785+t6833+t6954+t7025+t7162+t7222+t7244+t7354+t7356+t7466+t7577+t7710+t7721+t7724+t7727+t8133+t8167+t8216+t8235+t8665+t8757+t8764+t9065+t9188+t9731+t9735+t9795+t9803+t9853+t9858+t9997+t10008+t10051+t10113+t10128+t10171+t10365+t10387;
t16239 = t4065+t4081+t4136+t4175+t4210+t4234+t4278+t4376+t4419+t4669+t4687+t4974+t5006+t5563+t5704+t5728+t5734+t5854+t5855+t5961+t6264+t6332+t6336+t6368+t6399+t6409+t6456+t7052+t7062+t7071+t7109+t7155+t7464+t7537+t7684+t7717+t7798+t9214+t9222+t9230+t9231+t9279+t9306+t9340+t9486+t9489+t9612+t9668+t9792+t10039+t10047+t10066+t10132+t10449+t10494+t10680+t10745+t10748+t10929+t10952+t11042+t11323+t11328+t11332+t11352+t11682+t11686;
t16240 = -q2d.*(-t4065-t4081-t4136-t4175+t4180-t4234-t4376-t4419-t4974+t4990+t5545+t5691+t5718+t5745+t5865+t5867+t5941+t6282+t6348+t6352+t6388+t6398+t6412+t6464+t7033+t7076+t7086+t7122+t7167+t7455-t7537+t7669+t7698+t7782+t9221+t9235+t9243+t9246+t9286+t9295+t9329-t9486-t9489-t9612+t9660+t9807+t10027+t10035+t10077+t10126+t10458+t10492-t10680-t10745-t10748+t10935+t10958+t11034+t11313+t11318+t11337+t11357+t11680+t11684+(t1837.*(t689-t740))./4.0+(t3286.*(t60-t394))./4.0+(t3239.*(t357-t519))./4.0);
t16241 = t4065+t4081+t4136+t4175+t4210+t4234+t4278+t4376+t4419+t4669+t4687+t4974+t5006+t5545+t5691+t5718+t5745+t5865+t5867+t5941+t6282+t6348+t6352+t6388+t6398+t6412+t6464+t7033+t7076+t7086+t7122+t7167+t7464+t7537+t7669+t7698+t7782+t9221+t9235+t9243+t9246+t9286+t9295+t9329+t9486+t9489+t9612+t9660+t9807+t10027+t10035+t10077+t10126+t10458+t10492+t10680+t10745+t10748+t10935+t10958+t11034+t11313+t11318+t11337+t11357+t11680+t11684;
t16243 = -phid.*(t7842+t8174+t8286+t9182+t9210+t15012+t15215+t16106-t16107-t16109+t16110);
t16258 = t4001+t4040+t4652+t4658+t4762+t4785+t4804+t4840+t5267+t5296+t5773+t5803+t7148+t7195+t7207+t8626+t8682+t8881+t9257+t12013+t12015+t12020+t12023+t14549+t14869+t15554+t15558+t15597+t15601+t15608+t15610+t15669+t15670;
t16259 = -phid.*(-t4652-t4658+t4757+t4840+t5267+t5296+t5773+t5803+t7148+t7195+t7207+t8626+t8682+t8881+t9257+t12008+t12014+t12018+t14549+t14869+t15554+t15558+t15597+t15601+t15608+t15610+t15669+t15670+t8.*t11672.*3.867742437e-3+t2963.*(t71-t391)+t3167.*(t71-t391)+t4080.*(t71-t391)+t4130.*(t71-t391));
t16260 = t3687+t3745+t3778+t3781+t3791+t3805+t3813+t3815+t3827+t3945+t4028+t4036+t4104+t4118+t4157+t4870+t4895+t4942+t4944+t4949+t5035+t5067+t5092+t5145+t5258+t5306+t5702+t5742+t5758+t5780+t5839+t6068+t6082+t6122+t6165+t6166+t6289+t6386+t6465+t6511+t6548+t6574+t6588+t6732+t6759+t6812+t6868+t6874+t6877+t6923+t6925+t6989+t7023+t7095+t7529+t7625+t7628+t7634+t7638+t7641+t7773+t8043+t8056+t8110+t8536+t8545+t8551+t8559+t8775+t8805+t8838+t8851+t8884+t8888+t9016+t9081+t9095+t9107+t9176+t9609+t9622+t9844+t9859+t9968+t9996+t10474+t10486+t10694+t10697+t10731+t10737+t10800+t10813+t10876+t11153+t11159+t11305+t11448+t11449;
t16261 = t3708+t3745+t3753+t3779+t3781+t3791+t3813+t3827+t3842+t3918+t4028+t4036+t4104+t4118+t4157+t4857+t4909+t4942+t4953+t4960+t5035+t5049+t5072+t5145+t5244+t5316+t5689+t5732+t5746+t5788+t5856+t6051+t6095+t6122+t6165+t6184+t6272+t6403+t6457+t6522+t6556+t6579+t6582+t6719+t6746+t6786+t6836+t6892+t6899+t6923+t6925+t6989+t7023+t7095+t7545+t7606+t7621+t7643+t7653+t7660+t7759+t8043+t8068+t8093+t8536+t8543+t8545+t8570+t8765+t8821+t8822+t8871+t8888+t8908+t9020+t9077+t9108+t9114+t9176+t9609+t9622+t9835+t9868+t9968+t10003+t10474+t10486+t10698+t10706+t10736+t10744+t10792+t10812+t10875+t11166+t11171+t11299+t11451+t11453;
t16263 = t4407+t4421+t4425+t4429+t4481+t4483+t4903+t4904+t6030+t6420+t6486+t6964+t7008+t7213+t7269+t7308+t8685+t8735+t9991+t9999+t10133+t10713+t12542+t12543+t14813+t15002+t15643+t15648+t15656+t15658+t15681+t15683+t15711+t15713;
t16269 = t4279+t4301+t4305+t4485+t4490+t4518+t4805+t4821+t6392+t6620+t6696+t7394+t7411+t7474+t7814+t7899+t8762+t8866+t10388+t10784+t10943+t10951+t12578+t12579+t14852+t15026+t15693+t15695+t15715+t15716+t15732+t15733+t15749+t15753;
t16281 = t4503+t4613+t4616+t4732+t4747+t4759+t5010+t5023+t6965+t7270+t7384+t7472+t7744+t7785+t8540+t8593+t9007+t9038+t10280+t10284+t11218+t11933+t12212+t12224+t14925+t15123+t15778+t15780+t15783+t15784+t15795+t15797+t15802+t15803;
t16282 = -phid.*(t4484+t4576+t4580+t4749+t4773+t4786+t5002+t5030-t6965+t7258-t7472-t7744-t8540-t8593+t9003+t10285+t10292-t11218-t11933+t12219+t12221+t14924+t15122+t15777+t15779+t15794+t15796+(t6276.*(t1918+t9.*(t71-t391)))./4.0+(t8622.*(t395+t9.*(t48-t349)))./4.0+(t7949.*(t3418-t3879+t4324+t11855+t9.*(t71-t391).*4.5305948634e-2+t17.*(t426-t581).*7.35522e-1+t9.*(t9166-t11658).*7.35522e-1))./4.0+(t1907.*(t1912.*(-1.0027e-2)+t2709+t3492+t751.*(t71-t391)))./4.0+(t7940.*(t3423+t3845+t3888+t3925+t4339+t9.*(t210+t2107+t7423+t9121).*7.35522e-1+t17.*(t9166-t11658).*7.35522e-1))./4.0+(t9362.*(t2091+t2497+t2579+t2680+t3516+t9.*(t210+t2107+t7423+t9121)+t17.*(t9166-t11658)))./4.0+(t9361.*(t1987-t2621+t3452+t11654+t9.*(t71-t391).*6.1597e-2+t17.*(t426-t581)+t9.*(t9166-t11658)))./4.0);
t16283 = t4484+t4576+t4580+t4749+t4773+t4786+t5002+t5030+t6965+t7270+t7384+t7472+t7744+t7785+t8540+t8593+t9007+t9038+t10285+t10292+t11218+t11933+t12219+t12221+t14925+t15123+t15778+t15780+t15783+t15784+t15795+t15797+t15802+t15803;
t9893 = -t9882;
t10130 = -t10124;
t10206 = -t10185;
t10393 = -t10378;
t10395 = -t10384;
t10407 = -t10403;
t10410 = t10187.*7.35522e-1;
t10423 = t10185.*7.35522e-1;
t10515 = (t3738.*t9926)./4.0;
t10518 = -t10511;
t10589 = -t10578;
t10592 = t9.*t10149.*1.13264871585e-2;
t10598 = -t10587;
t10610 = -t10600;
t10618 = t10187.*3.867742437e-3;
t10619 = -t10609;
t10625 = t10185.*1.563719772e-3;
t10715 = -t10707;
t10822 = -t10817;
t10826 = -t10823;
t10837 = -t10833;
t10853 = (t4300.*t10149)./4.0;
t10977 = -t10965;
t10989 = -t10962;
t11004 = (t5329.*t9926)./4.0;
t11014 = -t11007;
t11017 = -t11012;
t11024 = -t11019;
t11047 = -t11043;
t11050 = -t11048;
t11066 = -t11062;
t11096 = -t11094;
t11102 = -t11097;
t11108 = -t11101;
t11111 = -t11103;
t11142 = -t11136;
t11156 = t10962.*7.35522e-1;
t11157 = t10963.*7.35522e-1;
t11181 = -t11177;
t11217 = -t11216;
t11226 = -t11220;
t11230 = -t11222;
t11234 = -t11225;
t11238 = -t11229;
t11280 = (t5448.*t10149)./4.0;
t11300 = -t11291;
t11363 = -t11354;
t11371 = -t11361;
t11385 = t10963.*3.867742437e-3;
t11395 = t10962.*1.563719772e-3;
t11425 = -t11417;
t11426 = -t11419;
t11467 = -t11464;
t11475 = t3460+t3879+t10447;
t11489 = -t11485;
t11533 = -t11528;
t11542 = -t11535;
t11559 = t8.*t11356.*2.62925e-3;
t11576 = -t11563;
t11605 = -t11599;
t11643 = (t6408.*t10149)./4.0;
t11666 = (t6811.*t9926)./4.0;
t11693 = -t11688;
t11695 = t9.*t11470.*1.539925e-2;
t11697 = -t11690;
t11705 = -t11698;
t11726 = -t11718;
t11734 = -t11724;
t11737 = -t11728;
t11742 = -t11736;
t11768 = -t11756;
t11777 = -t11769;
t11819 = -t11817;
t11823 = (t2054.*t11470)./4.0;
t11853 = -t11844;
t11876 = (t6781.*t10149)./4.0;
t11891 = -t11889;
t11917 = -t11910;
t11930 = -t11928;
t11932 = (t4024.*t11356)./4.0;
t11946 = -t11942;
t11949 = -t11944;
t11992 = (t3767.*t11470)./4.0;
t11994 = -t11989;
t12010 = -t12003;
t12047 = -t12044;
t12056 = -t12055;
t12058 = -t12057;
t12081 = (t7540.*t10149)./4.0;
t12082 = -t12078;
t12096 = (t4517.*t11470)./4.0;
t12115 = (t4772.*t11470)./4.0;
t12131 = -t12126;
t12149 = (t7856.*t10149)./4.0;
t12164 = -t12158;
t12166 = (t7901.*t10149)./4.0;
t12190 = -t12184;
t12282 = (t5217.*t11470)./4.0;
t12283 = t8160+t10172;
t12304 = -t12298;
t12332 = t9.*t12307;
t12333 = t17.*t12307;
t12370 = -t12365;
t12381 = (t8464.*t10149)./4.0;
t12424 = (t5719.*t11470)./4.0;
t12429 = -t12427;
t12431 = (t8979.*t9926)./4.0;
t12440 = (t5760.*t11470)./4.0;
t12478 = (t6038.*t11470)./4.0;
t12484 = t8532+t10382;
t12487 = t8538+t10386;
t12494 = t17.*t12279.*3.867742437e-3;
t12495 = t9.*t12279.*1.563719772e-3;
t12496 = t16.*t12279.*4.38178973375e-3;
t12506 = t8560+t10424;
t12508 = t8566+t10427;
t12515 = -t12511;
t12518 = -t12513;
t12519 = -t12514;
t12522 = t8.*t12307.*4.38178973375e-3;
t12570 = (t6526.*t11470)./4.0;
t12571 = (t9049.*t10149)./4.0;
t12572 = (t9050.*t10149)./4.0;
t12595 = t8.*(t10384+t16.*(t4542-t6448).*1.666555).*(-2.62925e-3);
t12598 = t8.*(t10384+t16.*(t4542-t6448).*1.666555).*2.62925e-3;
t12607 = t16.*t12503.*2.62925e-3;
t12619 = -t12617;
t12620 = t9.*t12520.*1.539925e-2;
t12626 = -t12623;
t12633 = (t7116.*t11356)./4.0;
t12652 = -t12650;
t12653 = t9.*t3738.*t12279.*1.838805e-1;
t12656 = t17.*t3743.*t12279.*1.838805e-1;
t12699 = t2520.*(t10384+t16.*(t4542-t6448).*1.666555).*(-1.0./4.0);
t12707 = -t12698;
t12708 = (t2520.*(t10384+t16.*(t4542-t6448).*1.666555))./4.0;
t12710 = -t12702;
t12720 = (t2501.*t12503)./4.0;
t12748 = (t9362.*t10149)./4.0;
t12750 = (t4896.*t12279)./4.0;
t12762 = (t4938.*t12279)./4.0;
t12765 = (t12279.*(t2889-t2921))./4.0;
t12766 = (t12279.*(t2904-t2927))./4.0;
t12784 = t3421.*(t10378+t16.*(t4542-t6448).*7.35522e-1).*(-1.0./4.0);
t12788 = -t12781;
t12789 = (t3421.*(t10378+t16.*(t4542-t6448).*7.35522e-1))./4.0;
t12790 = t12500.*(t701-t775).*(-1.0./4.0);
t12791 = -t12786;
t12793 = -t12787;
t12794 = (t12307.*(t2904-t2927))./4.0;
t12795 = (t5069.*t12279)./4.0;
t12798 = (t3365.*t12500)./4.0;
t12800 = (t3455.*t12500)./4.0;
t12801 = (t3421.*t12500)./4.0;
t12808 = (t3489.*t12500)./4.0;
t12812 = (t9538.*t10149)./4.0;
t12814 = t3780.*(t10384+t16.*(t4542-t6448).*1.666555).*(-1.0./4.0);
t12815 = (t7348.*t11470)./4.0;
t12820 = -t12816;
t12825 = (t3732.*t12503)./4.0;
t12829 = (t5083.*t12307)./4.0;
t12851 = (t3738.*t12520)./4.0;
t12854 = t4021.*(t10384+t16.*(t4542-t6448).*1.666555).*(-1.0./4.0);
t12856 = t4024.*(t10384+t16.*(t4542-t6448).*1.666555).*(-1.0./4.0);
t12863 = (t4021.*(t10384+t16.*(t4542-t6448).*1.666555))./4.0;
t12864 = (t4024.*(t10384+t16.*(t4542-t6448).*1.666555))./4.0;
t12873 = (t4021.*t12503)./4.0;
t12874 = (t4024.*t12503)./4.0;
t12888 = (t5365.*t12279)./4.0;
t12892 = (t4152.*t12500)./4.0;
t12903 = (t5430.*t12279)./4.0;
t12907 = (t9.*t5434.*t12279)./4.0;
t12908 = (t17.*t5433.*t12279)./4.0;
t12925 = t4509.*(t10384+t16.*(t4542-t6448).*1.666555).*(-1.0./4.0);
t12927 = t4514.*(t10384+t16.*(t4542-t6448).*1.666555).*(-1.0./4.0);
t12930 = (t4509.*(t10384+t16.*(t4542-t6448).*1.666555))./4.0;
t12932 = (t5441.*t12307)./4.0;
t12933 = (t4514.*(t10384+t16.*(t4542-t6448).*1.666555))./4.0;
t12935 = -t12928;
t12936 = -t12929;
t12938 = (t11470.*(t2056+t2203+t2351+t3433+t3503+t16.*t389.*(1.1e+1./1.25e+2)))./4.0;
t12941 = (t4489.*t12503)./4.0;
t12944 = (t4498.*t12503)./4.0;
t12945 = t8555+t11129;
t12953 = t8569+t11130;
t12956 = -t12950;
t12958 = -t12952;
t12969 = t9.*t12689.*1.13264871585e-2;
t12975 = t17.*t12705.*1.13264871585e-2;
t12979 = t11356.*(-t1476-t1540+t2091+t2165+t2579+t8.*(t260+t468+t570+t2298)).*(-1.0./4.0);
t12984 = (t7940.*t11470)./4.0;
t12990 = (t9887.*t10149)./4.0;
t12995 = (t7982.*t11470)./4.0;
t12997 = t9.*t5329.*t12279.*1.838805e-1;
t13004 = t17.*t5345.*t12279.*1.838805e-1;
t13028 = -t13021;
t13033 = (t9922.*t10149)./2.0;
t13034 = -t13030;
t13040 = t9926.*(t1987-t2621+t3452-t4730+t5359+t9.*(t71-t391).*6.1597e-2+t17.*(t426-t581)).*(-1.0./2.0);
t13042 = (t9926.*(t1987-t2621+t3452-t4730+t5359+t9.*(t71-t391).*6.1597e-2+t17.*(t426-t581)))./2.0;
t13043 = (t5914.*t12279)./4.0;
t13044 = (t5919.*t12279)./4.0;
t13045 = (t4964.*t12500)./4.0;
t13049 = t5050.*(t10384+t16.*(t4542-t6448).*1.666555).*(-1.0./4.0);
t13053 = (t5007.*t12503)./4.0;
t13057 = (t6046.*t12279)./4.0;
t13059 = -t13056;
t13062 = (t5912.*t12307)./4.0;
t13063 = (t6069.*t12279)./4.0;
t13064 = (t5915.*t12307)./4.0;
t13075 = (t6104.*t12279)./4.0;
t13087 = t5234.*(t10384+t16.*(t4542-t6448).*1.666555).*(-1.0./4.0);
t13089 = t5235.*(t10384+t16.*(t4542-t6448).*1.666555).*(-1.0./4.0);
t13091 = -t13084;
t13093 = (t5235.*(t10384+t16.*(t4542-t6448).*1.666555))./4.0;
t13094 = (t6046.*t12307)./4.0;
t13095 = -t13092;
t13099 = (t6069.*t12307)./4.0;
t13103 = -t13101;
t13104 = (t5234.*t12503)./4.0;
t13106 = (t5235.*t12503)./4.0;
t13128 = (t6304.*t12279)./4.0;
t13130 = (t5290.*t12500)./4.0;
t13132 = t9.*t12987.*1.539925e-2;
t13148 = -t13145;
t13152 = (t5329.*t12520)./4.0;
t13167 = t10159+t10187;
t13174 = (t5524.*t12500)./4.0;
t13175 = t9245+t10963;
t13176 = (t5552.*t12500)./4.0;
t13185 = t5696.*(t10378+t16.*(t4542-t6448).*7.35522e-1).*(-1.0./4.0);
t13188 = (t5696.*(t10378+t16.*(t4542-t6448).*7.35522e-1))./4.0;
t13192 = (t5696.*t12500)./4.0;
t13200 = (t6681.*t12279)./4.0;
t13204 = (t8725.*t11470)./2.0;
t13217 = -t13214;
t13224 = t5923.*(t10384+t16.*(t4542-t6448).*1.666555).*(-1.0./4.0);
t13227 = (t6677.*t12307)./4.0;
t13229 = (t5923.*(t10384+t16.*(t4542-t6448).*1.666555))./4.0;
t13233 = t5952.*(t10384+t16.*(t4542-t6448).*1.666555).*(-1.0./4.0);
t13235 = (t5952.*(t10384+t16.*(t4542-t6448).*1.666555))./4.0;
t13239 = (t6884.*t12279)./4.0;
t13240 = t6014.*(t10384+t16.*(t4542-t6448).*1.666555).*(-1.0./4.0);
t13241 = (t6872.*t12279)./4.0;
t13245 = (t5929.*t12503)./4.0;
t13250 = (t5947.*t12503)./4.0;
t13253 = (t5951.*t12503)./4.0;
t13266 = (t6966.*t12279)./4.0;
t13269 = t10149.*(t4324-t5228+t5802+t9.*(t71-t391).*4.5305948634e-2+t17.*(t426-t581).*7.35522e-1).*(-1.0./2.0);
t13276 = (t10149.*(t4324-t5228+t5802+t9.*(t71-t391).*4.5305948634e-2+t17.*(t426-t581).*7.35522e-1))./2.0;
t13277 = -t13270;
t13279 = -t13274;
t13280 = (t6884.*t12307)./4.0;
t13282 = (t6872.*t12307)./4.0;
t13287 = (t3738.*t12987)./4.0;
t13289 = (t6096.*t12500)./4.0;
t13298 = (t10149.*t10485)./4.0;
t13300 = (t9001.*t11470)./4.0;
t13301 = (t6158.*t12500)./4.0;
t13302 = t10149.*(-t3823+t3970+t5243+t9.*(t260+t468+t570+t2298).*7.35522e-1+t972.*(t71-t391)+t2777.*(t71-t391)).*(-1.0./2.0);
t13310 = t6302.*(t10378+t16.*(t4542-t6448).*7.35522e-1).*(-1.0./4.0);
t13312 = t12500.*(-t2149+t2205+t693.*(t48-t349)+t784.*(t48-t349)).*(-1.0./4.0);
t13315 = (t12500.*(-t2149+t2205+t693.*(t48-t349)+t784.*(t48-t349)))./4.0;
t13316 = (t6302.*t12500)./4.0;
t13321 = -t13317;
t13322 = (t7215.*t12279)./4.0;
t13323 = -t13320;
t13324 = (t5434.*t12689)./4.0;
t13327 = t17.*t6761.*t12279.*1.838805e-1;
t13331 = (t5433.*t12705)./4.0;
t13336 = t9.*t6811.*t12279.*1.838805e-1;
t13350 = -t13345;
t13354 = t12500.*(t624+t2511-t3502-t9.*t439.*4.252e-3).*(-1.0./4.0);
t13356 = -t13352;
t13361 = (t12500.*(t624+t2511-t3502-t9.*t439.*4.252e-3))./4.0;
t13369 = -t13366;
t13386 = t9556+t11179;
t13398 = -t13395;
t13400 = t9.*t13181.*1.13264871585e-2;
t13404 = -t13402;
t13409 = t11470.*(-t2550+t2696+t2698+t4771+t9.*(t260+t468+t570+t2298)+t147.*(t71-t391)).*(-1.0./2.0);
t13417 = (t10149.*t10763)./2.0;
t13419 = (t9197.*t11470)./2.0;
t13422 = (t7612.*t12279)./4.0;
t13424 = (t7622.*t12279)./4.0;
t13429 = (t9233.*t11470)./2.0;
t13430 = (t10149.*t10783)./2.0;
t13432 = t6744.*(t10384+t16.*(t4542-t6448).*1.666555).*(-1.0./4.0);
t13442 = (t6729.*t12503)./4.0;
t13443 = -t13438;
t13447 = (t7613.*t12307)./4.0;
t13452 = (t7646.*t12307)./4.0;
t13460 = t11470.*(t3452-t4730+t5359+t9.*(t71-t391).*6.1597e-2+t17.*(t426-t581)).*(-1.0./2.0);
t13466 = (t11470.*(t3452-t4730+t5359+t9.*(t71-t391).*6.1597e-2+t17.*(t426-t581)))./2.0;
t13467 = t6957.*(t10384+t16.*(t4542-t6448).*1.666555).*(-1.0./4.0);
t13468 = (t9.*t7796.*t12279)./4.0;
t13469 = (t17.*t7797.*t12279)./4.0;
t13472 = (t6957.*(t10384+t16.*(t4542-t6448).*1.666555))./4.0;
t13483 = -t13479;
t13485 = t12503.*(-t1540+t2091+t2579+t8.*(t260+t468+t570+t2298)).*(-1.0./4.0);
t13486 = t12279.*(t3479-t3544+t2772.*(t48-t349)+t2775.*(t48-t349)).*(-1.0./4.0);
t13488 = ((t10384+t16.*(t4542-t6448).*1.666555).*(t1492+t2158+t2696-t4727))./4.0;
t13489 = (t6811.*t12520)./4.0;
t13490 = -t13484;
t13491 = (t12503.*(-t1540+t2091+t2579+t8.*(t260+t468+t570+t2298)))./4.0;
t13492 = (t12279.*(t3479-t3544+t2772.*(t48-t349)+t2775.*(t48-t349)))./4.0;
t13501 = -t13495;
t13502 = -t13497;
t13505 = (t6995.*t12503)./4.0;
t13510 = t17.*t13382.*1.539925e-2;
t13514 = t7079.*(t10384+t16.*(t4542-t6448).*1.666555).*(-1.0./4.0);
t13520 = t17.*t13387.*1.539925e-2;
t13521 = (t7079.*(t10384+t16.*(t4542-t6448).*1.666555))./4.0;
t13528 = t7105.*(t10384+t16.*(t4542-t6448).*1.666555).*(-1.0./4.0);
t13533 = t9.*t13391.*1.539925e-2;
t13537 = t7116.*(t10384+t16.*(t4542-t6448).*1.666555).*(-1.0./4.0);
t13538 = (t7980.*t12279)./4.0;
t13540 = (t7066.*t12503)./4.0;
t13542 = (t7116.*(t10384+t16.*(t4542-t6448).*1.666555))./4.0;
t13544 = (t7079.*t12503)./4.0;
t13549 = (t7116.*t12503)./4.0;
t13551 = (t7128.*t12500)./4.0;
t13552 = (t7130.*t12500)./4.0;
t13558 = (t8070.*t12279)./4.0;
t13559 = t12279.*(t2752+t3814-t4385-t9.*t439.*3.127439544e-3).*(-1.0./4.0);
t13562 = (t12279.*(t2752+t3814-t4385-t9.*t439.*3.127439544e-3))./4.0;
t13568 = -t13564;
t13573 = -t13570;
t13580 = -t13575;
t13583 = (t8062.*t12307)./4.0;
t13602 = (t7336.*t12500)./4.0;
t13609 = t7434.*(t10384+t16.*(t4542-t6448).*1.666555).*(-1.0./4.0);
t13611 = (t7434.*(t10384+t16.*(t4542-t6448).*1.666555))./4.0;
t13612 = (t7402.*t12503)./4.0;
t13642 = (t8477.*t12279)./4.0;
t13644 = (t8497.*t12279)./4.0;
t13653 = (t8547.*t12279)./4.0;
t13655 = -t13652;
t13656 = t12279.*(-t3218+t3458+t3878+t8.*(t260+t468+t570+t2298).*1.666555).*(-1.0./4.0);
t13659 = (t8477.*t12307)./4.0;
t13660 = (t12279.*(-t3218+t3458+t3878+t8.*(t260+t468+t570+t2298).*1.666555))./4.0;
t13661 = -t13658;
t13662 = (t7654.*t12500)./4.0;
t13667 = (t8600.*t12279)./4.0;
t13677 = (t3743.*t13382)./4.0;
t13690 = (t8562.*t12307)./4.0;
t13691 = (t8640.*t12279)./4.0;
t13697 = -t13693;
t13699 = (t8654.*t12279)./4.0;
t13704 = t12307.*(t3063+t3528+t3966-t5230).*(-1.0./4.0);
t13707 = -t13705;
t13710 = -t13708;
t13713 = (t8640.*t12307)./4.0;
t13725 = -t13721;
t13727 = (t8709.*t12279)./4.0;
t13736 = -t13731;
t13741 = -t13737;
t13756 = (t8713.*t12307)./4.0;
t13762 = (t8063.*t12500)./4.0;
t13768 = -t13763;
t13777 = (t5434.*t13181)./4.0;
t13788 = t8191.*(t10378+t16.*(t4542-t6448).*7.35522e-1).*(-1.0./4.0);
t13796 = (t8191.*(t10378+t16.*(t4542-t6448).*7.35522e-1))./4.0;
t13797 = t8227.*(t10384+t16.*(t4542-t6448).*1.666555).*(-1.0./4.0);
t13802 = (t8227.*(t10384+t16.*(t4542-t6448).*1.666555))./4.0;
t13804 = ((t10384+t16.*(t4542-t6448).*1.666555).*(-t1476-t1540+t2091+t2165+t2579+t8.*(t260+t468+t570+t2298)))./4.0;
t13807 = t8253.*(t10384+t16.*(t4542-t6448).*1.666555).*(-1.0./4.0);
t13814 = (t8178.*t12503)./4.0;
t13815 = (t8191.*t12500)./4.0;
t13821 = (t8227.*t12503)./4.0;
t13827 = t12503.*(-t1476-t1540+t2091+t2165+t2579+t8.*(t260+t468+t570+t2298)).*(-1.0./4.0);
t13831 = (t12503.*(-t1476-t1540+t2091+t2165+t2579+t8.*(t260+t468+t570+t2298)))./4.0;
t13844 = -t13843;
t13854 = (t9028.*t12279)./4.0;
t13858 = (t10149.*t11484)./2.0;
t13861 = (t8433.*t12500)./4.0;
t13864 = -t13859;
t13865 = (t10180.*t11470)./2.0;
t13872 = -t13870;
t13889 = (t9098.*t12279)./4.0;
t13892 = (t9110.*t12279)./4.0;
t13893 = (t9112.*t12279)./4.0;
t13900 = (t6811.*t12987)./4.0;
t13907 = t9.*t8979.*t12279.*1.838805e-1;
t13908 = -t13902;
t13910 = t17.*t8981.*t12279.*1.838805e-1;
t13914 = (t8628.*t12500)./4.0;
t13919 = -t13916;
t13920 = -t13917;
t13921 = (t9106.*t12307)./4.0;
t13922 = (t9110.*t12307)./4.0;
t13923 = (t9112.*t12307)./4.0;
t13937 = -t13929;
t13938 = -t13932;
t13951 = (t5345.*t13382)./4.0;
t13952 = (t17.*t9185.*t12279)./4.0;
t13958 = (t8693.*t12500)./4.0;
t13961 = (t9.*t9194.*t12279)./4.0;
t13962 = (t5329.*t13391)./4.0;
t13965 = (t5345.*t13387)./4.0;
t13976 = -t13972;
t13984 = (t12279.*(t3098+t3199+t3211-t3221+t3678+t4612))./4.0;
t13989 = -t13985;
t13991 = -t13987;
t13995 = (t9310.*t12279)./4.0;
t14000 = (t9269.*t12307)./4.0;
t14003 = -t14002;
t14014 = (t9505.*t12279)./4.0;
t14041 = (t9717.*t12279)./4.0;
t14043 = (t9744.*t12279)./4.0;
t14045 = t12279.*(-t3045-t3218+t3458+t3539+t3878+t8.*(t260+t468+t570+t2298).*1.666555).*(-1.0./4.0);
t14047 = (t12279.*(-t3045-t3218+t3458+t3539+t3878+t8.*(t260+t468+t570+t2298).*1.666555))./4.0;
t14052 = (t9196.*t12500)./4.0;
t14053 = -t14046;
t14056 = -t14054;
t14064 = -t14061;
t14065 = ((t10378+t16.*(t4542-t6448).*7.35522e-1).*(t249-t391.*(1.1e+1./1.25e+2)-t1912.*4.252e-3+t3505+t5357+t693.*(t71-t391)+t784.*(t71-t391)))./4.0;
t14071 = -t14066;
t14075 = (t9743.*t12307)./4.0;
t14076 = (t9744.*t12307)./4.0;
t14079 = t12307.*(-t3045-t3218+t3458+t3539+t3878+t8.*(t260+t468+t570+t2298).*1.666555).*(-1.0./4.0);
t14086 = (t12307.*(-t3045-t3218+t3458+t3539+t3878+t8.*(t260+t468+t570+t2298).*1.666555))./4.0;
t14090 = t12500.*(t249-t391.*(1.1e+1./1.25e+2)-t1912.*4.252e-3+t3505+t5357+t693.*(t71-t391)+t784.*(t71-t391)).*(-1.0./4.0);
t14091 = (t12500.*(t249-t391.*(1.1e+1./1.25e+2)-t1912.*4.252e-3+t3505+t5357+t693.*(t71-t391)+t784.*(t71-t391)))./4.0;
t14117 = (t6761.*t13387)./4.0;
t14127 = (t6811.*t13391)./4.0;
t14138 = -t14135;
t14140 = (t10096.*t12279)./4.0;
t14141 = (t7796.*t13181)./4.0;
t14142 = -t14139;
t14143 = (t10111.*t12279)./4.0;
t14147 = -t14145;
t14163 = (t10141.*t12279)./4.0;
t14168 = -t14166;
t14176 = (t9194.*t12689)./4.0;
t14177 = (t9185.*t12705)./4.0;
t14181 = -t14179;
t14183 = (t10141.*t12307)./4.0;
t14185 = t10173+t12292;
t14186 = t10193+t12291;
t14196 = -t14192;
t14198 = -t14194;
t14201 = -t14199;
t14203 = (t10240.*t12279)./4.0;
t14204 = -t14200;
t14206 = -t14202;
t14216 = -t14215;
t14224 = -t14222;
t14228 = -t14226;
t14229 = (t8979.*t12987)./4.0;
t14233 = t17.*t10149.*t12279.*1.838805e-1;
t14235 = t9.*t12279.*(t1987-t2621+t3452-t4730+t5359+t9.*(t71-t391).*6.1597e-2+t17.*(t426-t581)).*(-1.838805e-1);
t14240 = t9.*t12279.*(t1987-t2621+t3452-t4730+t5359+t9.*(t71-t391).*6.1597e-2+t17.*(t426-t581)).*1.838805e-1;
t14241 = (t10398.*t12279)./4.0;
t14242 = t17.*t10149.*t12296.*1.838805e-1;
t14249 = (t9.*t10468.*t12279)./4.0;
t14250 = (t17.*t10469.*t12279)./4.0;
t14258 = -t14256;
t14259 = -t14257;
t14265 = -t14263;
t14280 = t10402+t12415;
t14293 = t10149.*(t8610-t10439).*(-1.0./4.0);
t14294 = t12520.*(t1987-t2621+t3452-t4730+t5359+t9.*(t71-t391).*6.1597e-2+t17.*(t426-t581)).*(-1.0./4.0);
t14295 = (t10149.*(t8610-t10439))./4.0;
t14310 = (t10149.*t12563)./4.0;
t14317 = -t14313;
t14318 = -t14316;
t14322 = -t14319;
t14325 = -t14321;
t14326 = -t14323;
t14346 = t9.*(t10403+t9.*(t10158+t16.*(t4542-t6448)).*7.35522e-1).*(-1.539925e-2);
t14352 = (t10863.*t12279)./4.0;
t14367 = t12279.*(t1589-t2213+t3195-t4346+t4355+t4748.*7.35522e-1+t2772.*(t71-t391)+t2775.*(t71-t391)).*(-1.0./4.0);
t14372 = t2044.*(t10403+t9.*(t10158+t16.*(t4542-t6448)).*7.35522e-1).*(-1.0./4.0);
t14375 = -t14371;
t14376 = (t2044.*(t10403+t9.*(t10158+t16.*(t4542-t6448)).*7.35522e-1))./4.0;
t14377 = -t14374;
t14390 = t12307.*(t1589-t2213+t3195-t4346+t4355+t4748.*7.35522e-1+t2772.*(t71-t391)+t2775.*(t71-t391)).*(-1.0./4.0);
t14393 = (t12307.*(t1589-t2213+t3195-t4346+t4355+t4748.*7.35522e-1+t2772.*(t71-t391)+t2775.*(t71-t391)))./4.0;
t14396 = -t14392;
t14407 = -t14403;
t14409 = -t14406;
t14413 = t3367+t3819+t3875+t4361+t13621;
t14423 = (t8981.*t13382)./4.0;
t14428 = (t8981.*t13387)./4.0;
t14430 = (t8979.*t13391)./4.0;
t14432 = -t14429;
t14435 = -t14433;
t14440 = -t14436;
t14448 = t3738.*(t10403+t9.*(t10158+t16.*(t4542-t6448)).*7.35522e-1).*(-1.0./4.0);
t14450 = t3743.*(t10403+t9.*(t10158+t16.*(t4542-t6448)).*7.35522e-1).*(-1.0./4.0);
t14453 = (t3738.*(t10403+t9.*(t10158+t16.*(t4542-t6448)).*7.35522e-1))./4.0;
t14454 = t3763.*(t10403+t9.*(t10158+t16.*(t4542-t6448)).*7.35522e-1).*(-1.0./4.0);
t14455 = (t3743.*(t10403+t9.*(t10158+t16.*(t4542-t6448)).*7.35522e-1))./4.0;
t14458 = (t3763.*(t10403+t9.*(t10158+t16.*(t4542-t6448)).*7.35522e-1))./4.0;
t14460 = t8.*t14380.*2.62925e-3;
t14473 = (t10468.*t12689)./4.0;
t14479 = -t14476;
t14480 = (t10469.*t12705)./4.0;
t14481 = (t5434.*t14161)./4.0;
t14487 = -t14486;
t14504 = (t2501.*t14380)./4.0;
t14505 = t4474.*(t10403+t9.*(t10158+t16.*(t4542-t6448)).*7.35522e-1).*(-1.0./4.0);
t14509 = (t4474.*(t10403+t9.*(t10158+t16.*(t4542-t6448)).*7.35522e-1))./4.0;
t14531 = t10149.*(t8583-t11188).*(-1.0./4.0);
t14535 = t12987.*(t1987-t2621+t3452-t4730+t5359+t9.*(t71-t391).*6.1597e-2+t17.*(t426-t581)).*(-1.0./4.0);
t14537 = (t10149.*(t8583-t11188))./4.0;
t14539 = t4798.*(t10403+t9.*(t10158+t16.*(t4542-t6448)).*7.35522e-1).*(-1.0./4.0);
t14540 = (t4798.*(t10403+t9.*(t10158+t16.*(t4542-t6448)).*7.35522e-1))./4.0;
t14560 = t9.*t12279.*(t3418-t3879+t4324-t5228+t5802+t9.*(t71-t391).*4.5305948634e-2+t17.*(t426-t581).*7.35522e-1).*(-1.0./4.0);
t14562 = -t14559;
t14563 = (t17.*t11470.*t12279)./4.0;
t14564 = (t9.*t12279.*(t3418-t3879+t4324-t5228+t5802+t9.*(t71-t391).*4.5305948634e-2+t17.*(t426-t581).*7.35522e-1))./4.0;
t14569 = (t3732.*t14380)./4.0;
t14576 = (t17.*t11470.*t12296)./4.0;
t14582 = t11470.*(t8266-t10204).*(-1.0./4.0);
t14583 = (t11470.*(t8266-t10204))./4.0;
t14585 = t5213.*(t10403+t9.*(t10158+t16.*(t4542-t6448)).*7.35522e-1).*(-1.0./4.0);
t14588 = (t3743.*t14411)./4.0;
t14603 = t5329.*(t10403+t9.*(t10158+t16.*(t4542-t6448)).*7.35522e-1).*(-1.0./4.0);
t14607 = (t5329.*(t10403+t9.*(t10158+t16.*(t4542-t6448)).*7.35522e-1))./4.0;
t14609 = t5345.*(t10403+t9.*(t10158+t16.*(t4542-t6448)).*7.35522e-1).*(-1.0./4.0);
t14613 = t11470.*(t8329+t17.*(t16.*(t30.*(t2425-t2468)+t68.*(t2425-t2468))+t8.*(t7.*(t4650+t34.*(t2425-t2468))+t47.*(t2425-t2468)))).*(-1.0./4.0);
t14619 = (t4489.*t14380)./4.0;
t14623 = (t4498.*t14380)./4.0;
t14645 = t5679.*(t10403+t9.*(t10158+t16.*(t4542-t6448)).*7.35522e-1).*(-1.0./4.0);
t14648 = (t5679.*(t10403+t9.*(t10158+t16.*(t4542-t6448)).*7.35522e-1))./4.0;
t14655 = t5782.*(t10403+t9.*(t10158+t16.*(t4542-t6448)).*7.35522e-1).*(-1.0./4.0);
t14659 = (t5782.*(t10403+t9.*(t10158+t16.*(t4542-t6448)).*7.35522e-1))./4.0;
t14661 = (t5007.*t14380)./4.0;
t14674 = -t14672;
t14676 = -t14673;
t14689 = t6016.*(t10403+t9.*(t10158+t16.*(t4542-t6448)).*7.35522e-1).*(-1.0./4.0);
t14691 = (t6016.*(t10403+t9.*(t10158+t16.*(t4542-t6448)).*7.35522e-1))./4.0;
t14716 = -t14714;
t14718 = (t10468.*t13181)./4.0;
t14719 = -t14717;
t14723 = -t14721;
t14731 = (t5345.*t14411)./4.0;
t14733 = (t10149.*t13382)./4.0;
t14736 = (t10149.*t13387)./4.0;
t14740 = t13391.*(t1987-t2621+t3452-t4730+t5359+t9.*(t71-t391).*6.1597e-2+t17.*(t426-t581)).*(-1.0./4.0);
t14741 = t6540.*(t10403+t9.*(t10158+t16.*(t4542-t6448)).*7.35522e-1).*(-1.0./4.0);
t14757 = t10960+t13036;
t14761 = (t5929.*t14380)./4.0;
t14762 = (t5951.*t14380)./4.0;
t14765 = (t5947.*t14380)./4.0;
t14766 = t12689.*(t3418-t3879+t4324-t5228+t5802+t9.*(t71-t391).*4.5305948634e-2+t17.*(t426-t581).*7.35522e-1).*(-1.0./4.0);
t14769 = (t7796.*t14161)./4.0;
t14771 = (t11470.*t12705)./4.0;
t14777 = t6761.*(t10403+t9.*(t10158+t16.*(t4542-t6448)).*7.35522e-1).*(-1.0./4.0);
t14779 = (t6761.*(t10403+t9.*(t10158+t16.*(t4542-t6448)).*7.35522e-1))./4.0;
t14788 = t6811.*(t10403+t9.*(t10158+t16.*(t4542-t6448)).*7.35522e-1).*(-1.0./4.0);
t14791 = (t6811.*(t10403+t9.*(t10158+t16.*(t4542-t6448)).*7.35522e-1))./4.0;
t14802 = t11470.*(t8221-t11008).*(-1.0./4.0);
t14807 = (t11470.*(t8221-t11008))./4.0;
t14812 = -t14806;
t14863 = ((t10403+t9.*(t10158+t16.*(t4542-t6448)).*7.35522e-1).*(t1468-t1988-t2498+t4565+t17.*(t208-t427)))./4.0;
t14878 = (t6729.*t14380)./4.0;
t14879 = t11164+t13146;
t14883 = t17.*t14752.*1.13264871585e-2;
t14893 = t14380.*(-t1540+t2091+t2579+t8.*(t260+t468+t570+t2298)).*(-1.0./4.0);
t14897 = (t14380.*(-t1540+t2091+t2579+t8.*(t260+t468+t570+t2298)))./4.0;
t14903 = (t6995.*t14380)./4.0;
t14915 = t7799.*(t10403+t9.*(t10158+t16.*(t4542-t6448)).*7.35522e-1).*(-1.0./4.0);
t14917 = (t7066.*t14380)./4.0;
t14921 = (t6761.*t14411)./4.0;
t14938 = t7949.*(t10403+t9.*(t10158+t16.*(t4542-t6448)).*7.35522e-1).*(-1.0./4.0);
t14939 = (t7949.*(t10403+t9.*(t10158+t16.*(t4542-t6448)).*7.35522e-1))./4.0;
t14944 = t7987.*(t10403+t9.*(t10158+t16.*(t4542-t6448)).*7.35522e-1).*(-1.0./4.0);
t14945 = (t7987.*(t10403+t9.*(t10158+t16.*(t4542-t6448)).*7.35522e-1))./4.0;
t14952 = t9.*(t13145+t17.*(t8963+t7.*(t5026+t5.*(t2959-t2967))).*7.35522e-1).*(-1.539925e-2);
t14955 = t9.*(t13145+t17.*(t8963+t7.*(t5026+t5.*(t2959-t2967))).*7.35522e-1).*1.539925e-2;
t14960 = (t7402.*t14380)./4.0;
t14973 = -t14972;
t14975 = -t14974;
t14981 = t12392.*(t10384+t16.*(t4542-t6448).*1.666555).*(-1.0./4.0);
t14983 = (t12392.*(t10384+t16.*(t4542-t6448).*1.666555))./4.0;
t14985 = t12503.*(t1292+t2073+t2694+t11671).*(-1.0./4.0);
t14987 = (t11470.*t13177)./4.0;
t14988 = (t12503.*(t1292+t2073+t2694+t11671))./4.0;
t14992 = (t11470.*t13182)./4.0;
t14994 = t13181.*(t3418-t3879+t4324-t5228+t5802+t9.*(t71-t391).*4.5305948634e-2+t17.*(t426-t581).*7.35522e-1).*(-1.0./4.0);
t15006 = -t15005;
t15019 = (t9194.*t14161)./4.0;
t15022 = t3738.*(t13145+t17.*(t8963+t7.*(t5026+t5.*(t2959-t2967))).*7.35522e-1).*(-1.0./4.0);
t15025 = (t3738.*(t13145+t17.*(t8963+t7.*(t5026+t5.*(t2959-t2967))).*7.35522e-1))./4.0;
t15039 = (t8178.*t14380)./4.0;
t15043 = t8743.*(t10403+t9.*(t10158+t16.*(t4542-t6448)).*7.35522e-1).*(-1.0./4.0);
t15048 = (t8743.*(t10403+t9.*(t10158+t16.*(t4542-t6448)).*7.35522e-1))./4.0;
t15067 = (t5433.*t14752)./4.0;
t15074 = t8979.*(t10403+t9.*(t10158+t16.*(t4542-t6448)).*7.35522e-1).*(-1.0./4.0);
t15077 = t8981.*(t10403+t9.*(t10158+t16.*(t4542-t6448)).*7.35522e-1).*(-1.0./4.0);
t15080 = (t8979.*(t10403+t9.*(t10158+t16.*(t4542-t6448)).*7.35522e-1))./4.0;
t15082 = (t8981.*(t10403+t9.*(t10158+t16.*(t4542-t6448)).*7.35522e-1))./4.0;
t15085 = t8999.*(t10403+t9.*(t10158+t16.*(t4542-t6448)).*7.35522e-1).*(-1.0./4.0);
t15086 = t12279.*(t3116+t3486+t3963+t11671.*1.666555).*(-1.0./4.0);
t15090 = (t12279.*(t3116+t3486+t3963+t11671.*1.666555))./4.0;
t15105 = (t12307.*t12792)./4.0;
t15133 = ((t10403+t9.*(t10158+t16.*(t4542-t6448)).*7.35522e-1).*(t824+t2543+t2699+t2707-t4767+t17.*(t260+t468+t570+t2298)))./4.0;
t15139 = t9187.*(t10403+t9.*(t10158+t16.*(t4542-t6448)).*7.35522e-1).*(-1.0./4.0);
t15145 = t12696.*(t10384+t16.*(t4542-t6448).*1.666555).*(-1.0./4.0);
t15146 = (t12503.*t12667)./4.0;
t15154 = t9252.*(t10403+t9.*(t10158+t16.*(t4542-t6448)).*7.35522e-1).*(-1.0./4.0);
t15158 = (t9252.*(t10403+t9.*(t10158+t16.*(t4542-t6448)).*7.35522e-1))./4.0;
t15161 = t5329.*(t13145+t17.*(t8963+t7.*(t5026+t5.*(t2959-t2967))).*7.35522e-1).*(-1.0./4.0);
t15163 = (t5329.*(t13145+t17.*(t8963+t7.*(t5026+t5.*(t2959-t2967))).*7.35522e-1))./4.0;
t15166 = t9292.*(t10403+t9.*(t10158+t16.*(t4542-t6448)).*7.35522e-1).*(-1.0./4.0);
t15170 = (t9292.*(t10403+t9.*(t10158+t16.*(t4542-t6448)).*7.35522e-1))./4.0;
t15191 = t9926.*(t10174+t9.*(t10158+t16.*(t4542-t6448))).*(-1.0./4.0);
t15192 = (t9926.*(t10174+t9.*(t10158+t16.*(t4542-t6448))))./4.0;
t15197 = (t8981.*t14411)./4.0;
t15200 = -t15198;
t15214 = t12867.*(t10384+t16.*(t4542-t6448).*1.666555).*(-1.0./4.0);
t15222 = (t12503.*t12860)./4.0;
t15224 = (t12500.*t12866)./4.0;
t15233 = (t12279.*t13196)./4.0;
t15235 = (t12279.*t13197)./4.0;
t15239 = t13013.*(t10384+t16.*(t4542-t6448).*1.666555).*(-1.0./4.0);
t15241 = -t15236;
t15244 = (t13013.*(t10384+t16.*(t4542-t6448).*1.666555))./4.0;
t15247 = (t12503.*t13005)./4.0;
t15249 = (t12500.*t13005)./4.0;
t15253 = -t15248;
t15255 = -t15250;
t15258 = t13038.*(t10384+t16.*(t4542-t6448).*1.666555).*(-1.0./4.0);
t15260 = (t12307.*t13198)./4.0;
t15261 = (t13038.*(t10384+t16.*(t4542-t6448).*1.666555))./4.0;
t15264 = (t12503.*t13019)./4.0;
t15268 = (t10468.*t14161)./4.0;
t15302 = (t12279.*t13326)./4.0;
t15307 = t6811.*(t13145+t17.*(t8963+t7.*(t5026+t5.*(t2959-t2967))).*7.35522e-1).*(-1.0./4.0);
t15309 = (t6811.*(t13145+t17.*(t8963+t7.*(t5026+t5.*(t2959-t2967))).*7.35522e-1))./4.0;
t15313 = (t12500.*t13150)./4.0;
t15314 = (t7797.*t14752)./4.0;
t15322 = -t15317;
t15329 = t10149.*(t10403+t9.*(t10158+t16.*(t4542-t6448)).*7.35522e-1).*(-1.0./4.0);
t15331 = ((t10403+t9.*(t10158+t16.*(t4542-t6448)).*7.35522e-1).*(t1987-t2621+t3452-t4730+t5359+t9.*(t71-t391).*6.1597e-2+t17.*(t426-t581)))./4.0;
t15334 = (t12307.*t13333)./4.0;
t15339 = (t12279.*t13376)./4.0;
t15342 = t10170.*(t10403+t9.*(t10158+t16.*(t4542-t6448)).*7.35522e-1).*(-1.0./4.0);
t15345 = (t10170.*(t10403+t9.*(t10158+t16.*(t4542-t6448)).*7.35522e-1))./4.0;
t15360 = -t15354;
t15363 = -t15357;
t15365 = (t12307.*t13380)./4.0;
t15394 = (t12500.*t13273)./4.0;
t15402 = (t12500.*t13313)./4.0;
t15403 = (t12279.*t13578)./4.0;
t15405 = (t16.*t10153.*t14380)./4.0;
t15411 = t16.*t14380.*(t6452-t8229).*(-1.0./4.0);
t15414 = (t10199.*t14380)./4.0;
t15416 = (t16.*t14380.*(t6452-t8229))./4.0;
t15418 = -t15415;
t15420 = (t11356.*(-t1476+t2165+t13876))./4.0;
t15425 = -t15424;
t15430 = t14380.*(t8315+t8.*(t30.*(t2425-t2468)+t68.*(t2425-t2468))).*(-1.0./4.0);
t15431 = (t14380.*(t8315+t8.*(t30.*(t2425-t2468)+t68.*(t2425-t2468))))./4.0;
t15432 = (t10149.*t14411)./4.0;
t15433 = (t12279.*(t3098+t3211-t3221+t3678+t8102+t10798))./4.0;
t15442 = (t12307.*t13627)./4.0;
t15452 = (t11470.*t14156)./4.0;
t15454 = (t9185.*t14752)./4.0;
t15455 = t14161.*(t3418-t3879+t4324-t5228+t5802+t9.*(t71-t391).*4.5305948634e-2+t17.*(t426-t581).*7.35522e-1).*(-1.0./4.0);
t15457 = (t14161.*(t3418-t3879+t4324-t5228+t5802+t9.*(t71-t391).*4.5305948634e-2+t17.*(t426-t581).*7.35522e-1))./4.0;
t15468 = t11470.*(t10174+t9.*(t10158+t16.*(t4542-t6448))).*(-1.0./4.0);
t15477 = t8979.*(t13145+t17.*(t8963+t7.*(t5026+t5.*(t2959-t2967))).*7.35522e-1).*(-1.0./4.0);
t15481 = (t8979.*(t13145+t17.*(t8963+t7.*(t5026+t5.*(t2959-t2967))).*7.35522e-1))./4.0;
t15485 = (t12279.*t13915)./4.0;
t15487 = -t15486;
t15491 = -t15489;
t15493 = (t12279.*t13974)./4.0;
t15497 = (t10936.*t14380)./4.0;
t15498 = -t15494;
t15504 = -t15503;
t15505 = t14380.*(t6472-t9256).*(-1.0./4.0);
t15510 = (t10973.*t14380)./4.0;
t15512 = t14380.*(t8219-t8226).*(-1.0./4.0);
t15518 = t13879.*(t10384+t16.*(t4542-t6448).*1.666555).*(-1.0./4.0);
t15519 = (t13879.*(t10384+t16.*(t4542-t6448).*1.666555))./4.0;
t15520 = (t12503.*t13876)./4.0;
t15524 = (t12279.*t14035)./4.0;
t15539 = (t12279.*t14113)./4.0;
t15542 = t12500.*(t3625+t3660+t9166-t11658).*(-1.0./4.0);
t15544 = (t12500.*(t3625+t3660+t9166-t11658))./4.0;
t15546 = -t15545;
t15547 = (t12307.*t14112)./4.0;
t15568 = t14057.*(t10384+t16.*(t4542-t6448).*1.666555).*(-1.0./4.0);
t15570 = (t10384+t16.*(t4542-t6448).*1.666555).*(-t1476+t2165+t13876).*(-1.0./4.0);
t15571 = (t10469.*t14752)./4.0;
t15572 = (t14057.*(t10384+t16.*(t4542-t6448).*1.666555))./4.0;
t15573 = ((t10384+t16.*(t4542-t6448).*1.666555).*(-t1476+t2165+t13876))./4.0;
t15577 = (t12503.*t14057)./4.0;
t15578 = (t12503.*(-t1476+t2165+t13876))./4.0;
t15587 = t12279.*(t4401+t4424+t9457-t11860).*(-1.0./4.0);
t15588 = (t12279.*(t4401+t4424+t9457-t11860))./4.0;
t15595 = t11470.*(t2189+t2495+t2635+t2646+t3580+t9.*(t258+t2289+t5392+t7559)+t17.*(t7693+t9904)).*(-1.0./4.0);
t15596 = t10149.*(t3471+t3796+t3914+t3942+t4358+t9.*(t258+t2289+t5392+t7559).*7.35522e-1+t17.*(t7693+t9904).*7.35522e-1).*(-1.0./4.0);
t15605 = (t10149.*t14919)./4.0;
t15606 = (t11470.*t14542)./4.0;
t15622 = (t12279.*t14380)./4.0;
t15623 = (t12279.*(-t3045+t3539+t14113))./4.0;
t15626 = t14380.*(t10158+t16.*(t4542-t6448)).*(-1.0./4.0);
t15628 = (t14380.*(t10158+t16.*(t4542-t6448)))./4.0;
t15631 = (t12296.*t14380)./4.0;
t15634 = ((t10378+t16.*(t4542-t6448).*7.35522e-1).*(t249-t391.*(1.1e+1./1.25e+2)-t1912.*4.252e-3+t3505+t13496+t693.*(t71-t391)+t784.*(t71-t391)))./4.0;
t15635 = -t15632;
t15637 = (t12307.*t14380)./4.0;
t15638 = (t12307.*(-t3045+t3539+t14113))./4.0;
t15640 = t12500.*(t249-t391.*(1.1e+1./1.25e+2)-t1912.*4.252e-3+t3505+t13496+t693.*(t71-t391)+t784.*(t71-t391)).*(-1.0./4.0);
t15649 = t10149.*(-t3823+t3970+t11861+t8.*t11864+t972.*(t71-t391)+t2777.*(t71-t391)).*(-1.0./4.0);
t15652 = t14380.*(t1292+t2073+t2694+t11671).*(-1.0./2.0);
t15653 = (t14380.*(t1292+t2073+t2694+t11671))./2.0;
t15668 = t11470.*(-t2550+t2696+t2698+t11659+t8.*t11672+t147.*(t71-t391)).*(-1.0./4.0);
t15673 = (t10149.*t15156)./4.0;
t15676 = (t11470.*t14823)./4.0;
t15687 = -t15686;
t15696 = (t12667.*t14380)./2.0;
t15709 = -t15707;
t15710 = -t15708;
t15722 = (t12860.*t14380)./2.0;
t15725 = -t15724;
t15734 = t12279.*(t1589-t2213-t4346+t4355+t9454+t11863+t2772.*(t71-t391)+t2775.*(t71-t391)).*(-1.0./4.0);
t15735 = (t12279.*(t1589-t2213-t4346+t4355+t9454+t11863+t2772.*(t71-t391)+t2775.*(t71-t391)))./4.0;
t15737 = -t15736;
t15739 = t12307.*(t1589-t2213-t4346+t4355+t9454+t11863+t2772.*(t71-t391)+t2775.*(t71-t391)).*(-1.0./4.0);
t15740 = (t12307.*(t1589-t2213-t4346+t4355+t9454+t11863+t2772.*(t71-t391)+t2775.*(t71-t391)))./4.0;
t15745 = (t13005.*t14380)./2.0;
t15748 = (t13019.*t14380)./2.0;
t15809 = t9926.*(t1987-t2621+t3452+t11654+t9.*(t71-t391).*6.1597e-2+t17.*(t426-t581)+t9.*(t9166-t11658)).*(-1.0./4.0);
t15811 = (t9926.*(t1987-t2621+t3452+t11654+t9.*(t71-t391).*6.1597e-2+t17.*(t426-t581)+t9.*(t9166-t11658)))./4.0;
t15814 = -t15813;
t15822 = t10149.*(t4324+t11855+t9.*(t71-t391).*4.5305948634e-2+t17.*(t426-t581).*7.35522e-1+t9.*(t9166-t11658).*7.35522e-1).*(-1.0./4.0);
t15825 = (t10149.*(t4324+t11855+t9.*(t71-t391).*4.5305948634e-2+t17.*(t426-t581).*7.35522e-1+t9.*(t9166-t11658).*7.35522e-1))./4.0;
t15839 = (t13876.*t14380)./2.0;
t15865 = t11470.*(t3452+t11654+t9.*(t71-t391).*6.1597e-2+t17.*(t426-t581)+t9.*(t9166-t11658)).*(-1.0./4.0);
t15866 = (t11470.*(t3452+t11654+t9.*(t71-t391).*6.1597e-2+t17.*(t426-t581)+t9.*(t9166-t11658)))./4.0;
t15869 = t14161.*(t10403+t9.*(t10158+t16.*(t4542-t6448)).*7.35522e-1).*(-1.0./4.0);
t15870 = (t14161.*(t10403+t9.*(t10158+t16.*(t4542-t6448)).*7.35522e-1))./4.0;
t15896 = ((t10403+t9.*(t10158+t16.*(t4542-t6448)).*7.35522e-1).*(t2148+t2513+t2649+t2661+t3582+t11950+t17.*(t258+t2289+t5392+t7559)))./4.0;
t15897 = t14541.*(t10403+t9.*(t10158+t16.*(t4542-t6448)).*7.35522e-1).*(-1.0./4.0);
t15907 = t17.*t12279.*(t2091+t2497+t2579+t2680+t3516+t9.*(t210+t2107+t7423+t9121)+t17.*(t9166-t11658)).*(-1.838805e-1);
t15908 = t9.*t12279.*(t1987-t2621+t3452+t11654+t9.*(t71-t391).*6.1597e-2+t17.*(t426-t581)+t9.*(t9166-t11658)).*(-1.838805e-1);
t15909 = t17.*t12279.*(t2091+t2497+t2579+t2680+t3516+t9.*(t210+t2107+t7423+t9121)+t17.*(t9166-t11658)).*1.838805e-1;
t15910 = t9.*t12279.*(t1987-t2621+t3452+t11654+t9.*(t71-t391).*6.1597e-2+t17.*(t426-t581)+t9.*(t9166-t11658)).*1.838805e-1;
t15916 = t12520.*(t1987-t2621+t3452+t11654+t9.*(t71-t391).*6.1597e-2+t17.*(t426-t581)+t9.*(t9166-t11658)).*(-1.0./4.0);
t15925 = ((t10403+t9.*(t10158+t16.*(t4542-t6448)).*7.35522e-1).*(t13026+t17.*(t8963+t7.*(t5026+t5.*(t2959-t2967)))))./4.0;
t15926 = ((t10174+t9.*(t10158+t16.*(t4542-t6448))).*(t13145+t17.*(t8963+t7.*(t5026+t5.*(t2959-t2967))).*7.35522e-1))./4.0;
t15928 = t14770.*(t10403+t9.*(t10158+t16.*(t4542-t6448)).*7.35522e-1).*(-1.0./4.0);
t15930 = (t14770.*(t10403+t9.*(t10158+t16.*(t4542-t6448)).*7.35522e-1))./4.0;
t15951 = t14821.*(t10403+t9.*(t10158+t16.*(t4542-t6448)).*7.35522e-1).*(-1.0./4.0);
t15954 = (t14821.*(t10403+t9.*(t10158+t16.*(t4542-t6448)).*7.35522e-1))./4.0;
t15965 = t12987.*(t1987-t2621+t3452+t11654+t9.*(t71-t391).*6.1597e-2+t17.*(t426-t581)+t9.*(t9166-t11658)).*(-1.0./4.0);
t15966 = t17.*t12279.*(t3423+t3845+t3888+t3925+t4339+t9.*(t210+t2107+t7423+t9121).*7.35522e-1+t17.*(t9166-t11658).*7.35522e-1).*(-1.0./4.0);
t15967 = (t17.*t12279.*(t3423+t3845+t3888+t3925+t4339+t9.*(t210+t2107+t7423+t9121).*7.35522e-1+t17.*(t9166-t11658).*7.35522e-1))./4.0;
t15968 = t9.*t12279.*(t3418-t3879+t4324+t11855+t9.*(t71-t391).*4.5305948634e-2+t17.*(t426-t581).*7.35522e-1+t9.*(t9166-t11658).*7.35522e-1).*(-1.0./4.0);
t15969 = (t9.*t12279.*(t3418-t3879+t4324+t11855+t9.*(t71-t391).*4.5305948634e-2+t17.*(t426-t581).*7.35522e-1+t9.*(t9166-t11658).*7.35522e-1))./4.0;
t16001 = t13382.*(t2091+t2497+t2579+t2680+t3516+t9.*(t210+t2107+t7423+t9121)+t17.*(t9166-t11658)).*(-1.0./4.0);
t16002 = (t13382.*(t2091+t2497+t2579+t2680+t3516+t9.*(t210+t2107+t7423+t9121)+t17.*(t9166-t11658)))./4.0;
t16004 = t13387.*(t2091+t2497+t2579+t2680+t3516+t9.*(t210+t2107+t7423+t9121)+t17.*(t9166-t11658)).*(-1.0./4.0);
t16005 = (t13387.*(t2091+t2497+t2579+t2680+t3516+t9.*(t210+t2107+t7423+t9121)+t17.*(t9166-t11658)))./4.0;
t16006 = t13391.*(t1987-t2621+t3452+t11654+t9.*(t71-t391).*6.1597e-2+t17.*(t426-t581)+t9.*(t9166-t11658)).*(-1.0./4.0);
t16007 = (t13391.*(t1987-t2621+t3452+t11654+t9.*(t71-t391).*6.1597e-2+t17.*(t426-t581)+t9.*(t9166-t11658)))./4.0;
t16010 = t12689.*(t3418-t3879+t4324+t11855+t9.*(t71-t391).*4.5305948634e-2+t17.*(t426-t581).*7.35522e-1+t9.*(t9166-t11658).*7.35522e-1).*(-1.0./4.0);
t16011 = t12705.*(t3423+t3845+t3888+t3925+t4339+t9.*(t210+t2107+t7423+t9121).*7.35522e-1+t17.*(t9166-t11658).*7.35522e-1).*(-1.0./4.0);
t16024 = t13181.*(t3418-t3879+t4324+t11855+t9.*(t71-t391).*4.5305948634e-2+t17.*(t426-t581).*7.35522e-1+t9.*(t9166-t11658).*7.35522e-1).*(-1.0./4.0);
t16028 = ((t10403+t9.*(t10158+t16.*(t4542-t6448)).*7.35522e-1).*(t2497+t2680+t3516+t9.*(t210+t2107+t7423+t9121)+t17.*(t9166-t11658)))./4.0;
t16042 = ((t10403+t9.*(t10158+t16.*(t4542-t6448)).*7.35522e-1).*(t2091+t2497+t2579+t2680+t3516+t9.*(t210+t2107+t7423+t9121)+t17.*(t9166-t11658)))./4.0;
t16044 = ((t10403+t9.*(t10158+t16.*(t4542-t6448)).*7.35522e-1).*(t1987-t2621+t3452+t11654+t9.*(t71-t391).*6.1597e-2+t17.*(t426-t581)+t9.*(t9166-t11658)))./4.0;
t16052 = t14411.*(t2091+t2497+t2579+t2680+t3516+t9.*(t210+t2107+t7423+t9121)+t17.*(t9166-t11658)).*(-1.0./2.0);
t16056 = t14161.*(t3418-t3879+t4324+t11855+t9.*(t71-t391).*4.5305948634e-2+t17.*(t426-t581).*7.35522e-1+t9.*(t9166-t11658).*7.35522e-1).*(-1.0./2.0);
t16057 = (t14161.*(t3418-t3879+t4324+t11855+t9.*(t71-t391).*4.5305948634e-2+t17.*(t426-t581).*7.35522e-1+t9.*(t9166-t11658).*7.35522e-1))./2.0;
t16063 = -t16061;
t16064 = -t16062;
t16078 = ((t13145+t17.*(t8963+t7.*(t5026+t5.*(t2959-t2967))).*7.35522e-1).*(t1987-t2621+t3452+t11654+t9.*(t71-t391).*6.1597e-2+t17.*(t426-t581)+t9.*(t9166-t11658)))./2.0;
t16093 = t14752.*(t3423+t3845+t3888+t3925+t4339+t9.*(t210+t2107+t7423+t9121).*7.35522e-1+t17.*(t9166-t11658).*7.35522e-1).*(-1.0./2.0);
t16094 = (t14752.*(t3423+t3845+t3888+t3925+t4339+t9.*(t210+t2107+t7423+t9121).*7.35522e-1+t17.*(t9166-t11658).*7.35522e-1))./2.0;
t16104 = t5852+t5869+t6019+t7074+t7144+t9630+t10058+t10212+t10221+t10613+t10615;
t16127 = t3246+t3276+t4043+t4076+t4093+t4101+t4123+t4128+t4149+t4198+t4216+t4236+t4249+t4331+t4978+t5041+t5621+t5690+t5707+t6690+t6820+t7535+t8202+t8239+t8263+t8361+t8397+t8408+t8892+t8895+t9229+t9634+t9663;
t16129 = q3d.*t16128;
t16131 = q3d.*t16130;
t16138 = t3755+t3777+t3804+t3826+t3854+t3858+t4158+t4161+t4187+t4272+t4394+t4404+t5556+t5578+t5705+t5711+t5764+t5786+t6240+t6265+t6832+t7043+t9271+t9490+t9497+t9498+t9633+t9647+t9688+t9721+t9920+t9944+t10163+t10198;
t16160 = q3d.*t16159;
t16162 = t4205+t4237+t4290+t4348+t4354+t4488+t4659+t4688+t5055+t5068+t5558+t5588+t5995+t6268+t6327+t6534+t6544+t6612+t7319+t7451+t7855+t7900+t9960+t10359+t10553+t11202+t11223+t11275+t11297+t11309+t11555+t11594+t11632+t11638;
t16168 = q3d.*t16167;
t16169 = t3704+t3711+t3930+t3971+t3976+t3993+t4002+t4015+t4070+t4083+t4138+t4151+t4177+t4865+t4872+t4888+t4941+t4967+t5039+t5383+t5407+t5617+t5633+t5670+t5708+t5726+t5969+t5989+t6007+t6089+t6204+t6206+t6495+t6496+t6689+t6742+t6796+t6959+t6979+t7040+t7200+t7409+t7413+t7430+t7614+t8048+t8275+t8300+t8317+t8439+t8783+t8787+t8939+t8955+t9013+t9015+t9021+t9164+t9240+t9928+t9932;
t16180 = t3775+t3786+t3810+t3920+t4046+t4050+t4091+t4106+t4132+t4182+t4207+t4240+t4247+t4891+t4926+t4971+t5056+t5175+t5372+t5398+t5435+t5678+t5816+t5817+t6021+t6040+t6076+t6086+t6176+t6705+t6737+t6766+t6881+t6882+t7297+t7298+t7325+t7333+t7431+t7447+t7695+t7716+t7729+t7766+t7770+t7775+t8247+t8489+t8744+t9023+t9032+t9191+t9282+t9287+t9472+t9487+t9501+t9516+t9517+t9646+t9671+t9683+t10139+t10140;
